simulink model "new_model"  (R2023a)
(part 1 of 4)
settings: Solver=VariableStepAuto  StartTime=0.0  StopTime=10.0  RelTol=1e-3
settings Model: Creator=owner  LastModifiedBy=owner

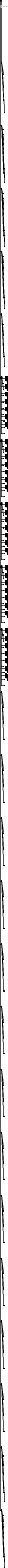
== system new_model ==
  SensorsInput : Inport
  Bus Selector:FreeSpacePerception:0 : BusSelector  OutputSignals=FreeSpacePerception:0.time,FreeSpacePerception:0.width,FreeSpacePerception:0.x,FreeSpacePerception:0.y
  Bus Selector:GNSS:0 : BusSelector  OutputSignals=GNSS:0.Timestamp,GNSS:0.Longitude,GNSS:0.Latitude,GNSS:0.Altitude,GNSS:0.Heading,GNSS:0.Velocity
  Bus Selector:IMU:0 : BusSelector  OutputSignals=IMU:0.Timestamp,IMU:0.ACC_X,IMU:0.ACC_Y,IMU:0.ACC_Z,IMU:0.Gyro_X,IMU:0.Gyro_Y,IMU:0.Gyro_Z,IMU:0.Yaw,IMU:0.Pitch,IMU:0.Roll
  Bus Selector:LaneInfoPerception:0 : BusSelector  OutputSignals=LaneInfoPerception:0.Timestamp,LaneInfoPerception:0.width,LaneInfoPerception:0.Lane_ID,LaneInfoPerception:0.Lane_Distance,LaneInfoPerception:0.Lane_Car_Distance_Left,LaneInfoPerception:0.Lane_Car_Distance_Right,LaneInfoPerception:0.Lane_Curvature,LaneInfoPerception:0.Lane_Coefficient_C0,LaneInfoPerception:0.Lane_Coefficient_C1,LaneInfoPerception:0.Lane_Coefficient_C2,LaneInfoPerception:0.Lane_Coefficient_C3,LaneInfoPerception:0.Lane_Class
  Bus Selector:ObjectPerception:0 : BusSelector  OutputSignals=ObjectPerception:0.Timestamp,ObjectPerception:0.width,ObjectPerception:0.OBJ_ID,ObjectPerception:0.OBJ_Class,ObjectPerception:0.OBJ_X,ObjectPerception:0.OBJ_Y,ObjectPerception:0.OBJ_Z,ObjectPerception:0.OBJ_Velocity,ObjectPerception:0.OBJ_Length,ObjectPerception:0.OBJ_Width,ObjectPerception:0.OBJ_Height
  Bus Selector:ParkingLotsPerception:0 : BusSelector  OutputSignals=ParkingLotsPerception:0.time,ParkingLotsPerception:0.width,ParkingLotsPerception:0.x1,ParkingLotsPerception:0.y1,ParkingLotsPerception:0.x2,ParkingLotsPerception:0.y2,ParkingLotsPerception:0.x3,ParkingLotsPerception:0.y3,ParkingLotsPerception:0.x4,ParkingLotsPerception:0.y4
  Bus Selector:RadarSensor:0 : BusSelector  OutputSignals=RadarSensor:0.time,RadarSensor:0.width,RadarSensor:0.OBJ_ID,RadarSensor:0.OBJ_Class,RadarSensor:0.OBJ_S_Azimuth,RadarSensor:0.OBJ_S_Elevation,RadarSensor:0.OBJ_S_Velocity,RadarSensor:0.OBJ_S_Range,RadarSensor:0.OBJ_RCS
  Bus Selector:RadarSensor:0_OBJ_Class_BS : BusSelector  OutputSignals=RadarSensor:0.OBJ_Class_1,RadarSensor:0.OBJ_Class_2,RadarSensor:0.OBJ_Class_3,RadarSensor:0.OBJ_Class_4,RadarSensor:0.OBJ_Class_5,RadarSensor:0.OBJ_Class_6,RadarSensor:0.OBJ_Class_7,RadarSensor:0.OBJ_Class_8,RadarSensor:0.OBJ_Class_9,RadarSensor:0.OBJ_Class_10,RadarSensor:0.OBJ_Class_11,RadarSensor:0.OBJ_Class_12,RadarSensor:0.OBJ_Class_13,RadarSensor:0.OBJ_Class_14,RadarSensor:0.OBJ_Class_15,RadarSensor:0.OBJ_Class_16,RadarSensor:0.OBJ_Class_17,RadarSensor:0.OBJ_Class_18,RadarSensor:0.OBJ_Class_19,RadarSensor:0.OBJ_Class_20,RadarSensor:0.OBJ_Class_21,RadarSensor:0.OBJ_Class_22,RadarSensor:0.OBJ_Class_23,RadarSensor:0.OBJ_Class_24,RadarSensor:0.OBJ_Class_25,RadarSensor:0.OBJ_Class_26,RadarSensor:0.OBJ_Class_27,RadarSensor:0.OBJ_Class_28,RadarSensor:0.OBJ_Class_29,RadarSensor:0.OBJ_Class_30,RadarSensor:0.OBJ_Class_31,RadarSensor:0.OBJ_Class_32,RadarSensor:0.OBJ_Class_33,RadarSensor:0.OBJ_Class_34,RadarSensor:0.OBJ_Class_35,RadarSensor:0.OBJ_Class_36,RadarSensor:0.OBJ_Class_37,RadarSensor:0.OBJ_Class_38,RadarSensor:0.OBJ_Class_39,RadarSensor:0.OBJ_Class_40,RadarSensor:0.OBJ_Class_41,RadarSensor:0.OBJ_Class_42,RadarSensor:0.OBJ_Class_43,RadarSensor:0.OBJ_Class_44,RadarSensor:0.OBJ_Class_45,RadarSensor:0.OBJ_Class_46,RadarSensor:0.OBJ_Class_47,RadarSensor:0.OBJ_Class_48,RadarSensor:0.OBJ_Class_49,RadarSensor:0.OBJ_Class_50,RadarSensor:0.OBJ_Class_51,RadarSensor:0.OBJ_Class_52,RadarSensor:0.OBJ_Class_53,RadarSensor:0.OBJ_Class_54,RadarSensor:0.OBJ_Class_55,RadarSensor:0.OBJ_Class_56,RadarSensor:0.OBJ_Class_57,RadarSensor:0.OBJ_Class_58,RadarSensor:0.OBJ_Class_59,RadarSensor:0.OBJ_Class_60,RadarSensor:0.OBJ_Class_61,RadarSensor:0.OBJ_Class_62,RadarSensor:0.OBJ_Class_63,RadarSensor:0.OBJ_Class_64
  Bus Selector:RadarSensor:0_OBJ_ID_BS : BusSelector  OutputSignals=RadarSensor:0.OBJ_ID_1,RadarSensor:0.OBJ_ID_2,RadarSensor:0.OBJ_ID_3,RadarSensor:0.OBJ_ID_4,RadarSensor:0.OBJ_ID_5,RadarSensor:0.OBJ_ID_6,RadarSensor:0.OBJ_ID_7,RadarSensor:0.OBJ_ID_8,RadarSensor:0.OBJ_ID_9,RadarSensor:0.OBJ_ID_10,RadarSensor:0.OBJ_ID_11,RadarSensor:0.OBJ_ID_12,RadarSensor:0.OBJ_ID_13,RadarSensor:0.OBJ_ID_14,RadarSensor:0.OBJ_ID_15,RadarSensor:0.OBJ_ID_16,RadarSensor:0.OBJ_ID_17,RadarSensor:0.OBJ_ID_18,RadarSensor:0.OBJ_ID_19,RadarSensor:0.OBJ_ID_20,RadarSensor:0.OBJ_ID_21,RadarSensor:0.OBJ_ID_22,RadarSensor:0.OBJ_ID_23,RadarSensor:0.OBJ_ID_24,RadarSensor:0.OBJ_ID_25,RadarSensor:0.OBJ_ID_26,RadarSensor:0.OBJ_ID_27,RadarSensor:0.OBJ_ID_28,RadarSensor:0.OBJ_ID_29,RadarSensor:0.OBJ_ID_30,RadarSensor:0.OBJ_ID_31,RadarSensor:0.OBJ_ID_32,RadarSensor:0.OBJ_ID_33,RadarSensor:0.OBJ_ID_34,RadarSensor:0.OBJ_ID_35,RadarSensor:0.OBJ_ID_36,RadarSensor:0.OBJ_ID_37,RadarSensor:0.OBJ_ID_38,RadarSensor:0.OBJ_ID_39,RadarSensor:0.OBJ_ID_40,RadarSensor:0.OBJ_ID_41,RadarSensor:0.OBJ_ID_42,RadarSensor:0.OBJ_ID_43,RadarSensor:0.OBJ_ID_44,RadarSensor:0.OBJ_ID_45,RadarSensor:0.OBJ_ID_46,RadarSensor:0.OBJ_ID_47,RadarSensor:0.OBJ_ID_48,RadarSensor:0.OBJ_ID_49,RadarSensor:0.OBJ_ID_50,RadarSensor:0.OBJ_ID_51,RadarSensor:0.OBJ_ID_52,RadarSensor:0.OBJ_ID_53,RadarSensor:0.OBJ_ID_54,RadarSensor:0.OBJ_ID_55,RadarSensor:0.OBJ_ID_56,RadarSensor:0.OBJ_ID_57,RadarSensor:0.OBJ_ID_58,RadarSensor:0.OBJ_ID_59,RadarSensor:0.OBJ_ID_60,RadarSensor:0.OBJ_ID_61,RadarSensor:0.OBJ_ID_62,RadarSensor:0.OBJ_ID_63,RadarSensor:0.OBJ_ID_64
  Bus Selector:RadarSensor:0_OBJ_RCS_BS : BusSelector  OutputSignals=RadarSensor:0.OBJ_RCS_1,RadarSensor:0.OBJ_RCS_2,RadarSensor:0.OBJ_RCS_3,RadarSensor:0.OBJ_RCS_4,RadarSensor:0.OBJ_RCS_5,RadarSensor:0.OBJ_RCS_6,RadarSensor:0.OBJ_RCS_7,RadarSensor:0.OBJ_RCS_8,RadarSensor:0.OBJ_RCS_9,RadarSensor:0.OBJ_RCS_10,RadarSensor:0.OBJ_RCS_11,RadarSensor:0.OBJ_RCS_12,RadarSensor:0.OBJ_RCS_13,RadarSensor:0.OBJ_RCS_14,RadarSensor:0.OBJ_RCS_15,RadarSensor:0.OBJ_RCS_16,RadarSensor:0.OBJ_RCS_17,RadarSensor:0.OBJ_RCS_18,RadarSensor:0.OBJ_RCS_19,RadarSensor:0.OBJ_RCS_20,RadarSensor:0.OBJ_RCS_21,RadarSensor:0.OBJ_RCS_22,RadarSensor:0.OBJ_RCS_23,RadarSensor:0.OBJ_RCS_24,RadarSensor:0.OBJ_RCS_25,RadarSensor:0.OBJ_RCS_26,RadarSensor:0.OBJ_RCS_27,RadarSensor:0.OBJ_RCS_28,RadarSensor:0.OBJ_RCS_29,RadarSensor:0.OBJ_RCS_30,RadarSensor:0.OBJ_RCS_31,RadarSensor:0.OBJ_RCS_32,RadarSensor:0.OBJ_RCS_33,RadarSensor:0.OBJ_RCS_34,RadarSensor:0.OBJ_RCS_35,RadarSensor:0.OBJ_RCS_36,RadarSensor:0.OBJ_RCS_37,RadarSensor:0.OBJ_RCS_38,RadarSensor:0.OBJ_RCS_39,RadarSensor:0.OBJ_RCS_40,RadarSensor:0.OBJ_RCS_41,RadarSensor:0.OBJ_RCS_42,RadarSensor:0.OBJ_RCS_43,RadarSensor:0.OBJ_RCS_44,RadarSensor:0.OBJ_RCS_45,RadarSensor:0.OBJ_RCS_46,RadarSensor:0.OBJ_RCS_47,RadarSensor:0.OBJ_RCS_48,RadarSensor:0.OBJ_RCS_49,RadarSensor:0.OBJ_RCS_50,RadarSensor:0.OBJ_RCS_51,RadarSensor:0.OBJ_RCS_52,RadarSensor:0.OBJ_RCS_53,RadarSensor:0.OBJ_RCS_54,RadarSensor:0.OBJ_RCS_55,RadarSensor:0.OBJ_RCS_56,RadarSensor:0.OBJ_RCS_57,RadarSensor:0.OBJ_RCS_58,RadarSensor:0.OBJ_RCS_59,RadarSensor:0.OBJ_RCS_60,RadarSensor:0.OBJ_RCS_61,RadarSensor:0.OBJ_RCS_62,RadarSensor:0.OBJ_RCS_63,RadarSensor:0.OBJ_RCS_64
  Bus Selector:RadarSensor:0_OBJ_S_Azimuth_BS : BusSelector  OutputSignals=RadarSensor:0.OBJ_S_Azimuth_1,RadarSensor:0.OBJ_S_Azimuth_2,RadarSensor:0.OBJ_S_Azimuth_3,RadarSensor:0.OBJ_S_Azimuth_4,RadarSensor:0.OBJ_S_Azimuth_5,RadarSensor:0.OBJ_S_Azimuth_6,RadarSensor:0.OBJ_S_Azimuth_7,RadarSensor:0.OBJ_S_Azimuth_8,RadarSensor:0.OBJ_S_Azimuth_9,RadarSensor:0.OBJ_S_Azimuth_10,RadarSensor:0.OBJ_S_Azimuth_11,RadarSensor:0.OBJ_S_Azimuth_12,RadarSensor:0.OBJ_S_Azimuth_13,RadarSensor:0.OBJ_S_Azimuth_14,RadarSensor:0.OBJ_S_Azimuth_15,RadarSensor:0.OBJ_S_Azimuth_16,RadarSensor:0.OBJ_S_Azimuth_17,RadarSensor:0.OBJ_S_Azimuth_18,RadarSensor:0.OBJ_S_Azimuth_19,RadarSensor:0.OBJ_S_Azimuth_20,RadarSensor:0.OBJ_S_Azimuth_21,RadarSensor:0.OBJ_S_Azimuth_22,RadarSensor:0.OBJ_S_Azimuth_23,RadarSensor:0.OBJ_S_Azimuth_24,RadarSensor:0.OBJ_S_Azimuth_25,RadarSensor:0.OBJ_S_Azimuth_26,RadarSensor:0.OBJ_S_Azimuth_27,RadarSensor:0.OBJ_S_Azimuth_28,RadarSensor:0.OBJ_S_Azimuth_29,RadarSensor:0.OBJ_S_Azimuth_30,RadarSensor:0.OBJ_S_Azimuth_31,RadarSensor:0.OBJ_S_Azimuth_32,RadarSensor:0.OBJ_S_Azimuth_33,RadarSensor:0.OBJ_S_Azimuth_34,RadarSensor:0.OBJ_S_Azimuth_35,RadarSensor:0.OBJ_S_Azimuth_36,RadarSensor:0.OBJ_S_Azimuth_37,RadarSensor:0.OBJ_S_Azimuth_38,RadarSensor:0.OBJ_S_Azimuth_39,RadarSensor:0.OBJ_S_Azimuth_40,RadarSensor:0.OBJ_S_Azimuth_41,RadarSensor:0.OBJ_S_Azimuth_42,RadarSensor:0.OBJ_S_Azimuth_43,RadarSensor:0.OBJ_S_Azimuth_44,RadarSensor:0.OBJ_S_Azimuth_45,RadarSensor:0.OBJ_S_Azimuth_46,RadarSensor:0.OBJ_S_Azimuth_47,RadarSensor:0.OBJ_S_Azimuth_48,RadarSensor:0.OBJ_S_Azimuth_49,RadarSensor:0.OBJ_S_Azimuth_50,RadarSensor:0.OBJ_S_Azimuth_51,RadarSensor:0.OBJ_S_Azimuth_52,RadarSensor:0.OBJ_S_Azimuth_53,RadarSensor:0.OBJ_S_Azimuth_54,RadarSensor:0.OBJ_S_Azimuth_55,RadarSensor:0.OBJ_S_Azimuth_56,RadarSensor:0.OBJ_S_Azimuth_57,RadarSensor:0.OBJ_S_Azimuth_58,RadarSensor:0.OBJ_S_Azimuth_59,RadarSensor:0.OBJ_S_Azimuth_60,RadarSensor:0.OBJ_S_Azimuth_61,RadarSensor:0.OBJ_S_Azimuth_62,RadarSensor:0.OBJ_S_Azimuth_63,RadarSensor:0.OBJ_S_Azimuth_64
  Bus Selector:RadarSensor:0_OBJ_S_Elevation_BS : BusSelector  OutputSignals=RadarSensor:0.OBJ_S_Elevation_1,RadarSensor:0.OBJ_S_Elevation_2,RadarSensor:0.OBJ_S_Elevation_3,RadarSensor:0.OBJ_S_Elevation_4,RadarSensor:0.OBJ_S_Elevation_5,RadarSensor:0.OBJ_S_Elevation_6,RadarSensor:0.OBJ_S_Elevation_7,RadarSensor:0.OBJ_S_Elevation_8,RadarSensor:0.OBJ_S_Elevation_9,RadarSensor:0.OBJ_S_Elevation_10,RadarSensor:0.OBJ_S_Elevation_11,RadarSensor:0.OBJ_S_Elevation_12,RadarSensor:0.OBJ_S_Elevation_13,RadarSensor:0.OBJ_S_Elevation_14,RadarSensor:0.OBJ_S_Elevation_15,RadarSensor:0.OBJ_S_Elevation_16,RadarSensor:0.OBJ_S_Elevation_17,RadarSensor:0.OBJ_S_Elevation_18,RadarSensor:0.OBJ_S_Elevation_19,RadarSensor:0.OBJ_S_Elevation_20,RadarSensor:0.OBJ_S_Elevation_21,RadarSensor:0.OBJ_S_Elevation_22,RadarSensor:0.OBJ_S_Elevation_23,RadarSensor:0.OBJ_S_Elevation_24,RadarSensor:0.OBJ_S_Elevation_25,RadarSensor:0.OBJ_S_Elevation_26,RadarSensor:0.OBJ_S_Elevation_27,RadarSensor:0.OBJ_S_Elevation_28,RadarSensor:0.OBJ_S_Elevation_29,RadarSensor:0.OBJ_S_Elevation_30,RadarSensor:0.OBJ_S_Elevation_31,RadarSensor:0.OBJ_S_Elevation_32,RadarSensor:0.OBJ_S_Elevation_33,RadarSensor:0.OBJ_S_Elevation_34,RadarSensor:0.OBJ_S_Elevation_35,RadarSensor:0.OBJ_S_Elevation_36,RadarSensor:0.OBJ_S_Elevation_37,RadarSensor:0.OBJ_S_Elevation_38,RadarSensor:0.OBJ_S_Elevation_39,RadarSensor:0.OBJ_S_Elevation_40,RadarSensor:0.OBJ_S_Elevation_41,RadarSensor:0.OBJ_S_Elevation_42,RadarSensor:0.OBJ_S_Elevation_43,RadarSensor:0.OBJ_S_Elevation_44,RadarSensor:0.OBJ_S_Elevation_45,RadarSensor:0.OBJ_S_Elevation_46,RadarSensor:0.OBJ_S_Elevation_47,RadarSensor:0.OBJ_S_Elevation_48,RadarSensor:0.OBJ_S_Elevation_49,RadarSensor:0.OBJ_S_Elevation_50,RadarSensor:0.OBJ_S_Elevation_51,RadarSensor:0.OBJ_S_Elevation_52,RadarSensor:0.OBJ_S_Elevation_53,RadarSensor:0.OBJ_S_Elevation_54,RadarSensor:0.OBJ_S_Elevation_55,RadarSensor:0.OBJ_S_Elevation_56,RadarSensor:0.OBJ_S_Elevation_57,RadarSensor:0.OBJ_S_Elevation_58,RadarSensor:0.OBJ_S_Elevation_59,RadarSensor:0.OBJ_S_Elevation_60,RadarSensor:0.OBJ_S_Elevation_61,RadarSensor:0.OBJ_S_Elevation_62,RadarSensor:0.OBJ_S_Elevation_63,RadarSensor:0.OBJ_S_Elevation_64
  Bus Selector:RadarSensor:0_OBJ_S_Range_BS : BusSelector  OutputSignals=RadarSensor:0.OBJ_S_Range_1,RadarSensor:0.OBJ_S_Range_2,RadarSensor:0.OBJ_S_Range_3,RadarSensor:0.OBJ_S_Range_4,RadarSensor:0.OBJ_S_Range_5,RadarSensor:0.OBJ_S_Range_6,RadarSensor:0.OBJ_S_Range_7,RadarSensor:0.OBJ_S_Range_8,RadarSensor:0.OBJ_S_Range_9,RadarSensor:0.OBJ_S_Range_10,RadarSensor:0.OBJ_S_Range_11,RadarSensor:0.OBJ_S_Range_12,RadarSensor:0.OBJ_S_Range_13,RadarSensor:0.OBJ_S_Range_14,RadarSensor:0.OBJ_S_Range_15,RadarSensor:0.OBJ_S_Range_16,RadarSensor:0.OBJ_S_Range_17,RadarSensor:0.OBJ_S_Range_18,RadarSensor:0.OBJ_S_Range_19,RadarSensor:0.OBJ_S_Range_20,RadarSensor:0.OBJ_S_Range_21,RadarSensor:0.OBJ_S_Range_22,RadarSensor:0.OBJ_S_Range_23,RadarSensor:0.OBJ_S_Range_24,RadarSensor:0.OBJ_S_Range_25,RadarSensor:0.OBJ_S_Range_26,RadarSensor:0.OBJ_S_Range_27,RadarSensor:0.OBJ_S_Range_28,RadarSensor:0.OBJ_S_Range_29,RadarSensor:0.OBJ_S_Range_30,RadarSensor:0.OBJ_S_Range_31,RadarSensor:0.OBJ_S_Range_32,RadarSensor:0.OBJ_S_Range_33,RadarSensor:0.OBJ_S_Range_34,RadarSensor:0.OBJ_S_Range_35,RadarSensor:0.OBJ_S_Range_36,RadarSensor:0.OBJ_S_Range_37,RadarSensor:0.OBJ_S_Range_38,RadarSensor:0.OBJ_S_Range_39,RadarSensor:0.OBJ_S_Range_40,RadarSensor:0.OBJ_S_Range_41,RadarSensor:0.OBJ_S_Range_42,RadarSensor:0.OBJ_S_Range_43,RadarSensor:0.OBJ_S_Range_44,RadarSensor:0.OBJ_S_Range_45,RadarSensor:0.OBJ_S_Range_46,RadarSensor:0.OBJ_S_Range_47,RadarSensor:0.OBJ_S_Range_48,RadarSensor:0.OBJ_S_Range_49,RadarSensor:0.OBJ_S_Range_50,RadarSensor:0.OBJ_S_Range_51,RadarSensor:0.OBJ_S_Range_52,RadarSensor:0.OBJ_S_Range_53,RadarSensor:0.OBJ_S_Range_54,RadarSensor:0.OBJ_S_Range_55,RadarSensor:0.OBJ_S_Range_56,RadarSensor:0.OBJ_S_Range_57,RadarSensor:0.OBJ_S_Range_58,RadarSensor:0.OBJ_S_Range_59,RadarSensor:0.OBJ_S_Range_60,RadarSensor:0.OBJ_S_Range_61,RadarSensor:0.OBJ_S_Range_62,RadarSensor:0.OBJ_S_Range_63,RadarSensor:0.OBJ_S_Range_64
  Bus Selector:RadarSensor:0_OBJ_S_Velocity_BS : BusSelector  OutputSignals=RadarSensor:0.OBJ_S_Velocity_1,RadarSensor:0.OBJ_S_Velocity_2,RadarSensor:0.OBJ_S_Velocity_3,RadarSensor:0.OBJ_S_Velocity_4,RadarSensor:0.OBJ_S_Velocity_5,RadarSensor:0.OBJ_S_Velocity_6,RadarSensor:0.OBJ_S_Velocity_7,RadarSensor:0.OBJ_S_Velocity_8,RadarSensor:0.OBJ_S_Velocity_9,RadarSensor:0.OBJ_S_Velocity_10,RadarSensor:0.OBJ_S_Velocity_11,RadarSensor:0.OBJ_S_Velocity_12,RadarSensor:0.OBJ_S_Velocity_13,RadarSensor:0.OBJ_S_Velocity_14,RadarSensor:0.OBJ_S_Velocity_15,RadarSensor:0.OBJ_S_Velocity_16,RadarSensor:0.OBJ_S_Velocity_17,RadarSensor:0.OBJ_S_Velocity_18,RadarSensor:0.OBJ_S_Velocity_19,RadarSensor:0.OBJ_S_Velocity_20,RadarSensor:0.OBJ_S_Velocity_21,RadarSensor:0.OBJ_S_Velocity_22,RadarSensor:0.OBJ_S_Velocity_23,RadarSensor:0.OBJ_S_Velocity_24,RadarSensor:0.OBJ_S_Velocity_25,RadarSensor:0.OBJ_S_Velocity_26,RadarSensor:0.OBJ_S_Velocity_27,RadarSensor:0.OBJ_S_Velocity_28,RadarSensor:0.OBJ_S_Velocity_29,RadarSensor:0.OBJ_S_Velocity_30,RadarSensor:0.OBJ_S_Velocity_31,RadarSensor:0.OBJ_S_Velocity_32,RadarSensor:0.OBJ_S_Velocity_33,RadarSensor:0.OBJ_S_Velocity_34,RadarSensor:0.OBJ_S_Velocity_35,RadarSensor:0.OBJ_S_Velocity_36,RadarSensor:0.OBJ_S_Velocity_37,RadarSensor:0.OBJ_S_Velocity_38,RadarSensor:0.OBJ_S_Velocity_39,RadarSensor:0.OBJ_S_Velocity_40,RadarSensor:0.OBJ_S_Velocity_41,RadarSensor:0.OBJ_S_Velocity_42,RadarSensor:0.OBJ_S_Velocity_43,RadarSensor:0.OBJ_S_Velocity_44,RadarSensor:0.OBJ_S_Velocity_45,RadarSensor:0.OBJ_S_Velocity_46,RadarSensor:0.OBJ_S_Velocity_47,RadarSensor:0.OBJ_S_Velocity_48,RadarSensor:0.OBJ_S_Velocity_49,RadarSensor:0.OBJ_S_Velocity_50,RadarSensor:0.OBJ_S_Velocity_51,RadarSensor:0.OBJ_S_Velocity_52,RadarSensor:0.OBJ_S_Velocity_53,RadarSensor:0.OBJ_S_Velocity_54,RadarSensor:0.OBJ_S_Velocity_55,RadarSensor:0.OBJ_S_Velocity_56,RadarSensor:0.OBJ_S_Velocity_57,RadarSensor:0.OBJ_S_Velocity_58,RadarSensor:0.OBJ_S_Velocity_59,RadarSensor:0.OBJ_S_Velocity_60,RadarSensor:0.OBJ_S_Velocity_61,RadarSensor:0.OBJ_S_Velocity_62,RadarSensor:0.OBJ_S_Velocity_63,RadarSensor:0.OBJ_S_Velocity_64
  Bus Selector:RadarSensor:1 : BusSelector  OutputSignals=RadarSensor:1.time,RadarSensor:1.width,RadarSensor:1.OBJ_ID,RadarSensor:1.OBJ_Class,RadarSensor:1.OBJ_S_Azimuth,RadarSensor:1.OBJ_S_Elevation,RadarSensor:1.OBJ_S_Velocity,RadarSensor:1.OBJ_S_Range,RadarSensor:1.OBJ_RCS
  Bus Selector:RadarSensor:1_OBJ_Class_BS : BusSelector  OutputSignals=RadarSensor:1.OBJ_Class_1,RadarSensor:1.OBJ_Class_2,RadarSensor:1.OBJ_Class_3,RadarSensor:1.OBJ_Class_4,RadarSensor:1.OBJ_Class_5,RadarSensor:1.OBJ_Class_6,RadarSensor:1.OBJ_Class_7,RadarSensor:1.OBJ_Class_8,RadarSensor:1.OBJ_Class_9,RadarSensor:1.OBJ_Class_10,RadarSensor:1.OBJ_Class_11,RadarSensor:1.OBJ_Class_12,RadarSensor:1.OBJ_Class_13,RadarSensor:1.OBJ_Class_14,RadarSensor:1.OBJ_Class_15,RadarSensor:1.OBJ_Class_16,RadarSensor:1.OBJ_Class_17,RadarSensor:1.OBJ_Class_18,RadarSensor:1.OBJ_Class_19,RadarSensor:1.OBJ_Class_20,RadarSensor:1.OBJ_Class_21,RadarSensor:1.OBJ_Class_22,RadarSensor:1.OBJ_Class_23,RadarSensor:1.OBJ_Class_24,RadarSensor:1.OBJ_Class_25,RadarSensor:1.OBJ_Class_26,RadarSensor:1.OBJ_Class_27,RadarSensor:1.OBJ_Class_28,RadarSensor:1.OBJ_Class_29,RadarSensor:1.OBJ_Class_30,RadarSensor:1.OBJ_Class_31,RadarSensor:1.OBJ_Class_32,RadarSensor:1.OBJ_Class_33,RadarSensor:1.OBJ_Class_34,RadarSensor:1.OBJ_Class_35,RadarSensor:1.OBJ_Class_36,RadarSensor:1.OBJ_Class_37,RadarSensor:1.OBJ_Class_38,RadarSensor:1.OBJ_Class_39,RadarSensor:1.OBJ_Class_40,RadarSensor:1.OBJ_Class_41,RadarSensor:1.OBJ_Class_42,RadarSensor:1.OBJ_Class_43,RadarSensor:1.OBJ_Class_44,RadarSensor:1.OBJ_Class_45,RadarSensor:1.OBJ_Class_46,RadarSensor:1.OBJ_Class_47,RadarSensor:1.OBJ_Class_48,RadarSensor:1.OBJ_Class_49,RadarSensor:1.OBJ_Class_50,RadarSensor:1.OBJ_Class_51,RadarSensor:1.OBJ_Class_52,RadarSensor:1.OBJ_Class_53,RadarSensor:1.OBJ_Class_54,RadarSensor:1.OBJ_Class_55,RadarSensor:1.OBJ_Class_56,RadarSensor:1.OBJ_Class_57,RadarSensor:1.OBJ_Class_58,RadarSensor:1.OBJ_Class_59,RadarSensor:1.OBJ_Class_60,RadarSensor:1.OBJ_Class_61,RadarSensor:1.OBJ_Class_62,RadarSensor:1.OBJ_Class_63,RadarSensor:1.OBJ_Class_64
  Bus Selector:RadarSensor:1_OBJ_ID_BS : BusSelector  OutputSignals=RadarSensor:1.OBJ_ID_1,RadarSensor:1.OBJ_ID_2,RadarSensor:1.OBJ_ID_3,RadarSensor:1.OBJ_ID_4,RadarSensor:1.OBJ_ID_5,RadarSensor:1.OBJ_ID_6,RadarSensor:1.OBJ_ID_7,RadarSensor:1.OBJ_ID_8,RadarSensor:1.OBJ_ID_9,RadarSensor:1.OBJ_ID_10,RadarSensor:1.OBJ_ID_11,RadarSensor:1.OBJ_ID_12,RadarSensor:1.OBJ_ID_13,RadarSensor:1.OBJ_ID_14,RadarSensor:1.OBJ_ID_15,RadarSensor:1.OBJ_ID_16,RadarSensor:1.OBJ_ID_17,RadarSensor:1.OBJ_ID_18,RadarSensor:1.OBJ_ID_19,RadarSensor:1.OBJ_ID_20,RadarSensor:1.OBJ_ID_21,RadarSensor:1.OBJ_ID_22,RadarSensor:1.OBJ_ID_23,RadarSensor:1.OBJ_ID_24,RadarSensor:1.OBJ_ID_25,RadarSensor:1.OBJ_ID_26,RadarSensor:1.OBJ_ID_27,RadarSensor:1.OBJ_ID_28,RadarSensor:1.OBJ_ID_29,RadarSensor:1.OBJ_ID_30,RadarSensor:1.OBJ_ID_31,RadarSensor:1.OBJ_ID_32,RadarSensor:1.OBJ_ID_33,RadarSensor:1.OBJ_ID_34,RadarSensor:1.OBJ_ID_35,RadarSensor:1.OBJ_ID_36,RadarSensor:1.OBJ_ID_37,RadarSensor:1.OBJ_ID_38,RadarSensor:1.OBJ_ID_39,RadarSensor:1.OBJ_ID_40,RadarSensor:1.OBJ_ID_41,RadarSensor:1.OBJ_ID_42,RadarSensor:1.OBJ_ID_43,RadarSensor:1.OBJ_ID_44,RadarSensor:1.OBJ_ID_45,RadarSensor:1.OBJ_ID_46,RadarSensor:1.OBJ_ID_47,RadarSensor:1.OBJ_ID_48,RadarSensor:1.OBJ_ID_49,RadarSensor:1.OBJ_ID_50,RadarSensor:1.OBJ_ID_51,RadarSensor:1.OBJ_ID_52,RadarSensor:1.OBJ_ID_53,RadarSensor:1.OBJ_ID_54,RadarSensor:1.OBJ_ID_55,RadarSensor:1.OBJ_ID_56,RadarSensor:1.OBJ_ID_57,RadarSensor:1.OBJ_ID_58,RadarSensor:1.OBJ_ID_59,RadarSensor:1.OBJ_ID_60,RadarSensor:1.OBJ_ID_61,RadarSensor:1.OBJ_ID_62,RadarSensor:1.OBJ_ID_63,RadarSensor:1.OBJ_ID_64
  Bus Selector:RadarSensor:1_OBJ_RCS_BS : BusSelector  OutputSignals=RadarSensor:1.OBJ_RCS_1,RadarSensor:1.OBJ_RCS_2,RadarSensor:1.OBJ_RCS_3,RadarSensor:1.OBJ_RCS_4,RadarSensor:1.OBJ_RCS_5,RadarSensor:1.OBJ_RCS_6,RadarSensor:1.OBJ_RCS_7,RadarSensor:1.OBJ_RCS_8,RadarSensor:1.OBJ_RCS_9,RadarSensor:1.OBJ_RCS_10,RadarSensor:1.OBJ_RCS_11,RadarSensor:1.OBJ_RCS_12,RadarSensor:1.OBJ_RCS_13,RadarSensor:1.OBJ_RCS_14,RadarSensor:1.OBJ_RCS_15,RadarSensor:1.OBJ_RCS_16,RadarSensor:1.OBJ_RCS_17,RadarSensor:1.OBJ_RCS_18,RadarSensor:1.OBJ_RCS_19,RadarSensor:1.OBJ_RCS_20,RadarSensor:1.OBJ_RCS_21,RadarSensor:1.OBJ_RCS_22,RadarSensor:1.OBJ_RCS_23,RadarSensor:1.OBJ_RCS_24,RadarSensor:1.OBJ_RCS_25,RadarSensor:1.OBJ_RCS_26,RadarSensor:1.OBJ_RCS_27,RadarSensor:1.OBJ_RCS_28,RadarSensor:1.OBJ_RCS_29,RadarSensor:1.OBJ_RCS_30,RadarSensor:1.OBJ_RCS_31,RadarSensor:1.OBJ_RCS_32,RadarSensor:1.OBJ_RCS_33,RadarSensor:1.OBJ_RCS_34,RadarSensor:1.OBJ_RCS_35,RadarSensor:1.OBJ_RCS_36,RadarSensor:1.OBJ_RCS_37,RadarSensor:1.OBJ_RCS_38,RadarSensor:1.OBJ_RCS_39,RadarSensor:1.OBJ_RCS_40,RadarSensor:1.OBJ_RCS_41,RadarSensor:1.OBJ_RCS_42,RadarSensor:1.OBJ_RCS_43,RadarSensor:1.OBJ_RCS_44,RadarSensor:1.OBJ_RCS_45,RadarSensor:1.OBJ_RCS_46,RadarSensor:1.OBJ_RCS_47,RadarSensor:1.OBJ_RCS_48,RadarSensor:1.OBJ_RCS_49,RadarSensor:1.OBJ_RCS_50,RadarSensor:1.OBJ_RCS_51,RadarSensor:1.OBJ_RCS_52,RadarSensor:1.OBJ_RCS_53,RadarSensor:1.OBJ_RCS_54,RadarSensor:1.OBJ_RCS_55,RadarSensor:1.OBJ_RCS_56,RadarSensor:1.OBJ_RCS_57,RadarSensor:1.OBJ_RCS_58,RadarSensor:1.OBJ_RCS_59,RadarSensor:1.OBJ_RCS_60,RadarSensor:1.OBJ_RCS_61,RadarSensor:1.OBJ_RCS_62,RadarSensor:1.OBJ_RCS_63,RadarSensor:1.OBJ_RCS_64
  Bus Selector:RadarSensor:1_OBJ_S_Azimuth_BS : BusSelector  OutputSignals=RadarSensor:1.OBJ_S_Azimuth_1,RadarSensor:1.OBJ_S_Azimuth_2,RadarSensor:1.OBJ_S_Azimuth_3,RadarSensor:1.OBJ_S_Azimuth_4,RadarSensor:1.OBJ_S_Azimuth_5,RadarSensor:1.OBJ_S_Azimuth_6,RadarSensor:1.OBJ_S_Azimuth_7,RadarSensor:1.OBJ_S_Azimuth_8,RadarSensor:1.OBJ_S_Azimuth_9,RadarSensor:1.OBJ_S_Azimuth_10,RadarSensor:1.OBJ_S_Azimuth_11,RadarSensor:1.OBJ_S_Azimuth_12,RadarSensor:1.OBJ_S_Azimuth_13,RadarSensor:1.OBJ_S_Azimuth_14,RadarSensor:1.OBJ_S_Azimuth_15,RadarSensor:1.OBJ_S_Azimuth_16,RadarSensor:1.OBJ_S_Azimuth_17,RadarSensor:1.OBJ_S_Azimuth_18,RadarSensor:1.OBJ_S_Azimuth_19,RadarSensor:1.OBJ_S_Azimuth_20,RadarSensor:1.OBJ_S_Azimuth_21,RadarSensor:1.OBJ_S_Azimuth_22,RadarSensor:1.OBJ_S_Azimuth_23,RadarSensor:1.OBJ_S_Azimuth_24,RadarSensor:1.OBJ_S_Azimuth_25,RadarSensor:1.OBJ_S_Azimuth_26,RadarSensor:1.OBJ_S_Azimuth_27,RadarSensor:1.OBJ_S_Azimuth_28,RadarSensor:1.OBJ_S_Azimuth_29,RadarSensor:1.OBJ_S_Azimuth_30,RadarSensor:1.OBJ_S_Azimuth_31,RadarSensor:1.OBJ_S_Azimuth_32,RadarSensor:1.OBJ_S_Azimuth_33,RadarSensor:1.OBJ_S_Azimuth_34,RadarSensor:1.OBJ_S_Azimuth_35,RadarSensor:1.OBJ_S_Azimuth_36,RadarSensor:1.OBJ_S_Azimuth_37,RadarSensor:1.OBJ_S_Azimuth_38,RadarSensor:1.OBJ_S_Azimuth_39,RadarSensor:1.OBJ_S_Azimuth_40,RadarSensor:1.OBJ_S_Azimuth_41,RadarSensor:1.OBJ_S_Azimuth_42,RadarSensor:1.OBJ_S_Azimuth_43,RadarSensor:1.OBJ_S_Azimuth_44,RadarSensor:1.OBJ_S_Azimuth_45,RadarSensor:1.OBJ_S_Azimuth_46,RadarSensor:1.OBJ_S_Azimuth_47,RadarSensor:1.OBJ_S_Azimuth_48,RadarSensor:1.OBJ_S_Azimuth_49,RadarSensor:1.OBJ_S_Azimuth_50,RadarSensor:1.OBJ_S_Azimuth_51,RadarSensor:1.OBJ_S_Azimuth_52,RadarSensor:1.OBJ_S_Azimuth_53,RadarSensor:1.OBJ_S_Azimuth_54,RadarSensor:1.OBJ_S_Azimuth_55,RadarSensor:1.OBJ_S_Azimuth_56,RadarSensor:1.OBJ_S_Azimuth_57,RadarSensor:1.OBJ_S_Azimuth_58,RadarSensor:1.OBJ_S_Azimuth_59,RadarSensor:1.OBJ_S_Azimuth_60,RadarSensor:1.OBJ_S_Azimuth_61,RadarSensor:1.OBJ_S_Azimuth_62,RadarSensor:1.OBJ_S_Azimuth_63,RadarSensor:1.OBJ_S_Azimuth_64
  Bus Selector:RadarSensor:1_OBJ_S_Elevation_BS : BusSelector  OutputSignals=RadarSensor:1.OBJ_S_Elevation_1,RadarSensor:1.OBJ_S_Elevation_2,RadarSensor:1.OBJ_S_Elevation_3,RadarSensor:1.OBJ_S_Elevation_4,RadarSensor:1.OBJ_S_Elevation_5,RadarSensor:1.OBJ_S_Elevation_6,RadarSensor:1.OBJ_S_Elevation_7,RadarSensor:1.OBJ_S_Elevation_8,RadarSensor:1.OBJ_S_Elevation_9,RadarSensor:1.OBJ_S_Elevation_10,RadarSensor:1.OBJ_S_Elevation_11,RadarSensor:1.OBJ_S_Elevation_12,RadarSensor:1.OBJ_S_Elevation_13,RadarSensor:1.OBJ_S_Elevation_14,RadarSensor:1.OBJ_S_Elevation_15,RadarSensor:1.OBJ_S_Elevation_16,RadarSensor:1.OBJ_S_Elevation_17,RadarSensor:1.OBJ_S_Elevation_18,RadarSensor:1.OBJ_S_Elevation_19,RadarSensor:1.OBJ_S_Elevation_20,RadarSensor:1.OBJ_S_Elevation_21,RadarSensor:1.OBJ_S_Elevation_22,RadarSensor:1.OBJ_S_Elevation_23,RadarSensor:1.OBJ_S_Elevation_24,RadarSensor:1.OBJ_S_Elevation_25,RadarSensor:1.OBJ_S_Elevation_26,RadarSensor:1.OBJ_S_Elevation_27,RadarSensor:1.OBJ_S_Elevation_28,RadarSensor:1.OBJ_S_Elevation_29,RadarSensor:1.OBJ_S_Elevation_30,RadarSensor:1.OBJ_S_Elevation_31,RadarSensor:1.OBJ_S_Elevation_32,RadarSensor:1.OBJ_S_Elevation_33,RadarSensor:1.OBJ_S_Elevation_34,RadarSensor:1.OBJ_S_Elevation_35,RadarSensor:1.OBJ_S_Elevation_36,RadarSensor:1.OBJ_S_Elevation_37,RadarSensor:1.OBJ_S_Elevation_38,RadarSensor:1.OBJ_S_Elevation_39,RadarSensor:1.OBJ_S_Elevation_40,RadarSensor:1.OBJ_S_Elevation_41,RadarSensor:1.OBJ_S_Elevation_42,RadarSensor:1.OBJ_S_Elevation_43,RadarSensor:1.OBJ_S_Elevation_44,RadarSensor:1.OBJ_S_Elevation_45,RadarSensor:1.OBJ_S_Elevation_46,RadarSensor:1.OBJ_S_Elevation_47,RadarSensor:1.OBJ_S_Elevation_48,RadarSensor:1.OBJ_S_Elevation_49,RadarSensor:1.OBJ_S_Elevation_50,RadarSensor:1.OBJ_S_Elevation_51,RadarSensor:1.OBJ_S_Elevation_52,RadarSensor:1.OBJ_S_Elevation_53,RadarSensor:1.OBJ_S_Elevation_54,RadarSensor:1.OBJ_S_Elevation_55,RadarSensor:1.OBJ_S_Elevation_56,RadarSensor:1.OBJ_S_Elevation_57,RadarSensor:1.OBJ_S_Elevation_58,RadarSensor:1.OBJ_S_Elevation_59,RadarSensor:1.OBJ_S_Elevation_60,RadarSensor:1.OBJ_S_Elevation_61,RadarSensor:1.OBJ_S_Elevation_62,RadarSensor:1.OBJ_S_Elevation_63,RadarSensor:1.OBJ_S_Elevation_64
  Bus Selector:RadarSensor:1_OBJ_S_Range_BS : BusSelector  OutputSignals=RadarSensor:1.OBJ_S_Range_1,RadarSensor:1.OBJ_S_Range_2,RadarSensor:1.OBJ_S_Range_3,RadarSensor:1.OBJ_S_Range_4,RadarSensor:1.OBJ_S_Range_5,RadarSensor:1.OBJ_S_Range_6,RadarSensor:1.OBJ_S_Range_7,RadarSensor:1.OBJ_S_Range_8,RadarSensor:1.OBJ_S_Range_9,RadarSensor:1.OBJ_S_Range_10,RadarSensor:1.OBJ_S_Range_11,RadarSensor:1.OBJ_S_Range_12,RadarSensor:1.OBJ_S_Range_13,RadarSensor:1.OBJ_S_Range_14,RadarSensor:1.OBJ_S_Range_15,RadarSensor:1.OBJ_S_Range_16,RadarSensor:1.OBJ_S_Range_17,RadarSensor:1.OBJ_S_Range_18,RadarSensor:1.OBJ_S_Range_19,RadarSensor:1.OBJ_S_Range_20,RadarSensor:1.OBJ_S_Range_21,RadarSensor:1.OBJ_S_Range_22,RadarSensor:1.OBJ_S_Range_23,RadarSensor:1.OBJ_S_Range_24,RadarSensor:1.OBJ_S_Range_25,RadarSensor:1.OBJ_S_Range_26,RadarSensor:1.OBJ_S_Range_27,RadarSensor:1.OBJ_S_Range_28,RadarSensor:1.OBJ_S_Range_29,RadarSensor:1.OBJ_S_Range_30,RadarSensor:1.OBJ_S_Range_31,RadarSensor:1.OBJ_S_Range_32,RadarSensor:1.OBJ_S_Range_33,RadarSensor:1.OBJ_S_Range_34,RadarSensor:1.OBJ_S_Range_35,RadarSensor:1.OBJ_S_Range_36,RadarSensor:1.OBJ_S_Range_37,RadarSensor:1.OBJ_S_Range_38,RadarSensor:1.OBJ_S_Range_39,RadarSensor:1.OBJ_S_Range_40,RadarSensor:1.OBJ_S_Range_41,RadarSensor:1.OBJ_S_Range_42,RadarSensor:1.OBJ_S_Range_43,RadarSensor:1.OBJ_S_Range_44,RadarSensor:1.OBJ_S_Range_45,RadarSensor:1.OBJ_S_Range_46,RadarSensor:1.OBJ_S_Range_47,RadarSensor:1.OBJ_S_Range_48,RadarSensor:1.OBJ_S_Range_49,RadarSensor:1.OBJ_S_Range_50,RadarSensor:1.OBJ_S_Range_51,RadarSensor:1.OBJ_S_Range_52,RadarSensor:1.OBJ_S_Range_53,RadarSensor:1.OBJ_S_Range_54,RadarSensor:1.OBJ_S_Range_55,RadarSensor:1.OBJ_S_Range_56,RadarSensor:1.OBJ_S_Range_57,RadarSensor:1.OBJ_S_Range_58,RadarSensor:1.OBJ_S_Range_59,RadarSensor:1.OBJ_S_Range_60,RadarSensor:1.OBJ_S_Range_61,RadarSensor:1.OBJ_S_Range_62,RadarSensor:1.OBJ_S_Range_63,RadarSensor:1.OBJ_S_Range_64
  Bus Selector:RadarSensor:1_OBJ_S_Velocity_BS : BusSelector  OutputSignals=RadarSensor:1.OBJ_S_Velocity_1,RadarSensor:1.OBJ_S_Velocity_2,RadarSensor:1.OBJ_S_Velocity_3,RadarSensor:1.OBJ_S_Velocity_4,RadarSensor:1.OBJ_S_Velocity_5,RadarSensor:1.OBJ_S_Velocity_6,RadarSensor:1.OBJ_S_Velocity_7,RadarSensor:1.OBJ_S_Velocity_8,RadarSensor:1.OBJ_S_Velocity_9,RadarSensor:1.OBJ_S_Velocity_10,RadarSensor:1.OBJ_S_Velocity_11,RadarSensor:1.OBJ_S_Velocity_12,RadarSensor:1.OBJ_S_Velocity_13,RadarSensor:1.OBJ_S_Velocity_14,RadarSensor:1.OBJ_S_Velocity_15,RadarSensor:1.OBJ_S_Velocity_16,RadarSensor:1.OBJ_S_Velocity_17,RadarSensor:1.OBJ_S_Velocity_18,RadarSensor:1.OBJ_S_Velocity_19,RadarSensor:1.OBJ_S_Velocity_20,RadarSensor:1.OBJ_S_Velocity_21,RadarSensor:1.OBJ_S_Velocity_22,RadarSensor:1.OBJ_S_Velocity_23,RadarSensor:1.OBJ_S_Velocity_24,RadarSensor:1.OBJ_S_Velocity_25,RadarSensor:1.OBJ_S_Velocity_26,RadarSensor:1.OBJ_S_Velocity_27,RadarSensor:1.OBJ_S_Velocity_28,RadarSensor:1.OBJ_S_Velocity_29,RadarSensor:1.OBJ_S_Velocity_30,RadarSensor:1.OBJ_S_Velocity_31,RadarSensor:1.OBJ_S_Velocity_32,RadarSensor:1.OBJ_S_Velocity_33,RadarSensor:1.OBJ_S_Velocity_34,RadarSensor:1.OBJ_S_Velocity_35,RadarSensor:1.OBJ_S_Velocity_36,RadarSensor:1.OBJ_S_Velocity_37,RadarSensor:1.OBJ_S_Velocity_38,RadarSensor:1.OBJ_S_Velocity_39,RadarSensor:1.OBJ_S_Velocity_40,RadarSensor:1.OBJ_S_Velocity_41,RadarSensor:1.OBJ_S_Velocity_42,RadarSensor:1.OBJ_S_Velocity_43,RadarSensor:1.OBJ_S_Velocity_44,RadarSensor:1.OBJ_S_Velocity_45,RadarSensor:1.OBJ_S_Velocity_46,RadarSensor:1.OBJ_S_Velocity_47,RadarSensor:1.OBJ_S_Velocity_48,RadarSensor:1.OBJ_S_Velocity_49,RadarSensor:1.OBJ_S_Velocity_50,RadarSensor:1.OBJ_S_Velocity_51,RadarSensor:1.OBJ_S_Velocity_52,RadarSensor:1.OBJ_S_Velocity_53,RadarSensor:1.OBJ_S_Velocity_54,RadarSensor:1.OBJ_S_Velocity_55,RadarSensor:1.OBJ_S_Velocity_56,RadarSensor:1.OBJ_S_Velocity_57,RadarSensor:1.OBJ_S_Velocity_58,RadarSensor:1.OBJ_S_Velocity_59,RadarSensor:1.OBJ_S_Velocity_60,RadarSensor:1.OBJ_S_Velocity_61,RadarSensor:1.OBJ_S_Velocity_62,RadarSensor:1.OBJ_S_Velocity_63,RadarSensor:1.OBJ_S_Velocity_64
  Bus Selector:RadarSensor:2 : BusSelector  OutputSignals=RadarSensor:2.time,RadarSensor:2.width,RadarSensor:2.OBJ_ID,RadarSensor:2.OBJ_Class,RadarSensor:2.OBJ_S_Azimuth,RadarSensor:2.OBJ_S_Elevation,RadarSensor:2.OBJ_S_Velocity,RadarSensor:2.OBJ_S_Range,RadarSensor:2.OBJ_RCS
  Bus Selector:RadarSensor:2_OBJ_Class_BS : BusSelector  OutputSignals=RadarSensor:2.OBJ_Class_1,RadarSensor:2.OBJ_Class_2,RadarSensor:2.OBJ_Class_3,RadarSensor:2.OBJ_Class_4,RadarSensor:2.OBJ_Class_5,RadarSensor:2.OBJ_Class_6,RadarSensor:2.OBJ_Class_7,RadarSensor:2.OBJ_Class_8,RadarSensor:2.OBJ_Class_9,RadarSensor:2.OBJ_Class_10,RadarSensor:2.OBJ_Class_11,RadarSensor:2.OBJ_Class_12,RadarSensor:2.OBJ_Class_13,RadarSensor:2.OBJ_Class_14,RadarSensor:2.OBJ_Class_15,RadarSensor:2.OBJ_Class_16,RadarSensor:2.OBJ_Class_17,RadarSensor:2.OBJ_Class_18,RadarSensor:2.OBJ_Class_19,RadarSensor:2.OBJ_Class_20,RadarSensor:2.OBJ_Class_21,RadarSensor:2.OBJ_Class_22,RadarSensor:2.OBJ_Class_23,RadarSensor:2.OBJ_Class_24,RadarSensor:2.OBJ_Class_25,RadarSensor:2.OBJ_Class_26,RadarSensor:2.OBJ_Class_27,RadarSensor:2.OBJ_Class_28,RadarSensor:2.OBJ_Class_29,RadarSensor:2.OBJ_Class_30,RadarSensor:2.OBJ_Class_31,RadarSensor:2.OBJ_Class_32,RadarSensor:2.OBJ_Class_33,RadarSensor:2.OBJ_Class_34,RadarSensor:2.OBJ_Class_35,RadarSensor:2.OBJ_Class_36,RadarSensor:2.OBJ_Class_37,RadarSensor:2.OBJ_Class_38,RadarSensor:2.OBJ_Class_39,RadarSensor:2.OBJ_Class_40,RadarSensor:2.OBJ_Class_41,RadarSensor:2.OBJ_Class_42,RadarSensor:2.OBJ_Class_43,RadarSensor:2.OBJ_Class_44,RadarSensor:2.OBJ_Class_45,RadarSensor:2.OBJ_Class_46,RadarSensor:2.OBJ_Class_47,RadarSensor:2.OBJ_Class_48,RadarSensor:2.OBJ_Class_49,RadarSensor:2.OBJ_Class_50,RadarSensor:2.OBJ_Class_51,RadarSensor:2.OBJ_Class_52,RadarSensor:2.OBJ_Class_53,RadarSensor:2.OBJ_Class_54,RadarSensor:2.OBJ_Class_55,RadarSensor:2.OBJ_Class_56,RadarSensor:2.OBJ_Class_57,RadarSensor:2.OBJ_Class_58,RadarSensor:2.OBJ_Class_59,RadarSensor:2.OBJ_Class_60,RadarSensor:2.OBJ_Class_61,RadarSensor:2.OBJ_Class_62,RadarSensor:2.OBJ_Class_63,RadarSensor:2.OBJ_Class_64
  Bus Selector:RadarSensor:2_OBJ_ID_BS : BusSelector  OutputSignals=RadarSensor:2.OBJ_ID_1,RadarSensor:2.OBJ_ID_2,RadarSensor:2.OBJ_ID_3,RadarSensor:2.OBJ_ID_4,RadarSensor:2.OBJ_ID_5,RadarSensor:2.OBJ_ID_6,RadarSensor:2.OBJ_ID_7,RadarSensor:2.OBJ_ID_8,RadarSensor:2.OBJ_ID_9,RadarSensor:2.OBJ_ID_10,RadarSensor:2.OBJ_ID_11,RadarSensor:2.OBJ_ID_12,RadarSensor:2.OBJ_ID_13,RadarSensor:2.OBJ_ID_14,RadarSensor:2.OBJ_ID_15,RadarSensor:2.OBJ_ID_16,RadarSensor:2.OBJ_ID_17,RadarSensor:2.OBJ_ID_18,RadarSensor:2.OBJ_ID_19,RadarSensor:2.OBJ_ID_20,RadarSensor:2.OBJ_ID_21,RadarSensor:2.OBJ_ID_22,RadarSensor:2.OBJ_ID_23,RadarSensor:2.OBJ_ID_24,RadarSensor:2.OBJ_ID_25,RadarSensor:2.OBJ_ID_26,RadarSensor:2.OBJ_ID_27,RadarSensor:2.OBJ_ID_28,RadarSensor:2.OBJ_ID_29,RadarSensor:2.OBJ_ID_30,RadarSensor:2.OBJ_ID_31,RadarSensor:2.OBJ_ID_32,RadarSensor:2.OBJ_ID_33,RadarSensor:2.OBJ_ID_34,RadarSensor:2.OBJ_ID_35,RadarSensor:2.OBJ_ID_36,RadarSensor:2.OBJ_ID_37,RadarSensor:2.OBJ_ID_38,RadarSensor:2.OBJ_ID_39,RadarSensor:2.OBJ_ID_40,RadarSensor:2.OBJ_ID_41,RadarSensor:2.OBJ_ID_42,RadarSensor:2.OBJ_ID_43,RadarSensor:2.OBJ_ID_44,RadarSensor:2.OBJ_ID_45,RadarSensor:2.OBJ_ID_46,RadarSensor:2.OBJ_ID_47,RadarSensor:2.OBJ_ID_48,RadarSensor:2.OBJ_ID_49,RadarSensor:2.OBJ_ID_50,RadarSensor:2.OBJ_ID_51,RadarSensor:2.OBJ_ID_52,RadarSensor:2.OBJ_ID_53,RadarSensor:2.OBJ_ID_54,RadarSensor:2.OBJ_ID_55,RadarSensor:2.OBJ_ID_56,RadarSensor:2.OBJ_ID_57,RadarSensor:2.OBJ_ID_58,RadarSensor:2.OBJ_ID_59,RadarSensor:2.OBJ_ID_60,RadarSensor:2.OBJ_ID_61,RadarSensor:2.OBJ_ID_62,RadarSensor:2.OBJ_ID_63,RadarSensor:2.OBJ_ID_64
  Bus Selector:RadarSensor:2_OBJ_RCS_BS : BusSelector  OutputSignals=RadarSensor:2.OBJ_RCS_1,RadarSensor:2.OBJ_RCS_2,RadarSensor:2.OBJ_RCS_3,RadarSensor:2.OBJ_RCS_4,RadarSensor:2.OBJ_RCS_5,RadarSensor:2.OBJ_RCS_6,RadarSensor:2.OBJ_RCS_7,RadarSensor:2.OBJ_RCS_8,RadarSensor:2.OBJ_RCS_9,RadarSensor:2.OBJ_RCS_10,RadarSensor:2.OBJ_RCS_11,RadarSensor:2.OBJ_RCS_12,RadarSensor:2.OBJ_RCS_13,RadarSensor:2.OBJ_RCS_14,RadarSensor:2.OBJ_RCS_15,RadarSensor:2.OBJ_RCS_16,RadarSensor:2.OBJ_RCS_17,RadarSensor:2.OBJ_RCS_18,RadarSensor:2.OBJ_RCS_19,RadarSensor:2.OBJ_RCS_20,RadarSensor:2.OBJ_RCS_21,RadarSensor:2.OBJ_RCS_22,RadarSensor:2.OBJ_RCS_23,RadarSensor:2.OBJ_RCS_24,RadarSensor:2.OBJ_RCS_25,RadarSensor:2.OBJ_RCS_26,RadarSensor:2.OBJ_RCS_27,RadarSensor:2.OBJ_RCS_28,RadarSensor:2.OBJ_RCS_29,RadarSensor:2.OBJ_RCS_30,RadarSensor:2.OBJ_RCS_31,RadarSensor:2.OBJ_RCS_32,RadarSensor:2.OBJ_RCS_33,RadarSensor:2.OBJ_RCS_34,RadarSensor:2.OBJ_RCS_35,RadarSensor:2.OBJ_RCS_36,RadarSensor:2.OBJ_RCS_37,RadarSensor:2.OBJ_RCS_38,RadarSensor:2.OBJ_RCS_39,RadarSensor:2.OBJ_RCS_40,RadarSensor:2.OBJ_RCS_41,RadarSensor:2.OBJ_RCS_42,RadarSensor:2.OBJ_RCS_43,RadarSensor:2.OBJ_RCS_44,RadarSensor:2.OBJ_RCS_45,RadarSensor:2.OBJ_RCS_46,RadarSensor:2.OBJ_RCS_47,RadarSensor:2.OBJ_RCS_48,RadarSensor:2.OBJ_RCS_49,RadarSensor:2.OBJ_RCS_50,RadarSensor:2.OBJ_RCS_51,RadarSensor:2.OBJ_RCS_52,RadarSensor:2.OBJ_RCS_53,RadarSensor:2.OBJ_RCS_54,RadarSensor:2.OBJ_RCS_55,RadarSensor:2.OBJ_RCS_56,RadarSensor:2.OBJ_RCS_57,RadarSensor:2.OBJ_RCS_58,RadarSensor:2.OBJ_RCS_59,RadarSensor:2.OBJ_RCS_60,RadarSensor:2.OBJ_RCS_61,RadarSensor:2.OBJ_RCS_62,RadarSensor:2.OBJ_RCS_63,RadarSensor:2.OBJ_RCS_64
  Bus Selector:RadarSensor:2_OBJ_S_Azimuth_BS : BusSelector  OutputSignals=RadarSensor:2.OBJ_S_Azimuth_1,RadarSensor:2.OBJ_S_Azimuth_2,RadarSensor:2.OBJ_S_Azimuth_3,RadarSensor:2.OBJ_S_Azimuth_4,RadarSensor:2.OBJ_S_Azimuth_5,RadarSensor:2.OBJ_S_Azimuth_6,RadarSensor:2.OBJ_S_Azimuth_7,RadarSensor:2.OBJ_S_Azimuth_8,RadarSensor:2.OBJ_S_Azimuth_9,RadarSensor:2.OBJ_S_Azimuth_10,RadarSensor:2.OBJ_S_Azimuth_11,RadarSensor:2.OBJ_S_Azimuth_12,RadarSensor:2.OBJ_S_Azimuth_13,RadarSensor:2.OBJ_S_Azimuth_14,RadarSensor:2.OBJ_S_Azimuth_15,RadarSensor:2.OBJ_S_Azimuth_16,RadarSensor:2.OBJ_S_Azimuth_17,RadarSensor:2.OBJ_S_Azimuth_18,RadarSensor:2.OBJ_S_Azimuth_19,RadarSensor:2.OBJ_S_Azimuth_20,RadarSensor:2.OBJ_S_Azimuth_21,RadarSensor:2.OBJ_S_Azimuth_22,RadarSensor:2.OBJ_S_Azimuth_23,RadarSensor:2.OBJ_S_Azimuth_24,RadarSensor:2.OBJ_S_Azimuth_25,RadarSensor:2.OBJ_S_Azimuth_26,RadarSensor:2.OBJ_S_Azimuth_27,RadarSensor:2.OBJ_S_Azimuth_28,RadarSensor:2.OBJ_S_Azimuth_29,RadarSensor:2.OBJ_S_Azimuth_30,RadarSensor:2.OBJ_S_Azimuth_31,RadarSensor:2.OBJ_S_Azimuth_32,RadarSensor:2.OBJ_S_Azimuth_33,RadarSensor:2.OBJ_S_Azimuth_34,RadarSensor:2.OBJ_S_Azimuth_35,RadarSensor:2.OBJ_S_Azimuth_36,RadarSensor:2.OBJ_S_Azimuth_37,RadarSensor:2.OBJ_S_Azimuth_38,RadarSensor:2.OBJ_S_Azimuth_39,RadarSensor:2.OBJ_S_Azimuth_40,RadarSensor:2.OBJ_S_Azimuth_41,RadarSensor:2.OBJ_S_Azimuth_42,RadarSensor:2.OBJ_S_Azimuth_43,RadarSensor:2.OBJ_S_Azimuth_44,RadarSensor:2.OBJ_S_Azimuth_45,RadarSensor:2.OBJ_S_Azimuth_46,RadarSensor:2.OBJ_S_Azimuth_47,RadarSensor:2.OBJ_S_Azimuth_48,RadarSensor:2.OBJ_S_Azimuth_49,RadarSensor:2.OBJ_S_Azimuth_50,RadarSensor:2.OBJ_S_Azimuth_51,RadarSensor:2.OBJ_S_Azimuth_52,RadarSensor:2.OBJ_S_Azimuth_53,RadarSensor:2.OBJ_S_Azimuth_54,RadarSensor:2.OBJ_S_Azimuth_55,RadarSensor:2.OBJ_S_Azimuth_56,RadarSensor:2.OBJ_S_Azimuth_57,RadarSensor:2.OBJ_S_Azimuth_58,RadarSensor:2.OBJ_S_Azimuth_59,RadarSensor:2.OBJ_S_Azimuth_60,RadarSensor:2.OBJ_S_Azimuth_61,RadarSensor:2.OBJ_S_Azimuth_62,RadarSensor:2.OBJ_S_Azimuth_63,RadarSensor:2.OBJ_S_Azimuth_64
  Bus Selector:RadarSensor:2_OBJ_S_Elevation_BS : BusSelector  OutputSignals=RadarSensor:2.OBJ_S_Elevation_1,RadarSensor:2.OBJ_S_Elevation_2,RadarSensor:2.OBJ_S_Elevation_3,RadarSensor:2.OBJ_S_Elevation_4,RadarSensor:2.OBJ_S_Elevation_5,RadarSensor:2.OBJ_S_Elevation_6,RadarSensor:2.OBJ_S_Elevation_7,RadarSensor:2.OBJ_S_Elevation_8,RadarSensor:2.OBJ_S_Elevation_9,RadarSensor:2.OBJ_S_Elevation_10,RadarSensor:2.OBJ_S_Elevation_11,RadarSensor:2.OBJ_S_Elevation_12,RadarSensor:2.OBJ_S_Elevation_13,RadarSensor:2.OBJ_S_Elevation_14,RadarSensor:2.OBJ_S_Elevation_15,RadarSensor:2.OBJ_S_Elevation_16,RadarSensor:2.OBJ_S_Elevation_17,RadarSensor:2.OBJ_S_Elevation_18,RadarSensor:2.OBJ_S_Elevation_19,RadarSensor:2.OBJ_S_Elevation_20,RadarSensor:2.OBJ_S_Elevation_21,RadarSensor:2.OBJ_S_Elevation_22,RadarSensor:2.OBJ_S_Elevation_23,RadarSensor:2.OBJ_S_Elevation_24,RadarSensor:2.OBJ_S_Elevation_25,RadarSensor:2.OBJ_S_Elevation_26,RadarSensor:2.OBJ_S_Elevation_27,RadarSensor:2.OBJ_S_Elevation_28,RadarSensor:2.OBJ_S_Elevation_29,RadarSensor:2.OBJ_S_Elevation_30,RadarSensor:2.OBJ_S_Elevation_31,RadarSensor:2.OBJ_S_Elevation_32,RadarSensor:2.OBJ_S_Elevation_33,RadarSensor:2.OBJ_S_Elevation_34,RadarSensor:2.OBJ_S_Elevation_35,RadarSensor:2.OBJ_S_Elevation_36,RadarSensor:2.OBJ_S_Elevation_37,RadarSensor:2.OBJ_S_Elevation_38,RadarSensor:2.OBJ_S_Elevation_39,RadarSensor:2.OBJ_S_Elevation_40,RadarSensor:2.OBJ_S_Elevation_41,RadarSensor:2.OBJ_S_Elevation_42,RadarSensor:2.OBJ_S_Elevation_43,RadarSensor:2.OBJ_S_Elevation_44,RadarSensor:2.OBJ_S_Elevation_45,RadarSensor:2.OBJ_S_Elevation_46,RadarSensor:2.OBJ_S_Elevation_47,RadarSensor:2.OBJ_S_Elevation_48,RadarSensor:2.OBJ_S_Elevation_49,RadarSensor:2.OBJ_S_Elevation_50,RadarSensor:2.OBJ_S_Elevation_51,RadarSensor:2.OBJ_S_Elevation_52,RadarSensor:2.OBJ_S_Elevation_53,RadarSensor:2.OBJ_S_Elevation_54,RadarSensor:2.OBJ_S_Elevation_55,RadarSensor:2.OBJ_S_Elevation_56,RadarSensor:2.OBJ_S_Elevation_57,RadarSensor:2.OBJ_S_Elevation_58,RadarSensor:2.OBJ_S_Elevation_59,RadarSensor:2.OBJ_S_Elevation_60,RadarSensor:2.OBJ_S_Elevation_61,RadarSensor:2.OBJ_S_Elevation_62,RadarSensor:2.OBJ_S_Elevation_63,RadarSensor:2.OBJ_S_Elevation_64
  Bus Selector:RadarSensor:2_OBJ_S_Range_BS : BusSelector  OutputSignals=RadarSensor:2.OBJ_S_Range_1,RadarSensor:2.OBJ_S_Range_2,RadarSensor:2.OBJ_S_Range_3,RadarSensor:2.OBJ_S_Range_4,RadarSensor:2.OBJ_S_Range_5,RadarSensor:2.OBJ_S_Range_6,RadarSensor:2.OBJ_S_Range_7,RadarSensor:2.OBJ_S_Range_8,RadarSensor:2.OBJ_S_Range_9,RadarSensor:2.OBJ_S_Range_10,RadarSensor:2.OBJ_S_Range_11,RadarSensor:2.OBJ_S_Range_12,RadarSensor:2.OBJ_S_Range_13,RadarSensor:2.OBJ_S_Range_14,RadarSensor:2.OBJ_S_Range_15,RadarSensor:2.OBJ_S_Range_16,RadarSensor:2.OBJ_S_Range_17,RadarSensor:2.OBJ_S_Range_18,RadarSensor:2.OBJ_S_Range_19,RadarSensor:2.OBJ_S_Range_20,RadarSensor:2.OBJ_S_Range_21,RadarSensor:2.OBJ_S_Range_22,RadarSensor:2.OBJ_S_Range_23,RadarSensor:2.OBJ_S_Range_24,RadarSensor:2.OBJ_S_Range_25,RadarSensor:2.OBJ_S_Range_26,RadarSensor:2.OBJ_S_Range_27,RadarSensor:2.OBJ_S_Range_28,RadarSensor:2.OBJ_S_Range_29,RadarSensor:2.OBJ_S_Range_30,RadarSensor:2.OBJ_S_Range_31,RadarSensor:2.OBJ_S_Range_32,RadarSensor:2.OBJ_S_Range_33,RadarSensor:2.OBJ_S_Range_34,RadarSensor:2.OBJ_S_Range_35,RadarSensor:2.OBJ_S_Range_36,RadarSensor:2.OBJ_S_Range_37,RadarSensor:2.OBJ_S_Range_38,RadarSensor:2.OBJ_S_Range_39,RadarSensor:2.OBJ_S_Range_40,RadarSensor:2.OBJ_S_Range_41,RadarSensor:2.OBJ_S_Range_42,RadarSensor:2.OBJ_S_Range_43,RadarSensor:2.OBJ_S_Range_44,RadarSensor:2.OBJ_S_Range_45,RadarSensor:2.OBJ_S_Range_46,RadarSensor:2.OBJ_S_Range_47,RadarSensor:2.OBJ_S_Range_48,RadarSensor:2.OBJ_S_Range_49,RadarSensor:2.OBJ_S_Range_50,RadarSensor:2.OBJ_S_Range_51,RadarSensor:2.OBJ_S_Range_52,RadarSensor:2.OBJ_S_Range_53,RadarSensor:2.OBJ_S_Range_54,RadarSensor:2.OBJ_S_Range_55,RadarSensor:2.OBJ_S_Range_56,RadarSensor:2.OBJ_S_Range_57,RadarSensor:2.OBJ_S_Range_58,RadarSensor:2.OBJ_S_Range_59,RadarSensor:2.OBJ_S_Range_60,RadarSensor:2.OBJ_S_Range_61,RadarSensor:2.OBJ_S_Range_62,RadarSensor:2.OBJ_S_Range_63,RadarSensor:2.OBJ_S_Range_64
  Bus Selector:RadarSensor:2_OBJ_S_Velocity_BS : BusSelector  OutputSignals=RadarSensor:2.OBJ_S_Velocity_1,RadarSensor:2.OBJ_S_Velocity_2,RadarSensor:2.OBJ_S_Velocity_3,RadarSensor:2.OBJ_S_Velocity_4,RadarSensor:2.OBJ_S_Velocity_5,RadarSensor:2.OBJ_S_Velocity_6,RadarSensor:2.OBJ_S_Velocity_7,RadarSensor:2.OBJ_S_Velocity_8,RadarSensor:2.OBJ_S_Velocity_9,RadarSensor:2.OBJ_S_Velocity_10,RadarSensor:2.OBJ_S_Velocity_11,RadarSensor:2.OBJ_S_Velocity_12,RadarSensor:2.OBJ_S_Velocity_13,RadarSensor:2.OBJ_S_Velocity_14,RadarSensor:2.OBJ_S_Velocity_15,RadarSensor:2.OBJ_S_Velocity_16,RadarSensor:2.OBJ_S_Velocity_17,RadarSensor:2.OBJ_S_Velocity_18,RadarSensor:2.OBJ_S_Velocity_19,RadarSensor:2.OBJ_S_Velocity_20,RadarSensor:2.OBJ_S_Velocity_21,RadarSensor:2.OBJ_S_Velocity_22,RadarSensor:2.OBJ_S_Velocity_23,RadarSensor:2.OBJ_S_Velocity_24,RadarSensor:2.OBJ_S_Velocity_25,RadarSensor:2.OBJ_S_Velocity_26,RadarSensor:2.OBJ_S_Velocity_27,RadarSensor:2.OBJ_S_Velocity_28,RadarSensor:2.OBJ_S_Velocity_29,RadarSensor:2.OBJ_S_Velocity_30,RadarSensor:2.OBJ_S_Velocity_31,RadarSensor:2.OBJ_S_Velocity_32,RadarSensor:2.OBJ_S_Velocity_33,RadarSensor:2.OBJ_S_Velocity_34,RadarSensor:2.OBJ_S_Velocity_35,RadarSensor:2.OBJ_S_Velocity_36,RadarSensor:2.OBJ_S_Velocity_37,RadarSensor:2.OBJ_S_Velocity_38,RadarSensor:2.OBJ_S_Velocity_39,RadarSensor:2.OBJ_S_Velocity_40,RadarSensor:2.OBJ_S_Velocity_41,RadarSensor:2.OBJ_S_Velocity_42,RadarSensor:2.OBJ_S_Velocity_43,RadarSensor:2.OBJ_S_Velocity_44,RadarSensor:2.OBJ_S_Velocity_45,RadarSensor:2.OBJ_S_Velocity_46,RadarSensor:2.OBJ_S_Velocity_47,RadarSensor:2.OBJ_S_Velocity_48,RadarSensor:2.OBJ_S_Velocity_49,RadarSensor:2.OBJ_S_Velocity_50,RadarSensor:2.OBJ_S_Velocity_51,RadarSensor:2.OBJ_S_Velocity_52,RadarSensor:2.OBJ_S_Velocity_53,RadarSensor:2.OBJ_S_Velocity_54,RadarSensor:2.OBJ_S_Velocity_55,RadarSensor:2.OBJ_S_Velocity_56,RadarSensor:2.OBJ_S_Velocity_57,RadarSensor:2.OBJ_S_Velocity_58,RadarSensor:2.OBJ_S_Velocity_59,RadarSensor:2.OBJ_S_Velocity_60,RadarSensor:2.OBJ_S_Velocity_61,RadarSensor:2.OBJ_S_Velocity_62,RadarSensor:2.OBJ_S_Velocity_63,RadarSensor:2.OBJ_S_Velocity_64
  Bus Selector:RadarSensor:3 : BusSelector  OutputSignals=RadarSensor:3.time,RadarSensor:3.width,RadarSensor:3.OBJ_ID,RadarSensor:3.OBJ_Class,RadarSensor:3.OBJ_S_Azimuth,RadarSensor:3.OBJ_S_Elevation,RadarSensor:3.OBJ_S_Velocity,RadarSensor:3.OBJ_S_Range,RadarSensor:3.OBJ_RCS
  Bus Selector:RadarSensor:3_OBJ_Class_BS : BusSelector  OutputSignals=RadarSensor:3.OBJ_Class_1,RadarSensor:3.OBJ_Class_2,RadarSensor:3.OBJ_Class_3,RadarSensor:3.OBJ_Class_4,RadarSensor:3.OBJ_Class_5,RadarSensor:3.OBJ_Class_6,RadarSensor:3.OBJ_Class_7,RadarSensor:3.OBJ_Class_8,RadarSensor:3.OBJ_Class_9,RadarSensor:3.OBJ_Class_10,RadarSensor:3.OBJ_Class_11,RadarSensor:3.OBJ_Class_12,RadarSensor:3.OBJ_Class_13,RadarSensor:3.OBJ_Class_14,RadarSensor:3.OBJ_Class_15,RadarSensor:3.OBJ_Class_16,RadarSensor:3.OBJ_Class_17,RadarSensor:3.OBJ_Class_18,RadarSensor:3.OBJ_Class_19,RadarSensor:3.OBJ_Class_20,RadarSensor:3.OBJ_Class_21,RadarSensor:3.OBJ_Class_22,RadarSensor:3.OBJ_Class_23,RadarSensor:3.OBJ_Class_24,RadarSensor:3.OBJ_Class_25,RadarSensor:3.OBJ_Class_26,RadarSensor:3.OBJ_Class_27,RadarSensor:3.OBJ_Class_28,RadarSensor:3.OBJ_Class_29,RadarSensor:3.OBJ_Class_30,RadarSensor:3.OBJ_Class_31,RadarSensor:3.OBJ_Class_32,RadarSensor:3.OBJ_Class_33,RadarSensor:3.OBJ_Class_34,RadarSensor:3.OBJ_Class_35,RadarSensor:3.OBJ_Class_36,RadarSensor:3.OBJ_Class_37,RadarSensor:3.OBJ_Class_38,RadarSensor:3.OBJ_Class_39,RadarSensor:3.OBJ_Class_40,RadarSensor:3.OBJ_Class_41,RadarSensor:3.OBJ_Class_42,RadarSensor:3.OBJ_Class_43,RadarSensor:3.OBJ_Class_44,RadarSensor:3.OBJ_Class_45,RadarSensor:3.OBJ_Class_46,RadarSensor:3.OBJ_Class_47,RadarSensor:3.OBJ_Class_48,RadarSensor:3.OBJ_Class_49,RadarSensor:3.OBJ_Class_50,RadarSensor:3.OBJ_Class_51,RadarSensor:3.OBJ_Class_52,RadarSensor:3.OBJ_Class_53,RadarSensor:3.OBJ_Class_54,RadarSensor:3.OBJ_Class_55,RadarSensor:3.OBJ_Class_56,RadarSensor:3.OBJ_Class_57,RadarSensor:3.OBJ_Class_58,RadarSensor:3.OBJ_Class_59,RadarSensor:3.OBJ_Class_60,RadarSensor:3.OBJ_Class_61,RadarSensor:3.OBJ_Class_62,RadarSensor:3.OBJ_Class_63,RadarSensor:3.OBJ_Class_64
  Bus Selector:RadarSensor:3_OBJ_ID_BS : BusSelector  OutputSignals=RadarSensor:3.OBJ_ID_1,RadarSensor:3.OBJ_ID_2,RadarSensor:3.OBJ_ID_3,RadarSensor:3.OBJ_ID_4,RadarSensor:3.OBJ_ID_5,RadarSensor:3.OBJ_ID_6,RadarSensor:3.OBJ_ID_7,RadarSensor:3.OBJ_ID_8,RadarSensor:3.OBJ_ID_9,RadarSensor:3.OBJ_ID_10,RadarSensor:3.OBJ_ID_11,RadarSensor:3.OBJ_ID_12,RadarSensor:3.OBJ_ID_13,RadarSensor:3.OBJ_ID_14,RadarSensor:3.OBJ_ID_15,RadarSensor:3.OBJ_ID_16,RadarSensor:3.OBJ_ID_17,RadarSensor:3.OBJ_ID_18,RadarSensor:3.OBJ_ID_19,RadarSensor:3.OBJ_ID_20,RadarSensor:3.OBJ_ID_21,RadarSensor:3.OBJ_ID_22,RadarSensor:3.OBJ_ID_23,RadarSensor:3.OBJ_ID_24,RadarSensor:3.OBJ_ID_25,RadarSensor:3.OBJ_ID_26,RadarSensor:3.OBJ_ID_27,RadarSensor:3.OBJ_ID_28,RadarSensor:3.OBJ_ID_29,RadarSensor:3.OBJ_ID_30,RadarSensor:3.OBJ_ID_31,RadarSensor:3.OBJ_ID_32,RadarSensor:3.OBJ_ID_33,RadarSensor:3.OBJ_ID_34,RadarSensor:3.OBJ_ID_35,RadarSensor:3.OBJ_ID_36,RadarSensor:3.OBJ_ID_37,RadarSensor:3.OBJ_ID_38,RadarSensor:3.OBJ_ID_39,RadarSensor:3.OBJ_ID_40,RadarSensor:3.OBJ_ID_41,RadarSensor:3.OBJ_ID_42,RadarSensor:3.OBJ_ID_43,RadarSensor:3.OBJ_ID_44,RadarSensor:3.OBJ_ID_45,RadarSensor:3.OBJ_ID_46,RadarSensor:3.OBJ_ID_47,RadarSensor:3.OBJ_ID_48,RadarSensor:3.OBJ_ID_49,RadarSensor:3.OBJ_ID_50,RadarSensor:3.OBJ_ID_51,RadarSensor:3.OBJ_ID_52,RadarSensor:3.OBJ_ID_53,RadarSensor:3.OBJ_ID_54,RadarSensor:3.OBJ_ID_55,RadarSensor:3.OBJ_ID_56,RadarSensor:3.OBJ_ID_57,RadarSensor:3.OBJ_ID_58,RadarSensor:3.OBJ_ID_59,RadarSensor:3.OBJ_ID_60,RadarSensor:3.OBJ_ID_61,RadarSensor:3.OBJ_ID_62,RadarSensor:3.OBJ_ID_63,RadarSensor:3.OBJ_ID_64
  Bus Selector:RadarSensor:3_OBJ_RCS_BS : BusSelector  OutputSignals=RadarSensor:3.OBJ_RCS_1,RadarSensor:3.OBJ_RCS_2,RadarSensor:3.OBJ_RCS_3,RadarSensor:3.OBJ_RCS_4,RadarSensor:3.OBJ_RCS_5,RadarSensor:3.OBJ_RCS_6,RadarSensor:3.OBJ_RCS_7,RadarSensor:3.OBJ_RCS_8,RadarSensor:3.OBJ_RCS_9,RadarSensor:3.OBJ_RCS_10,RadarSensor:3.OBJ_RCS_11,RadarSensor:3.OBJ_RCS_12,RadarSensor:3.OBJ_RCS_13,RadarSensor:3.OBJ_RCS_14,RadarSensor:3.OBJ_RCS_15,RadarSensor:3.OBJ_RCS_16,RadarSensor:3.OBJ_RCS_17,RadarSensor:3.OBJ_RCS_18,RadarSensor:3.OBJ_RCS_19,RadarSensor:3.OBJ_RCS_20,RadarSensor:3.OBJ_RCS_21,RadarSensor:3.OBJ_RCS_22,RadarSensor:3.OBJ_RCS_23,RadarSensor:3.OBJ_RCS_24,RadarSensor:3.OBJ_RCS_25,RadarSensor:3.OBJ_RCS_26,RadarSensor:3.OBJ_RCS_27,RadarSensor:3.OBJ_RCS_28,RadarSensor:3.OBJ_RCS_29,RadarSensor:3.OBJ_RCS_30,RadarSensor:3.OBJ_RCS_31,RadarSensor:3.OBJ_RCS_32,RadarSensor:3.OBJ_RCS_33,RadarSensor:3.OBJ_RCS_34,RadarSensor:3.OBJ_RCS_35,RadarSensor:3.OBJ_RCS_36,RadarSensor:3.OBJ_RCS_37,RadarSensor:3.OBJ_RCS_38,RadarSensor:3.OBJ_RCS_39,RadarSensor:3.OBJ_RCS_40,RadarSensor:3.OBJ_RCS_41,RadarSensor:3.OBJ_RCS_42,RadarSensor:3.OBJ_RCS_43,RadarSensor:3.OBJ_RCS_44,RadarSensor:3.OBJ_RCS_45,RadarSensor:3.OBJ_RCS_46,RadarSensor:3.OBJ_RCS_47,RadarSensor:3.OBJ_RCS_48,RadarSensor:3.OBJ_RCS_49,RadarSensor:3.OBJ_RCS_50,RadarSensor:3.OBJ_RCS_51,RadarSensor:3.OBJ_RCS_52,RadarSensor:3.OBJ_RCS_53,RadarSensor:3.OBJ_RCS_54,RadarSensor:3.OBJ_RCS_55,RadarSensor:3.OBJ_RCS_56,RadarSensor:3.OBJ_RCS_57,RadarSensor:3.OBJ_RCS_58,RadarSensor:3.OBJ_RCS_59,RadarSensor:3.OBJ_RCS_60,RadarSensor:3.OBJ_RCS_61,RadarSensor:3.OBJ_RCS_62,RadarSensor:3.OBJ_RCS_63,RadarSensor:3.OBJ_RCS_64
  Bus Selector:RadarSensor:3_OBJ_S_Azimuth_BS : BusSelector  OutputSignals=RadarSensor:3.OBJ_S_Azimuth_1,RadarSensor:3.OBJ_S_Azimuth_2,RadarSensor:3.OBJ_S_Azimuth_3,RadarSensor:3.OBJ_S_Azimuth_4,RadarSensor:3.OBJ_S_Azimuth_5,RadarSensor:3.OBJ_S_Azimuth_6,RadarSensor:3.OBJ_S_Azimuth_7,RadarSensor:3.OBJ_S_Azimuth_8,RadarSensor:3.OBJ_S_Azimuth_9,RadarSensor:3.OBJ_S_Azimuth_10,RadarSensor:3.OBJ_S_Azimuth_11,RadarSensor:3.OBJ_S_Azimuth_12,RadarSensor:3.OBJ_S_Azimuth_13,RadarSensor:3.OBJ_S_Azimuth_14,RadarSensor:3.OBJ_S_Azimuth_15,RadarSensor:3.OBJ_S_Azimuth_16,RadarSensor:3.OBJ_S_Azimuth_17,RadarSensor:3.OBJ_S_Azimuth_18,RadarSensor:3.OBJ_S_Azimuth_19,RadarSensor:3.OBJ_S_Azimuth_20,RadarSensor:3.OBJ_S_Azimuth_21,RadarSensor:3.OBJ_S_Azimuth_22,RadarSensor:3.OBJ_S_Azimuth_23,RadarSensor:3.OBJ_S_Azimuth_24,RadarSensor:3.OBJ_S_Azimuth_25,RadarSensor:3.OBJ_S_Azimuth_26,RadarSensor:3.OBJ_S_Azimuth_27,RadarSensor:3.OBJ_S_Azimuth_28,RadarSensor:3.OBJ_S_Azimuth_29,RadarSensor:3.OBJ_S_Azimuth_30,RadarSensor:3.OBJ_S_Azimuth_31,RadarSensor:3.OBJ_S_Azimuth_32,RadarSensor:3.OBJ_S_Azimuth_33,RadarSensor:3.OBJ_S_Azimuth_34,RadarSensor:3.OBJ_S_Azimuth_35,RadarSensor:3.OBJ_S_Azimuth_36,RadarSensor:3.OBJ_S_Azimuth_37,RadarSensor:3.OBJ_S_Azimuth_38,RadarSensor:3.OBJ_S_Azimuth_39,RadarSensor:3.OBJ_S_Azimuth_40,RadarSensor:3.OBJ_S_Azimuth_41,RadarSensor:3.OBJ_S_Azimuth_42,RadarSensor:3.OBJ_S_Azimuth_43,RadarSensor:3.OBJ_S_Azimuth_44,RadarSensor:3.OBJ_S_Azimuth_45,RadarSensor:3.OBJ_S_Azimuth_46,RadarSensor:3.OBJ_S_Azimuth_47,RadarSensor:3.OBJ_S_Azimuth_48,RadarSensor:3.OBJ_S_Azimuth_49,RadarSensor:3.OBJ_S_Azimuth_50,RadarSensor:3.OBJ_S_Azimuth_51,RadarSensor:3.OBJ_S_Azimuth_52,RadarSensor:3.OBJ_S_Azimuth_53,RadarSensor:3.OBJ_S_Azimuth_54,RadarSensor:3.OBJ_S_Azimuth_55,RadarSensor:3.OBJ_S_Azimuth_56,RadarSensor:3.OBJ_S_Azimuth_57,RadarSensor:3.OBJ_S_Azimuth_58,RadarSensor:3.OBJ_S_Azimuth_59,RadarSensor:3.OBJ_S_Azimuth_60,RadarSensor:3.OBJ_S_Azimuth_61,RadarSensor:3.OBJ_S_Azimuth_62,RadarSensor:3.OBJ_S_Azimuth_63,RadarSensor:3.OBJ_S_Azimuth_64
  Bus Selector:RadarSensor:3_OBJ_S_Elevation_BS : BusSelector  OutputSignals=RadarSensor:3.OBJ_S_Elevation_1,RadarSensor:3.OBJ_S_Elevation_2,RadarSensor:3.OBJ_S_Elevation_3,RadarSensor:3.OBJ_S_Elevation_4,RadarSensor:3.OBJ_S_Elevation_5,RadarSensor:3.OBJ_S_Elevation_6,RadarSensor:3.OBJ_S_Elevation_7,RadarSensor:3.OBJ_S_Elevation_8,RadarSensor:3.OBJ_S_Elevation_9,RadarSensor:3.OBJ_S_Elevation_10,RadarSensor:3.OBJ_S_Elevation_11,RadarSensor:3.OBJ_S_Elevation_12,RadarSensor:3.OBJ_S_Elevation_13,RadarSensor:3.OBJ_S_Elevation_14,RadarSensor:3.OBJ_S_Elevation_15,RadarSensor:3.OBJ_S_Elevation_16,RadarSensor:3.OBJ_S_Elevation_17,RadarSensor:3.OBJ_S_Elevation_18,RadarSensor:3.OBJ_S_Elevation_19,RadarSensor:3.OBJ_S_Elevation_20,RadarSensor:3.OBJ_S_Elevation_21,RadarSensor:3.OBJ_S_Elevation_22,RadarSensor:3.OBJ_S_Elevation_23,RadarSensor:3.OBJ_S_Elevation_24,RadarSensor:3.OBJ_S_Elevation_25,RadarSensor:3.OBJ_S_Elevation_26,RadarSensor:3.OBJ_S_Elevation_27,RadarSensor:3.OBJ_S_Elevation_28,RadarSensor:3.OBJ_S_Elevation_29,RadarSensor:3.OBJ_S_Elevation_30,RadarSensor:3.OBJ_S_Elevation_31,RadarSensor:3.OBJ_S_Elevation_32,RadarSensor:3.OBJ_S_Elevation_33,RadarSensor:3.OBJ_S_Elevation_34,RadarSensor:3.OBJ_S_Elevation_35,RadarSensor:3.OBJ_S_Elevation_36,RadarSensor:3.OBJ_S_Elevation_37,RadarSensor:3.OBJ_S_Elevation_38,RadarSensor:3.OBJ_S_Elevation_39,RadarSensor:3.OBJ_S_Elevation_40,RadarSensor:3.OBJ_S_Elevation_41,RadarSensor:3.OBJ_S_Elevation_42,RadarSensor:3.OBJ_S_Elevation_43,RadarSensor:3.OBJ_S_Elevation_44,RadarSensor:3.OBJ_S_Elevation_45,RadarSensor:3.OBJ_S_Elevation_46,RadarSensor:3.OBJ_S_Elevation_47,RadarSensor:3.OBJ_S_Elevation_48,RadarSensor:3.OBJ_S_Elevation_49,RadarSensor:3.OBJ_S_Elevation_50,RadarSensor:3.OBJ_S_Elevation_51,RadarSensor:3.OBJ_S_Elevation_52,RadarSensor:3.OBJ_S_Elevation_53,RadarSensor:3.OBJ_S_Elevation_54,RadarSensor:3.OBJ_S_Elevation_55,RadarSensor:3.OBJ_S_Elevation_56,RadarSensor:3.OBJ_S_Elevation_57,RadarSensor:3.OBJ_S_Elevation_58,RadarSensor:3.OBJ_S_Elevation_59,RadarSensor:3.OBJ_S_Elevation_60,RadarSensor:3.OBJ_S_Elevation_61,RadarSensor:3.OBJ_S_Elevation_62,RadarSensor:3.OBJ_S_Elevation_63,RadarSensor:3.OBJ_S_Elevation_64
  Bus Selector:RadarSensor:3_OBJ_S_Range_BS : BusSelector  OutputSignals=RadarSensor:3.OBJ_S_Range_1,RadarSensor:3.OBJ_S_Range_2,RadarSensor:3.OBJ_S_Range_3,RadarSensor:3.OBJ_S_Range_4,RadarSensor:3.OBJ_S_Range_5,RadarSensor:3.OBJ_S_Range_6,RadarSensor:3.OBJ_S_Range_7,RadarSensor:3.OBJ_S_Range_8,RadarSensor:3.OBJ_S_Range_9,RadarSensor:3.OBJ_S_Range_10,RadarSensor:3.OBJ_S_Range_11,RadarSensor:3.OBJ_S_Range_12,RadarSensor:3.OBJ_S_Range_13,RadarSensor:3.OBJ_S_Range_14,RadarSensor:3.OBJ_S_Range_15,RadarSensor:3.OBJ_S_Range_16,RadarSensor:3.OBJ_S_Range_17,RadarSensor:3.OBJ_S_Range_18,RadarSensor:3.OBJ_S_Range_19,RadarSensor:3.OBJ_S_Range_20,RadarSensor:3.OBJ_S_Range_21,RadarSensor:3.OBJ_S_Range_22,RadarSensor:3.OBJ_S_Range_23,RadarSensor:3.OBJ_S_Range_24,RadarSensor:3.OBJ_S_Range_25,RadarSensor:3.OBJ_S_Range_26,RadarSensor:3.OBJ_S_Range_27,RadarSensor:3.OBJ_S_Range_28,RadarSensor:3.OBJ_S_Range_29,RadarSensor:3.OBJ_S_Range_30,RadarSensor:3.OBJ_S_Range_31,RadarSensor:3.OBJ_S_Range_32,RadarSensor:3.OBJ_S_Range_33,RadarSensor:3.OBJ_S_Range_34,RadarSensor:3.OBJ_S_Range_35,RadarSensor:3.OBJ_S_Range_36,RadarSensor:3.OBJ_S_Range_37,RadarSensor:3.OBJ_S_Range_38,RadarSensor:3.OBJ_S_Range_39,RadarSensor:3.OBJ_S_Range_40,RadarSensor:3.OBJ_S_Range_41,RadarSensor:3.OBJ_S_Range_42,RadarSensor:3.OBJ_S_Range_43,RadarSensor:3.OBJ_S_Range_44,RadarSensor:3.OBJ_S_Range_45,RadarSensor:3.OBJ_S_Range_46,RadarSensor:3.OBJ_S_Range_47,RadarSensor:3.OBJ_S_Range_48,RadarSensor:3.OBJ_S_Range_49,RadarSensor:3.OBJ_S_Range_50,RadarSensor:3.OBJ_S_Range_51,RadarSensor:3.OBJ_S_Range_52,RadarSensor:3.OBJ_S_Range_53,RadarSensor:3.OBJ_S_Range_54,RadarSensor:3.OBJ_S_Range_55,RadarSensor:3.OBJ_S_Range_56,RadarSensor:3.OBJ_S_Range_57,RadarSensor:3.OBJ_S_Range_58,RadarSensor:3.OBJ_S_Range_59,RadarSensor:3.OBJ_S_Range_60,RadarSensor:3.OBJ_S_Range_61,RadarSensor:3.OBJ_S_Range_62,RadarSensor:3.OBJ_S_Range_63,RadarSensor:3.OBJ_S_Range_64
  Bus Selector:RadarSensor:3_OBJ_S_Velocity_BS : BusSelector  OutputSignals=RadarSensor:3.OBJ_S_Velocity_1,RadarSensor:3.OBJ_S_Velocity_2,RadarSensor:3.OBJ_S_Velocity_3,RadarSensor:3.OBJ_S_Velocity_4,RadarSensor:3.OBJ_S_Velocity_5,RadarSensor:3.OBJ_S_Velocity_6,RadarSensor:3.OBJ_S_Velocity_7,RadarSensor:3.OBJ_S_Velocity_8,RadarSensor:3.OBJ_S_Velocity_9,RadarSensor:3.OBJ_S_Velocity_10,RadarSensor:3.OBJ_S_Velocity_11,RadarSensor:3.OBJ_S_Velocity_12,RadarSensor:3.OBJ_S_Velocity_13,RadarSensor:3.OBJ_S_Velocity_14,RadarSensor:3.OBJ_S_Velocity_15,RadarSensor:3.OBJ_S_Velocity_16,RadarSensor:3.OBJ_S_Velocity_17,RadarSensor:3.OBJ_S_Velocity_18,RadarSensor:3.OBJ_S_Velocity_19,RadarSensor:3.OBJ_S_Velocity_20,RadarSensor:3.OBJ_S_Velocity_21,RadarSensor:3.OBJ_S_Velocity_22,RadarSensor:3.OBJ_S_Velocity_23,RadarSensor:3.OBJ_S_Velocity_24,RadarSensor:3.OBJ_S_Velocity_25,RadarSensor:3.OBJ_S_Velocity_26,RadarSensor:3.OBJ_S_Velocity_27,RadarSensor:3.OBJ_S_Velocity_28,RadarSensor:3.OBJ_S_Velocity_29,RadarSensor:3.OBJ_S_Velocity_30,RadarSensor:3.OBJ_S_Velocity_31,RadarSensor:3.OBJ_S_Velocity_32,RadarSensor:3.OBJ_S_Velocity_33,RadarSensor:3.OBJ_S_Velocity_34,RadarSensor:3.OBJ_S_Velocity_35,RadarSensor:3.OBJ_S_Velocity_36,RadarSensor:3.OBJ_S_Velocity_37,RadarSensor:3.OBJ_S_Velocity_38,RadarSensor:3.OBJ_S_Velocity_39,RadarSensor:3.OBJ_S_Velocity_40,RadarSensor:3.OBJ_S_Velocity_41,RadarSensor:3.OBJ_S_Velocity_42,RadarSensor:3.OBJ_S_Velocity_43,RadarSensor:3.OBJ_S_Velocity_44,RadarSensor:3.OBJ_S_Velocity_45,RadarSensor:3.OBJ_S_Velocity_46,RadarSensor:3.OBJ_S_Velocity_47,RadarSensor:3.OBJ_S_Velocity_48,RadarSensor:3.OBJ_S_Velocity_49,RadarSensor:3.OBJ_S_Velocity_50,RadarSensor:3.OBJ_S_Velocity_51,RadarSensor:3.OBJ_S_Velocity_52,RadarSensor:3.OBJ_S_Velocity_53,RadarSensor:3.OBJ_S_Velocity_54,RadarSensor:3.OBJ_S_Velocity_55,RadarSensor:3.OBJ_S_Velocity_56,RadarSensor:3.OBJ_S_Velocity_57,RadarSensor:3.OBJ_S_Velocity_58,RadarSensor:3.OBJ_S_Velocity_59,RadarSensor:3.OBJ_S_Velocity_60,RadarSensor:3.OBJ_S_Velocity_61,RadarSensor:3.OBJ_S_Velocity_62,RadarSensor:3.OBJ_S_Velocity_63,RadarSensor:3.OBJ_S_Velocity_64
  Bus Selector:RadarSensor:4 : BusSelector  OutputSignals=RadarSensor:4.time,RadarSensor:4.width,RadarSensor:4.OBJ_ID,RadarSensor:4.OBJ_Class,RadarSensor:4.OBJ_S_Azimuth,RadarSensor:4.OBJ_S_Elevation,RadarSensor:4.OBJ_S_Velocity,RadarSensor:4.OBJ_S_Range,RadarSensor:4.OBJ_RCS
  Bus Selector:RadarSensor:4_OBJ_Class_BS : BusSelector  OutputSignals=RadarSensor:4.OBJ_Class_1,RadarSensor:4.OBJ_Class_2,RadarSensor:4.OBJ_Class_3,RadarSensor:4.OBJ_Class_4,RadarSensor:4.OBJ_Class_5,RadarSensor:4.OBJ_Class_6,RadarSensor:4.OBJ_Class_7,RadarSensor:4.OBJ_Class_8,RadarSensor:4.OBJ_Class_9,RadarSensor:4.OBJ_Class_10,RadarSensor:4.OBJ_Class_11,RadarSensor:4.OBJ_Class_12,RadarSensor:4.OBJ_Class_13,RadarSensor:4.OBJ_Class_14,RadarSensor:4.OBJ_Class_15,RadarSensor:4.OBJ_Class_16,RadarSensor:4.OBJ_Class_17,RadarSensor:4.OBJ_Class_18,RadarSensor:4.OBJ_Class_19,RadarSensor:4.OBJ_Class_20,RadarSensor:4.OBJ_Class_21,RadarSensor:4.OBJ_Class_22,RadarSensor:4.OBJ_Class_23,RadarSensor:4.OBJ_Class_24,RadarSensor:4.OBJ_Class_25,RadarSensor:4.OBJ_Class_26,RadarSensor:4.OBJ_Class_27,RadarSensor:4.OBJ_Class_28,RadarSensor:4.OBJ_Class_29,RadarSensor:4.OBJ_Class_30,RadarSensor:4.OBJ_Class_31,RadarSensor:4.OBJ_Class_32,RadarSensor:4.OBJ_Class_33,RadarSensor:4.OBJ_Class_34,RadarSensor:4.OBJ_Class_35,RadarSensor:4.OBJ_Class_36,RadarSensor:4.OBJ_Class_37,RadarSensor:4.OBJ_Class_38,RadarSensor:4.OBJ_Class_39,RadarSensor:4.OBJ_Class_40,RadarSensor:4.OBJ_Class_41,RadarSensor:4.OBJ_Class_42,RadarSensor:4.OBJ_Class_43,RadarSensor:4.OBJ_Class_44,RadarSensor:4.OBJ_Class_45,RadarSensor:4.OBJ_Class_46,RadarSensor:4.OBJ_Class_47,RadarSensor:4.OBJ_Class_48,RadarSensor:4.OBJ_Class_49,RadarSensor:4.OBJ_Class_50,RadarSensor:4.OBJ_Class_51,RadarSensor:4.OBJ_Class_52,RadarSensor:4.OBJ_Class_53,RadarSensor:4.OBJ_Class_54,RadarSensor:4.OBJ_Class_55,RadarSensor:4.OBJ_Class_56,RadarSensor:4.OBJ_Class_57,RadarSensor:4.OBJ_Class_58,RadarSensor:4.OBJ_Class_59,RadarSensor:4.OBJ_Class_60,RadarSensor:4.OBJ_Class_61,RadarSensor:4.OBJ_Class_62,RadarSensor:4.OBJ_Class_63,RadarSensor:4.OBJ_Class_64
  Bus Selector:RadarSensor:4_OBJ_ID_BS : BusSelector  OutputSignals=RadarSensor:4.OBJ_ID_1,RadarSensor:4.OBJ_ID_2,RadarSensor:4.OBJ_ID_3,RadarSensor:4.OBJ_ID_4,RadarSensor:4.OBJ_ID_5,RadarSensor:4.OBJ_ID_6,RadarSensor:4.OBJ_ID_7,RadarSensor:4.OBJ_ID_8,RadarSensor:4.OBJ_ID_9,RadarSensor:4.OBJ_ID_10,RadarSensor:4.OBJ_ID_11,RadarSensor:4.OBJ_ID_12,RadarSensor:4.OBJ_ID_13,RadarSensor:4.OBJ_ID_14,RadarSensor:4.OBJ_ID_15,RadarSensor:4.OBJ_ID_16,RadarSensor:4.OBJ_ID_17,RadarSensor:4.OBJ_ID_18,RadarSensor:4.OBJ_ID_19,RadarSensor:4.OBJ_ID_20,RadarSensor:4.OBJ_ID_21,RadarSensor:4.OBJ_ID_22,RadarSensor:4.OBJ_ID_23,RadarSensor:4.OBJ_ID_24,RadarSensor:4.OBJ_ID_25,RadarSensor:4.OBJ_ID_26,RadarSensor:4.OBJ_ID_27,RadarSensor:4.OBJ_ID_28,RadarSensor:4.OBJ_ID_29,RadarSensor:4.OBJ_ID_30,RadarSensor:4.OBJ_ID_31,RadarSensor:4.OBJ_ID_32,RadarSensor:4.OBJ_ID_33,RadarSensor:4.OBJ_ID_34,RadarSensor:4.OBJ_ID_35,RadarSensor:4.OBJ_ID_36,RadarSensor:4.OBJ_ID_37,RadarSensor:4.OBJ_ID_38,RadarSensor:4.OBJ_ID_39,RadarSensor:4.OBJ_ID_40,RadarSensor:4.OBJ_ID_41,RadarSensor:4.OBJ_ID_42,RadarSensor:4.OBJ_ID_43,RadarSensor:4.OBJ_ID_44,RadarSensor:4.OBJ_ID_45,RadarSensor:4.OBJ_ID_46,RadarSensor:4.OBJ_ID_47,RadarSensor:4.OBJ_ID_48,RadarSensor:4.OBJ_ID_49,RadarSensor:4.OBJ_ID_50,RadarSensor:4.OBJ_ID_51,RadarSensor:4.OBJ_ID_52,RadarSensor:4.OBJ_ID_53,RadarSensor:4.OBJ_ID_54,RadarSensor:4.OBJ_ID_55,RadarSensor:4.OBJ_ID_56,RadarSensor:4.OBJ_ID_57,RadarSensor:4.OBJ_ID_58,RadarSensor:4.OBJ_ID_59,RadarSensor:4.OBJ_ID_60,RadarSensor:4.OBJ_ID_61,RadarSensor:4.OBJ_ID_62,RadarSensor:4.OBJ_ID_63,RadarSensor:4.OBJ_ID_64
  Bus Selector:RadarSensor:4_OBJ_RCS_BS : BusSelector  OutputSignals=RadarSensor:4.OBJ_RCS_1,RadarSensor:4.OBJ_RCS_2,RadarSensor:4.OBJ_RCS_3,RadarSensor:4.OBJ_RCS_4,RadarSensor:4.OBJ_RCS_5,RadarSensor:4.OBJ_RCS_6,RadarSensor:4.OBJ_RCS_7,RadarSensor:4.OBJ_RCS_8,RadarSensor:4.OBJ_RCS_9,RadarSensor:4.OBJ_RCS_10,RadarSensor:4.OBJ_RCS_11,RadarSensor:4.OBJ_RCS_12,RadarSensor:4.OBJ_RCS_13,RadarSensor:4.OBJ_RCS_14,RadarSensor:4.OBJ_RCS_15,RadarSensor:4.OBJ_RCS_16,RadarSensor:4.OBJ_RCS_17,RadarSensor:4.OBJ_RCS_18,RadarSensor:4.OBJ_RCS_19,RadarSensor:4.OBJ_RCS_20,RadarSensor:4.OBJ_RCS_21,RadarSensor:4.OBJ_RCS_22,RadarSensor:4.OBJ_RCS_23,RadarSensor:4.OBJ_RCS_24,RadarSensor:4.OBJ_RCS_25,RadarSensor:4.OBJ_RCS_26,RadarSensor:4.OBJ_RCS_27,RadarSensor:4.OBJ_RCS_28,RadarSensor:4.OBJ_RCS_29,RadarSensor:4.OBJ_RCS_30,RadarSensor:4.OBJ_RCS_31,RadarSensor:4.OBJ_RCS_32,RadarSensor:4.OBJ_RCS_33,RadarSensor:4.OBJ_RCS_34,RadarSensor:4.OBJ_RCS_35,RadarSensor:4.OBJ_RCS_36,RadarSensor:4.OBJ_RCS_37,RadarSensor:4.OBJ_RCS_38,RadarSensor:4.OBJ_RCS_39,RadarSensor:4.OBJ_RCS_40,RadarSensor:4.OBJ_RCS_41,RadarSensor:4.OBJ_RCS_42,RadarSensor:4.OBJ_RCS_43,RadarSensor:4.OBJ_RCS_44,RadarSensor:4.OBJ_RCS_45,RadarSensor:4.OBJ_RCS_46,RadarSensor:4.OBJ_RCS_47,RadarSensor:4.OBJ_RCS_48,RadarSensor:4.OBJ_RCS_49,RadarSensor:4.OBJ_RCS_50,RadarSensor:4.OBJ_RCS_51,RadarSensor:4.OBJ_RCS_52,RadarSensor:4.OBJ_RCS_53,RadarSensor:4.OBJ_RCS_54,RadarSensor:4.OBJ_RCS_55,RadarSensor:4.OBJ_RCS_56,RadarSensor:4.OBJ_RCS_57,RadarSensor:4.OBJ_RCS_58,RadarSensor:4.OBJ_RCS_59,RadarSensor:4.OBJ_RCS_60,RadarSensor:4.OBJ_RCS_61,RadarSensor:4.OBJ_RCS_62,RadarSensor:4.OBJ_RCS_63,RadarSensor:4.OBJ_RCS_64
  Bus Selector:RadarSensor:4_OBJ_S_Azimuth_BS : BusSelector  OutputSignals=RadarSensor:4.OBJ_S_Azimuth_1,RadarSensor:4.OBJ_S_Azimuth_2,RadarSensor:4.OBJ_S_Azimuth_3,RadarSensor:4.OBJ_S_Azimuth_4,RadarSensor:4.OBJ_S_Azimuth_5,RadarSensor:4.OBJ_S_Azimuth_6,RadarSensor:4.OBJ_S_Azimuth_7,RadarSensor:4.OBJ_S_Azimuth_8,RadarSensor:4.OBJ_S_Azimuth_9,RadarSensor:4.OBJ_S_Azimuth_10,RadarSensor:4.OBJ_S_Azimuth_11,RadarSensor:4.OBJ_S_Azimuth_12,RadarSensor:4.OBJ_S_Azimuth_13,RadarSensor:4.OBJ_S_Azimuth_14,RadarSensor:4.OBJ_S_Azimuth_15,RadarSensor:4.OBJ_S_Azimuth_16,RadarSensor:4.OBJ_S_Azimuth_17,RadarSensor:4.OBJ_S_Azimuth_18,RadarSensor:4.OBJ_S_Azimuth_19,RadarSensor:4.OBJ_S_Azimuth_20,RadarSensor:4.OBJ_S_Azimuth_21,RadarSensor:4.OBJ_S_Azimuth_22,RadarSensor:4.OBJ_S_Azimuth_23,RadarSensor:4.OBJ_S_Azimuth_24,RadarSensor:4.OBJ_S_Azimuth_25,RadarSensor:4.OBJ_S_Azimuth_26,RadarSensor:4.OBJ_S_Azimuth_27,RadarSensor:4.OBJ_S_Azimuth_28,RadarSensor:4.OBJ_S_Azimuth_29,RadarSensor:4.OBJ_S_Azimuth_30,RadarSensor:4.OBJ_S_Azimuth_31,RadarSensor:4.OBJ_S_Azimuth_32,RadarSensor:4.OBJ_S_Azimuth_33,RadarSensor:4.OBJ_S_Azimuth_34,RadarSensor:4.OBJ_S_Azimuth_35,RadarSensor:4.OBJ_S_Azimuth_36,RadarSensor:4.OBJ_S_Azimuth_37,RadarSensor:4.OBJ_S_Azimuth_38,RadarSensor:4.OBJ_S_Azimuth_39,RadarSensor:4.OBJ_S_Azimuth_40,RadarSensor:4.OBJ_S_Azimuth_41,RadarSensor:4.OBJ_S_Azimuth_42,RadarSensor:4.OBJ_S_Azimuth_43,RadarSensor:4.OBJ_S_Azimuth_44,RadarSensor:4.OBJ_S_Azimuth_45,RadarSensor:4.OBJ_S_Azimuth_46,RadarSensor:4.OBJ_S_Azimuth_47,RadarSensor:4.OBJ_S_Azimuth_48,RadarSensor:4.OBJ_S_Azimuth_49,RadarSensor:4.OBJ_S_Azimuth_50,RadarSensor:4.OBJ_S_Azimuth_51,RadarSensor:4.OBJ_S_Azimuth_52,RadarSensor:4.OBJ_S_Azimuth_53,RadarSensor:4.OBJ_S_Azimuth_54,RadarSensor:4.OBJ_S_Azimuth_55,RadarSensor:4.OBJ_S_Azimuth_56,RadarSensor:4.OBJ_S_Azimuth_57,RadarSensor:4.OBJ_S_Azimuth_58,RadarSensor:4.OBJ_S_Azimuth_59,RadarSensor:4.OBJ_S_Azimuth_60,RadarSensor:4.OBJ_S_Azimuth_61,RadarSensor:4.OBJ_S_Azimuth_62,RadarSensor:4.OBJ_S_Azimuth_63,RadarSensor:4.OBJ_S_Azimuth_64
  Bus Selector:RadarSensor:4_OBJ_S_Elevation_BS : BusSelector  OutputSignals=RadarSensor:4.OBJ_S_Elevation_1,RadarSensor:4.OBJ_S_Elevation_2,RadarSensor:4.OBJ_S_Elevation_3,RadarSensor:4.OBJ_S_Elevation_4,RadarSensor:4.OBJ_S_Elevation_5,RadarSensor:4.OBJ_S_Elevation_6,RadarSensor:4.OBJ_S_Elevation_7,RadarSensor:4.OBJ_S_Elevation_8,RadarSensor:4.OBJ_S_Elevation_9,RadarSensor:4.OBJ_S_Elevation_10,RadarSensor:4.OBJ_S_Elevation_11,RadarSensor:4.OBJ_S_Elevation_12,RadarSensor:4.OBJ_S_Elevation_13,RadarSensor:4.OBJ_S_Elevation_14,RadarSensor:4.OBJ_S_Elevation_15,RadarSensor:4.OBJ_S_Elevation_16,RadarSensor:4.OBJ_S_Elevation_17,RadarSensor:4.OBJ_S_Elevation_18,RadarSensor:4.OBJ_S_Elevation_19,RadarSensor:4.OBJ_S_Elevation_20,RadarSensor:4.OBJ_S_Elevation_21,RadarSensor:4.OBJ_S_Elevation_22,RadarSensor:4.OBJ_S_Elevation_23,RadarSensor:4.OBJ_S_Elevation_24,RadarSensor:4.OBJ_S_Elevation_25,RadarSensor:4.OBJ_S_Elevation_26,RadarSensor:4.OBJ_S_Elevation_27,RadarSensor:4.OBJ_S_Elevation_28,RadarSensor:4.OBJ_S_Elevation_29,RadarSensor:4.OBJ_S_Elevation_30,RadarSensor:4.OBJ_S_Elevation_31,RadarSensor:4.OBJ_S_Elevation_32,RadarSensor:4.OBJ_S_Elevation_33,RadarSensor:4.OBJ_S_Elevation_34,RadarSensor:4.OBJ_S_Elevation_35,RadarSensor:4.OBJ_S_Elevation_36,RadarSensor:4.OBJ_S_Elevation_37,RadarSensor:4.OBJ_S_Elevation_38,RadarSensor:4.OBJ_S_Elevation_39,RadarSensor:4.OBJ_S_Elevation_40,RadarSensor:4.OBJ_S_Elevation_41,RadarSensor:4.OBJ_S_Elevation_42,RadarSensor:4.OBJ_S_Elevation_43,RadarSensor:4.OBJ_S_Elevation_44,RadarSensor:4.OBJ_S_Elevation_45,RadarSensor:4.OBJ_S_Elevation_46,RadarSensor:4.OBJ_S_Elevation_47,RadarSensor:4.OBJ_S_Elevation_48,RadarSensor:4.OBJ_S_Elevation_49,RadarSensor:4.OBJ_S_Elevation_50,RadarSensor:4.OBJ_S_Elevation_51,RadarSensor:4.OBJ_S_Elevation_52,RadarSensor:4.OBJ_S_Elevation_53,RadarSensor:4.OBJ_S_Elevation_54,RadarSensor:4.OBJ_S_Elevation_55,RadarSensor:4.OBJ_S_Elevation_56,RadarSensor:4.OBJ_S_Elevation_57,RadarSensor:4.OBJ_S_Elevation_58,RadarSensor:4.OBJ_S_Elevation_59,RadarSensor:4.OBJ_S_Elevation_60,RadarSensor:4.OBJ_S_Elevation_61,RadarSensor:4.OBJ_S_Elevation_62,RadarSensor:4.OBJ_S_Elevation_63,RadarSensor:4.OBJ_S_Elevation_64
  Bus Selector:RadarSensor:4_OBJ_S_Range_BS : BusSelector  OutputSignals=RadarSensor:4.OBJ_S_Range_1,RadarSensor:4.OBJ_S_Range_2,RadarSensor:4.OBJ_S_Range_3,RadarSensor:4.OBJ_S_Range_4,RadarSensor:4.OBJ_S_Range_5,RadarSensor:4.OBJ_S_Range_6,RadarSensor:4.OBJ_S_Range_7,RadarSensor:4.OBJ_S_Range_8,RadarSensor:4.OBJ_S_Range_9,RadarSensor:4.OBJ_S_Range_10,RadarSensor:4.OBJ_S_Range_11,RadarSensor:4.OBJ_S_Range_12,RadarSensor:4.OBJ_S_Range_13,RadarSensor:4.OBJ_S_Range_14,RadarSensor:4.OBJ_S_Range_15,RadarSensor:4.OBJ_S_Range_16,RadarSensor:4.OBJ_S_Range_17,RadarSensor:4.OBJ_S_Range_18,RadarSensor:4.OBJ_S_Range_19,RadarSensor:4.OBJ_S_Range_20,RadarSensor:4.OBJ_S_Range_21,RadarSensor:4.OBJ_S_Range_22,RadarSensor:4.OBJ_S_Range_23,RadarSensor:4.OBJ_S_Range_24,RadarSensor:4.OBJ_S_Range_25,RadarSensor:4.OBJ_S_Range_26,RadarSensor:4.OBJ_S_Range_27,RadarSensor:4.OBJ_S_Range_28,RadarSensor:4.OBJ_S_Range_29,RadarSensor:4.OBJ_S_Range_30,RadarSensor:4.OBJ_S_Range_31,RadarSensor:4.OBJ_S_Range_32,RadarSensor:4.OBJ_S_Range_33,RadarSensor:4.OBJ_S_Range_34,RadarSensor:4.OBJ_S_Range_35,RadarSensor:4.OBJ_S_Range_36,RadarSensor:4.OBJ_S_Range_37,RadarSensor:4.OBJ_S_Range_38,RadarSensor:4.OBJ_S_Range_39,RadarSensor:4.OBJ_S_Range_40,RadarSensor:4.OBJ_S_Range_41,RadarSensor:4.OBJ_S_Range_42,RadarSensor:4.OBJ_S_Range_43,RadarSensor:4.OBJ_S_Range_44,RadarSensor:4.OBJ_S_Range_45,RadarSensor:4.OBJ_S_Range_46,RadarSensor:4.OBJ_S_Range_47,RadarSensor:4.OBJ_S_Range_48,RadarSensor:4.OBJ_S_Range_49,RadarSensor:4.OBJ_S_Range_50,RadarSensor:4.OBJ_S_Range_51,RadarSensor:4.OBJ_S_Range_52,RadarSensor:4.OBJ_S_Range_53,RadarSensor:4.OBJ_S_Range_54,RadarSensor:4.OBJ_S_Range_55,RadarSensor:4.OBJ_S_Range_56,RadarSensor:4.OBJ_S_Range_57,RadarSensor:4.OBJ_S_Range_58,RadarSensor:4.OBJ_S_Range_59,RadarSensor:4.OBJ_S_Range_60,RadarSensor:4.OBJ_S_Range_61,RadarSensor:4.OBJ_S_Range_62,RadarSensor:4.OBJ_S_Range_63,RadarSensor:4.OBJ_S_Range_64
  Bus Selector:RadarSensor:4_OBJ_S_Velocity_BS : BusSelector  OutputSignals=RadarSensor:4.OBJ_S_Velocity_1,RadarSensor:4.OBJ_S_Velocity_2,RadarSensor:4.OBJ_S_Velocity_3,RadarSensor:4.OBJ_S_Velocity_4,RadarSensor:4.OBJ_S_Velocity_5,RadarSensor:4.OBJ_S_Velocity_6,RadarSensor:4.OBJ_S_Velocity_7,RadarSensor:4.OBJ_S_Velocity_8,RadarSensor:4.OBJ_S_Velocity_9,RadarSensor:4.OBJ_S_Velocity_10,RadarSensor:4.OBJ_S_Velocity_11,RadarSensor:4.OBJ_S_Velocity_12,RadarSensor:4.OBJ_S_Velocity_13,RadarSensor:4.OBJ_S_Velocity_14,RadarSensor:4.OBJ_S_Velocity_15,RadarSensor:4.OBJ_S_Velocity_16,RadarSensor:4.OBJ_S_Velocity_17,RadarSensor:4.OBJ_S_Velocity_18,RadarSensor:4.OBJ_S_Velocity_19,RadarSensor:4.OBJ_S_Velocity_20,RadarSensor:4.OBJ_S_Velocity_21,RadarSensor:4.OBJ_S_Velocity_22,RadarSensor:4.OBJ_S_Velocity_23,RadarSensor:4.OBJ_S_Velocity_24,RadarSensor:4.OBJ_S_Velocity_25,RadarSensor:4.OBJ_S_Velocity_26,RadarSensor:4.OBJ_S_Velocity_27,RadarSensor:4.OBJ_S_Velocity_28,RadarSensor:4.OBJ_S_Velocity_29,RadarSensor:4.OBJ_S_Velocity_30,RadarSensor:4.OBJ_S_Velocity_31,RadarSensor:4.OBJ_S_Velocity_32,RadarSensor:4.OBJ_S_Velocity_33,RadarSensor:4.OBJ_S_Velocity_34,RadarSensor:4.OBJ_S_Velocity_35,RadarSensor:4.OBJ_S_Velocity_36,RadarSensor:4.OBJ_S_Velocity_37,RadarSensor:4.OBJ_S_Velocity_38,RadarSensor:4.OBJ_S_Velocity_39,RadarSensor:4.OBJ_S_Velocity_40,RadarSensor:4.OBJ_S_Velocity_41,RadarSensor:4.OBJ_S_Velocity_42,RadarSensor:4.OBJ_S_Velocity_43,RadarSensor:4.OBJ_S_Velocity_44,RadarSensor:4.OBJ_S_Velocity_45,RadarSensor:4.OBJ_S_Velocity_46,RadarSensor:4.OBJ_S_Velocity_47,RadarSensor:4.OBJ_S_Velocity_48,RadarSensor:4.OBJ_S_Velocity_49,RadarSensor:4.OBJ_S_Velocity_50,RadarSensor:4.OBJ_S_Velocity_51,RadarSensor:4.OBJ_S_Velocity_52,RadarSensor:4.OBJ_S_Velocity_53,RadarSensor:4.OBJ_S_Velocity_54,RadarSensor:4.OBJ_S_Velocity_55,RadarSensor:4.OBJ_S_Velocity_56,RadarSensor:4.OBJ_S_Velocity_57,RadarSensor:4.OBJ_S_Velocity_58,RadarSensor:4.OBJ_S_Velocity_59,RadarSensor:4.OBJ_S_Velocity_60,RadarSensor:4.OBJ_S_Velocity_61,RadarSensor:4.OBJ_S_Velocity_62,RadarSensor:4.OBJ_S_Velocity_63,RadarSensor:4.OBJ_S_Velocity_64
  Bus Selector:TrafficLightPerception:0 : BusSelector  OutputSignals=TrafficLightPerception:0.Timestamp,TrafficLightPerception:0.width,TrafficLightPerception:0.TrafficLight_Direction,TrafficLightPerception:0.TrafficLight_State,TrafficLightPerception:0.TrafficLight_Timer
  Bus Selector:UltrasonicSensor:0 : BusSelector  OutputSignals=UltrasonicSensor:0.time,UltrasonicSensor:0.width,UltrasonicSensor:0.distance
  Bus Selector:UltrasonicSensor:1 : BusSelector  OutputSignals=UltrasonicSensor:1.time,UltrasonicSensor:1.width,UltrasonicSensor:1.distance
  Bus Selector:UltrasonicSensor:10 : BusSelector  OutputSignals=UltrasonicSensor:10.time,UltrasonicSensor:10.width,UltrasonicSensor:10.distance
  Bus Selector:UltrasonicSensor:11 : BusSelector  OutputSignals=UltrasonicSensor:11.time,UltrasonicSensor:11.width,UltrasonicSensor:11.distance
  Bus Selector:UltrasonicSensor:2 : BusSelector  OutputSignals=UltrasonicSensor:2.time,UltrasonicSensor:2.width,UltrasonicSensor:2.distance
  Bus Selector:UltrasonicSensor:3 : BusSelector  OutputSignals=UltrasonicSensor:3.time,UltrasonicSensor:3.width,UltrasonicSensor:3.distance
  Bus Selector:UltrasonicSensor:4 : BusSelector  OutputSignals=UltrasonicSensor:4.time,UltrasonicSensor:4.width,UltrasonicSensor:4.distance
  Bus Selector:UltrasonicSensor:5 : BusSelector  OutputSignals=UltrasonicSensor:5.time,UltrasonicSensor:5.width,UltrasonicSensor:5.distance
  Bus Selector:UltrasonicSensor:6 : BusSelector  OutputSignals=UltrasonicSensor:6.time,UltrasonicSensor:6.width,UltrasonicSensor:6.distance
  Bus Selector:UltrasonicSensor:7 : BusSelector  OutputSignals=UltrasonicSensor:7.time,UltrasonicSensor:7.width,UltrasonicSensor:7.distance
  Bus Selector:UltrasonicSensor:8 : BusSelector  OutputSignals=UltrasonicSensor:8.time,UltrasonicSensor:8.width,UltrasonicSensor:8.distance
  Bus Selector:UltrasonicSensor:9 : BusSelector  OutputSignals=UltrasonicSensor:9.time,UltrasonicSensor:9.width,UltrasonicSensor:9.distance
  FreeSpacePerception:0.time : Outport
  FreeSpacePerception:0.width : Outport  Port=2
  FreeSpacePerception:0.x : Outport  Port=3
  FreeSpacePerception:0.y : Outport  Port=4
  LaneInfoPerception:0.Timestamp : Outport  Port=5
  LaneInfoPerception:0.width : Outport  Port=6
  LaneInfoPerception:0.Lane_ID : Outport  Port=7
  LaneInfoPerception:0.Lane_Distance : Outport  Port=8
  LaneInfoPerception:0.Lane_Car_Distance_Left : Outport  Port=9
  LaneInfoPerception:0.Lane_Car_Distance_Right : Outport  Port=10
  LaneInfoPerception:0.Lane_Curvature : Outport  Port=11
  LaneInfoPerception:0.Lane_Coefficient_C0 : Outport  Port=12
  LaneInfoPerception:0.Lane_Coefficient_C1 : Outport  Port=13
  LaneInfoPerception:0.Lane_Coefficient_C2 : Outport  Port=14
  LaneInfoPerception:0.Lane_Coefficient_C3 : Outport  Port=15
  LaneInfoPerception:0.Lane_Class : Outport  Port=16
  ObjectPerception:0.Timestamp : Outport  Port=17
  ObjectPerception:0.width : Outport  Port=18
  ObjectPerception:0.OBJ_ID : Outport  Port=19
  ObjectPerception:0.OBJ_Class : Outport  Port=20
  ObjectPerception:0.OBJ_X : Outport  Port=21
  ObjectPerception:0.OBJ_Y : Outport  Port=22
  ObjectPerception:0.OBJ_Z : Outport  Port=23
  ObjectPerception:0.OBJ_Velocity : Outport  Port=24
  ObjectPerception:0.OBJ_Length : Outport  Port=25
  ObjectPerception:0.OBJ_Width : Outport  Port=26
  ObjectPerception:0.OBJ_Height : Outport  Port=27
  ParkingLotsPerception:0.time : Outport  Port=28
  ParkingLotsPerception:0.width : Outport  Port=29
  ParkingLotsPerception:0.x1 : Outport  Port=30
  ParkingLotsPerception:0.y1 : Outport  Port=31
  ParkingLotsPerception:0.x2 : Outport  Port=32
  ParkingLotsPerception:0.y2 : Outport  Port=33
  ParkingLotsPerception:0.x3 : Outport  Port=34
  ParkingLotsPerception:0.y3 : Outport  Port=35
  ParkingLotsPerception:0.x4 : Outport  Port=36
  ParkingLotsPerception:0.y4 : Outport  Port=37
  TrafficLightPerception:0.Timestamp : Outport  Port=38
  TrafficLightPerception:0.width : Outport  Port=39
  TrafficLightPerception:0.TrafficLight_Direction : Outport  Port=40
  TrafficLightPerception:0.TrafficLight_State : Outport  Port=41
  TrafficLightPerception:0.TrafficLight_Timer : Outport  Port=42
  RadarSensor:0.time : Outport  Port=43
  RadarSensor:0.width : Outport  Port=44
  RadarSensor:0.OBJ_ID : Outport  Port=45
  RadarSensor:0.OBJ_ID_1 : Outport  Port=46
  RadarSensor:0.OBJ_ID_2 : Outport  Port=47
  RadarSensor:0.OBJ_ID_3 : Outport  Port=48
  RadarSensor:0.OBJ_ID_4 : Outport  Port=49
  RadarSensor:0.OBJ_ID_5 : Outport  Port=50
  RadarSensor:0.OBJ_ID_6 : Outport  Port=51
  RadarSensor:0.OBJ_ID_7 : Outport  Port=52
  RadarSensor:0.OBJ_ID_8 : Outport  Port=53
  RadarSensor:0.OBJ_ID_9 : Outport  Port=54
  RadarSensor:0.OBJ_ID_10 : Outport  Port=55
  RadarSensor:0.OBJ_ID_11 : Outport  Port=56
  RadarSensor:0.OBJ_ID_12 : Outport  Port=57
  RadarSensor:0.OBJ_ID_13 : Outport  Port=58
  RadarSensor:0.OBJ_ID_14 : Outport  Port=59
  RadarSensor:0.OBJ_ID_15 : Outport  Port=60
  RadarSensor:0.OBJ_ID_16 : Outport  Port=61
  RadarSensor:0.OBJ_ID_17 : Outport  Port=62
  RadarSensor:0.OBJ_ID_18 : Outport  Port=63
  RadarSensor:0.OBJ_ID_19 : Outport  Port=64
  RadarSensor:0.OBJ_ID_20 : Outport  Port=65
  RadarSensor:0.OBJ_ID_21 : Outport  Port=66
  RadarSensor:0.OBJ_ID_22 : Outport  Port=67
  RadarSensor:0.OBJ_ID_23 : Outport  Port=68
  RadarSensor:0.OBJ_ID_24 : Outport  Port=69
  RadarSensor:0.OBJ_ID_25 : Outport  Port=70
  RadarSensor:0.OBJ_ID_26 : Outport  Port=71
  RadarSensor:0.OBJ_ID_27 : Outport  Port=72
  RadarSensor:0.OBJ_ID_28 : Outport  Port=73
  RadarSensor:0.OBJ_ID_29 : Outport  Port=74
  RadarSensor:0.OBJ_ID_30 : Outport  Port=75
  RadarSensor:0.OBJ_ID_31 : Outport  Port=76
  RadarSensor:0.OBJ_ID_32 : Outport  Port=77
  RadarSensor:0.OBJ_ID_33 : Outport  Port=78
  RadarSensor:0.OBJ_ID_34 : Outport  Port=79
  RadarSensor:0.OBJ_ID_35 : Outport  Port=80
  RadarSensor:0.OBJ_ID_36 : Outport  Port=81
  RadarSensor:0.OBJ_ID_37 : Outport  Port=82
  RadarSensor:0.OBJ_ID_38 : Outport  Port=83
  RadarSensor:0.OBJ_ID_39 : Outport  Port=84
  RadarSensor:0.OBJ_ID_40 : Outport  Port=85
  RadarSensor:0.OBJ_ID_41 : Outport  Port=86
  RadarSensor:0.OBJ_ID_42 : Outport  Port=87
  RadarSensor:0.OBJ_ID_43 : Outport  Port=88
  RadarSensor:0.OBJ_ID_44 : Outport  Port=89
  RadarSensor:0.OBJ_ID_45 : Outport  Port=90
  RadarSensor:0.OBJ_ID_46 : Outport  Port=91
  RadarSensor:0.OBJ_ID_47 : Outport  Port=92
  RadarSensor:0.OBJ_ID_48 : Outport  Port=93
  RadarSensor:0.OBJ_ID_49 : Outport  Port=94
  RadarSensor:0.OBJ_ID_50 : Outport  Port=95
  RadarSensor:0.OBJ_ID_51 : Outport  Port=96
  RadarSensor:0.OBJ_ID_52 : Outport  Port=97
  RadarSensor:0.OBJ_ID_53 : Outport  Port=98
  RadarSensor:0.OBJ_ID_54 : Outport  Port=99
  RadarSensor:0.OBJ_ID_55 : Outport  Port=100
  RadarSensor:0.OBJ_ID_56 : Outport  Port=101
  RadarSensor:0.OBJ_ID_57 : Outport  Port=102
  RadarSensor:0.OBJ_ID_58 : Outport  Port=103
  RadarSensor:0.OBJ_ID_59 : Outport  Port=104
  RadarSensor:0.OBJ_ID_60 : Outport  Port=105
  RadarSensor:0.OBJ_ID_61 : Outport  Port=106
  RadarSensor:0.OBJ_ID_62 : Outport  Port=107
  RadarSensor:0.OBJ_ID_63 : Outport  Port=108
  RadarSensor:0.OBJ_ID_64 : Outport  Port=109
  RadarSensor:0.OBJ_Class : Outport  Port=110
  RadarSensor:0.OBJ_Class_1 : Outport  Port=111
  RadarSensor:0.OBJ_Class_2 : Outport  Port=112
  RadarSensor:0.OBJ_Class_3 : Outport  Port=113
  RadarSensor:0.OBJ_Class_4 : Outport  Port=114
  RadarSensor:0.OBJ_Class_5 : Outport  Port=115
  RadarSensor:0.OBJ_Class_6 : Outport  Port=116
  RadarSensor:0.OBJ_Class_7 : Outport  Port=117
  RadarSensor:0.OBJ_Class_8 : Outport  Port=118
  RadarSensor:0.OBJ_Class_9 : Outport  Port=119
  RadarSensor:0.OBJ_Class_10 : Outport  Port=120
  RadarSensor:0.OBJ_Class_11 : Outport  Port=121
  RadarSensor:0.OBJ_Class_12 : Outport  Port=122
  RadarSensor:0.OBJ_Class_13 : Outport  Port=123
  RadarSensor:0.OBJ_Class_14 : Outport  Port=124
  RadarSensor:0.OBJ_Class_15 : Outport  Port=125
  RadarSensor:0.OBJ_Class_16 : Outport  Port=126
  RadarSensor:0.OBJ_Class_17 : Outport  Port=127
  RadarSensor:0.OBJ_Class_18 : Outport  Port=128
  RadarSensor:0.OBJ_Class_19 : Outport  Port=129
  RadarSensor:0.OBJ_Class_20 : Outport  Port=130
  RadarSensor:0.OBJ_Class_21 : Outport  Port=131
  RadarSensor:0.OBJ_Class_22 : Outport  Port=132
  RadarSensor:0.OBJ_Class_23 : Outport  Port=133
  RadarSensor:0.OBJ_Class_24 : Outport  Port=134
  RadarSensor:0.OBJ_Class_25 : Outport  Port=135
  RadarSensor:0.OBJ_Class_26 : Outport  Port=136
  RadarSensor:0.OBJ_Class_27 : Outport  Port=137
  RadarSensor:0.OBJ_Class_28 : Outport  Port=138
  RadarSensor:0.OBJ_Class_29 : Outport  Port=139
  RadarSensor:0.OBJ_Class_30 : Outport  Port=140
  RadarSensor:0.OBJ_Class_31 : Outport  Port=141
  RadarSensor:0.OBJ_Class_32 : Outport  Port=142
  RadarSensor:0.OBJ_Class_33 : Outport  Port=143
  RadarSensor:0.OBJ_Class_34 : Outport  Port=144
  RadarSensor:0.OBJ_Class_35 : Outport  Port=145
  RadarSensor:0.OBJ_Class_36 : Outport  Port=146
  RadarSensor:0.OBJ_Class_37 : Outport  Port=147
  RadarSensor:0.OBJ_Class_38 : Outport  Port=148
  RadarSensor:0.OBJ_Class_39 : Outport  Port=149
  RadarSensor:0.OBJ_Class_40 : Outport  Port=150
  RadarSensor:0.OBJ_Class_41 : Outport  Port=151
  RadarSensor:0.OBJ_Class_42 : Outport  Port=152
  RadarSensor:0.OBJ_Class_43 : Outport  Port=153
  RadarSensor:0.OBJ_Class_44 : Outport  Port=154
  RadarSensor:0.OBJ_Class_45 : Outport  Port=155
  RadarSensor:0.OBJ_Class_46 : Outport  Port=156
  RadarSensor:0.OBJ_Class_47 : Outport  Port=157
  RadarSensor:0.OBJ_Class_48 : Outport  Port=158
  RadarSensor:0.OBJ_Class_49 : Outport  Port=159
  RadarSensor:0.OBJ_Class_50 : Outport  Port=160
  RadarSensor:0.OBJ_Class_51 : Outport  Port=161
  RadarSensor:0.OBJ_Class_52 : Outport  Port=162
  RadarSensor:0.OBJ_Class_53 : Outport  Port=163
  RadarSensor:0.OBJ_Class_54 : Outport  Port=164
  RadarSensor:0.OBJ_Class_55 : Outport  Port=165
  RadarSensor:0.OBJ_Class_56 : Outport  Port=166
  RadarSensor:0.OBJ_Class_57 : Outport  Port=167
  RadarSensor:0.OBJ_Class_58 : Outport  Port=168
  RadarSensor:0.OBJ_Class_59 : Outport  Port=169
  RadarSensor:0.OBJ_Class_60 : Outport  Port=170
  RadarSensor:0.OBJ_Class_61 : Outport  Port=171
  RadarSensor:0.OBJ_Class_62 : Outport  Port=172
  RadarSensor:0.OBJ_Class_63 : Outport  Port=173
  RadarSensor:0.OBJ_Class_64 : Outport  Port=174
  RadarSensor:0.OBJ_S_Azimuth : Outport  Port=175
  RadarSensor:0.OBJ_S_Azimuth_1 : Outport  Port=176
  RadarSensor:0.OBJ_S_Azimuth_2 : Outport  Port=177
  RadarSensor:0.OBJ_S_Azimuth_3 : Outport  Port=178
  RadarSensor:0.OBJ_S_Azimuth_4 : Outport  Port=179
  RadarSensor:0.OBJ_S_Azimuth_5 : Outport  Port=180
  RadarSensor:0.OBJ_S_Azimuth_6 : Outport  Port=181
  RadarSensor:0.OBJ_S_Azimuth_7 : Outport  Port=182
  RadarSensor:0.OBJ_S_Azimuth_8 : Outport  Port=183
  RadarSensor:0.OBJ_S_Azimuth_9 : Outport  Port=184
  RadarSensor:0.OBJ_S_Azimuth_10 : Outport  Port=185
  RadarSensor:0.OBJ_S_Azimuth_11 : Outport  Port=186
  RadarSensor:0.OBJ_S_Azimuth_12 : Outport  Port=187
  RadarSensor:0.OBJ_S_Azimuth_13 : Outport  Port=188
  RadarSensor:0.OBJ_S_Azimuth_14 : Outport  Port=189
  RadarSensor:0.OBJ_S_Azimuth_15 : Outport  Port=190
  RadarSensor:0.OBJ_S_Azimuth_16 : Outport  Port=191
  RadarSensor:0.OBJ_S_Azimuth_17 : Outport  Port=192
  RadarSensor:0.OBJ_S_Azimuth_18 : Outport  Port=193
  RadarSensor:0.OBJ_S_Azimuth_19 : Outport  Port=194
  RadarSensor:0.OBJ_S_Azimuth_20 : Outport  Port=195
  RadarSensor:0.OBJ_S_Azimuth_21 : Outport  Port=196
  RadarSensor:0.OBJ_S_Azimuth_22 : Outport  Port=197
  RadarSensor:0.OBJ_S_Azimuth_23 : Outport  Port=198
  RadarSensor:0.OBJ_S_Azimuth_24 : Outport  Port=199
  RadarSensor:0.OBJ_S_Azimuth_25 : Outport  Port=200
  RadarSensor:0.OBJ_S_Azimuth_26 : Outport  Port=201
  RadarSensor:0.OBJ_S_Azimuth_27 : Outport  Port=202
  RadarSensor:0.OBJ_S_Azimuth_28 : Outport  Port=203
  RadarSensor:0.OBJ_S_Azimuth_29 : Outport  Port=204
  RadarSensor:0.OBJ_S_Azimuth_30 : Outport  Port=205
  RadarSensor:0.OBJ_S_Azimuth_31 : Outport  Port=206
  RadarSensor:0.OBJ_S_Azimuth_32 : Outport  Port=207
  RadarSensor:0.OBJ_S_Azimuth_33 : Outport  Port=208
  RadarSensor:0.OBJ_S_Azimuth_34 : Outport  Port=209
  RadarSensor:0.OBJ_S_Azimuth_35 : Outport  Port=210
  RadarSensor:0.OBJ_S_Azimuth_36 : Outport  Port=211
  RadarSensor:0.OBJ_S_Azimuth_37 : Outport  Port=212
  RadarSensor:0.OBJ_S_Azimuth_38 : Outport  Port=213
  RadarSensor:0.OBJ_S_Azimuth_39 : Outport  Port=214
  RadarSensor:0.OBJ_S_Azimuth_40 : Outport  Port=215
  RadarSensor:0.OBJ_S_Azimuth_41 : Outport  Port=216
  RadarSensor:0.OBJ_S_Azimuth_42 : Outport  Port=217
  RadarSensor:0.OBJ_S_Azimuth_43 : Outport  Port=218
  RadarSensor:0.OBJ_S_Azimuth_44 : Outport  Port=219
  RadarSensor:0.OBJ_S_Azimuth_45 : Outport  Port=220
  RadarSensor:0.OBJ_S_Azimuth_46 : Outport  Port=221
  RadarSensor:0.OBJ_S_Azimuth_47 : Outport  Port=222
  RadarSensor:0.OBJ_S_Azimuth_48 : Outport  Port=223
  RadarSensor:0.OBJ_S_Azimuth_49 : Outport  Port=224
  RadarSensor:0.OBJ_S_Azimuth_50 : Outport  Port=225
  RadarSensor:0.OBJ_S_Azimuth_51 : Outport  Port=226
  RadarSensor:0.OBJ_S_Azimuth_52 : Outport  Port=227
  RadarSensor:0.OBJ_S_Azimuth_53 : Outport  Port=228
  RadarSensor:0.OBJ_S_Azimuth_54 : Outport  Port=229
  RadarSensor:0.OBJ_S_Azimuth_55 : Outport  Port=230
  RadarSensor:0.OBJ_S_Azimuth_56 : Outport  Port=231
  RadarSensor:0.OBJ_S_Azimuth_57 : Outport  Port=232
  RadarSensor:0.OBJ_S_Azimuth_58 : Outport  Port=233
  RadarSensor:0.OBJ_S_Azimuth_59 : Outport  Port=234
  RadarSensor:0.OBJ_S_Azimuth_60 : Outport  Port=235
  RadarSensor:0.OBJ_S_Azimuth_61 : Outport  Port=236
  RadarSensor:0.OBJ_S_Azimuth_62 : Outport  Port=237
  RadarSensor:0.OBJ_S_Azimuth_63 : Outport  Port=238
  RadarSensor:0.OBJ_S_Azimuth_64 : Outport  Port=239
  RadarSensor:0.OBJ_S_Elevation : Outport  Port=240
  RadarSensor:0.OBJ_S_Elevation_1 : Outport  Port=241
  RadarSensor:0.OBJ_S_Elevation_2 : Outport  Port=242
  RadarSensor:0.OBJ_S_Elevation_3 : Outport  Port=243
  RadarSensor:0.OBJ_S_Elevation_4 : Outport  Port=244
  RadarSensor:0.OBJ_S_Elevation_5 : Outport  Port=245
  RadarSensor:0.OBJ_S_Elevation_6 : Outport  Port=246
  RadarSensor:0.OBJ_S_Elevation_7 : Outport  Port=247
  RadarSensor:0.OBJ_S_Elevation_8 : Outport  Port=248
  RadarSensor:0.OBJ_S_Elevation_9 : Outport  Port=249
  RadarSensor:0.OBJ_S_Elevation_10 : Outport  Port=250
  RadarSensor:0.OBJ_S_Elevation_11 : Outport  Port=251
  RadarSensor:0.OBJ_S_Elevation_12 : Outport  Port=252
  RadarSensor:0.OBJ_S_Elevation_13 : Outport  Port=253
  RadarSensor:0.OBJ_S_Elevation_14 : Outport  Port=254
  RadarSensor:0.OBJ_S_Elevation_15 : Outport  Port=255
  RadarSensor:0.OBJ_S_Elevation_16 : Outport  Port=256
  RadarSensor:0.OBJ_S_Elevation_17 : Outport  Port=257
  RadarSensor:0.OBJ_S_Elevation_18 : Outport  Port=258
  RadarSensor:0.OBJ_S_Elevation_19 : Outport  Port=259
  RadarSensor:0.OBJ_S_Elevation_20 : Outport  Port=260
  RadarSensor:0.OBJ_S_Elevation_21 : Outport  Port=261
  RadarSensor:0.OBJ_S_Elevation_22 : Outport  Port=262
  RadarSensor:0.OBJ_S_Elevation_23 : Outport  Port=263
  RadarSensor:0.OBJ_S_Elevation_24 : Outport  Port=264
  RadarSensor:0.OBJ_S_Elevation_25 : Outport  Port=265
  RadarSensor:0.OBJ_S_Elevation_26 : Outport  Port=266
  RadarSensor:0.OBJ_S_Elevation_27 : Outport  Port=267
  RadarSensor:0.OBJ_S_Elevation_28 : Outport  Port=268
  RadarSensor:0.OBJ_S_Elevation_29 : Outport  Port=269
  RadarSensor:0.OBJ_S_Elevation_30 : Outport  Port=270
  RadarSensor:0.OBJ_S_Elevation_31 : Outport  Port=271
  RadarSensor:0.OBJ_S_Elevation_32 : Outport  Port=272
  RadarSensor:0.OBJ_S_Elevation_33 : Outport  Port=273
  RadarSensor:0.OBJ_S_Elevation_34 : Outport  Port=274
  RadarSensor:0.OBJ_S_Elevation_35 : Outport  Port=275
  RadarSensor:0.OBJ_S_Elevation_36 : Outport  Port=276
  RadarSensor:0.OBJ_S_Elevation_37 : Outport  Port=277
  RadarSensor:0.OBJ_S_Elevation_38 : Outport  Port=278
  RadarSensor:0.OBJ_S_Elevation_39 : Outport  Port=279
  RadarSensor:0.OBJ_S_Elevation_40 : Outport  Port=280
  RadarSensor:0.OBJ_S_Elevation_41 : Outport  Port=281
  RadarSensor:0.OBJ_S_Elevation_42 : Outport  Port=282
  RadarSensor:0.OBJ_S_Elevation_43 : Outport  Port=283
  RadarSensor:0.OBJ_S_Elevation_44 : Outport  Port=284
  RadarSensor:0.OBJ_S_Elevation_45 : Outport  Port=285
  RadarSensor:0.OBJ_S_Elevation_46 : Outport  Port=286
  RadarSensor:0.OBJ_S_Elevation_47 : Outport  Port=287
  RadarSensor:0.OBJ_S_Elevation_48 : Outport  Port=288
  RadarSensor:0.OBJ_S_Elevation_49 : Outport  Port=289
  RadarSensor:0.OBJ_S_Elevation_50 : Outport  Port=290
  RadarSensor:0.OBJ_S_Elevation_51 : Outport  Port=291
  RadarSensor:0.OBJ_S_Elevation_52 : Outport  Port=292
  RadarSensor:0.OBJ_S_Elevation_53 : Outport  Port=293
  RadarSensor:0.OBJ_S_Elevation_54 : Outport  Port=294
  RadarSensor:0.OBJ_S_Elevation_55 : Outport  Port=295
  RadarSensor:0.OBJ_S_Elevation_56 : Outport  Port=296
  RadarSensor:0.OBJ_S_Elevation_57 : Outport  Port=297
  RadarSensor:0.OBJ_S_Elevation_58 : Outport  Port=298
  RadarSensor:0.OBJ_S_Elevation_59 : Outport  Port=299
  RadarSensor:0.OBJ_S_Elevation_60 : Outport  Port=300
  RadarSensor:0.OBJ_S_Elevation_61 : Outport  Port=301
  RadarSensor:0.OBJ_S_Elevation_62 : Outport  Port=302
  RadarSensor:0.OBJ_S_Elevation_63 : Outport  Port=303
  RadarSensor:0.OBJ_S_Elevation_64 : Outport  Port=304
  RadarSensor:0.OBJ_S_Velocity : Outport  Port=305
  RadarSensor:0.OBJ_S_Velocity_1 : Outport  Port=306
  RadarSensor:0.OBJ_S_Velocity_2 : Outport  Port=307
  RadarSensor:0.OBJ_S_Velocity_3 : Outport  Port=308
  RadarSensor:0.OBJ_S_Velocity_4 : Outport  Port=309
  RadarSensor:0.OBJ_S_Velocity_5 : Outport  Port=310
  RadarSensor:0.OBJ_S_Velocity_6 : Outport  Port=311
  RadarSensor:0.OBJ_S_Velocity_7 : Outport  Port=312
  RadarSensor:0.OBJ_S_Velocity_8 : Outport  Port=313
  RadarSensor:0.OBJ_S_Velocity_9 : Outport  Port=314
  RadarSensor:0.OBJ_S_Velocity_10 : Outport  Port=315
  RadarSensor:0.OBJ_S_Velocity_11 : Outport  Port=316
  RadarSensor:0.OBJ_S_Velocity_12 : Outport  Port=317
  RadarSensor:0.OBJ_S_Velocity_13 : Outport  Port=318
  RadarSensor:0.OBJ_S_Velocity_14 : Outport  Port=319
  RadarSensor:0.OBJ_S_Velocity_15 : Outport  Port=320
  RadarSensor:0.OBJ_S_Velocity_16 : Outport  Port=321
  RadarSensor:0.OBJ_S_Velocity_17 : Outport  Port=322
  RadarSensor:0.OBJ_S_Velocity_18 : Outport  Port=323
  RadarSensor:0.OBJ_S_Velocity_19 : Outport  Port=324
  RadarSensor:0.OBJ_S_Velocity_20 : Outport  Port=325
  RadarSensor:0.OBJ_S_Velocity_21 : Outport  Port=326
  RadarSensor:0.OBJ_S_Velocity_22 : Outport  Port=327
  RadarSensor:0.OBJ_S_Velocity_23 : Outport  Port=328
  RadarSensor:0.OBJ_S_Velocity_24 : Outport  Port=329
  RadarSensor:0.OBJ_S_Velocity_25 : Outport  Port=330
  RadarSensor:0.OBJ_S_Velocity_26 : Outport  Port=331
  RadarSensor:0.OBJ_S_Velocity_27 : Outport  Port=332
  RadarSensor:0.OBJ_S_Velocity_28 : Outport  Port=333
  RadarSensor:0.OBJ_S_Velocity_29 : Outport  Port=334
  RadarSensor:0.OBJ_S_Velocity_30 : Outport  Port=335
  RadarSensor:0.OBJ_S_Velocity_31 : Outport  Port=336
  RadarSensor:0.OBJ_S_Velocity_32 : Outport  Port=337
  RadarSensor:0.OBJ_S_Velocity_33 : Outport  Port=338
  RadarSensor:0.OBJ_S_Velocity_34 : Outport  Port=339
  RadarSensor:0.OBJ_S_Velocity_35 : Outport  Port=340
  RadarSensor:0.OBJ_S_Velocity_36 : Outport  Port=341
  RadarSensor:0.OBJ_S_Velocity_37 : Outport  Port=342
  RadarSensor:0.OBJ_S_Velocity_38 : Outport  Port=343
  RadarSensor:0.OBJ_S_Velocity_39 : Outport  Port=344
  RadarSensor:0.OBJ_S_Velocity_40 : Outport  Port=345
  RadarSensor:0.OBJ_S_Velocity_41 : Outport  Port=346
  RadarSensor:0.OBJ_S_Velocity_42 : Outport  Port=347
  RadarSensor:0.OBJ_S_Velocity_43 : Outport  Port=348
  RadarSensor:0.OBJ_S_Velocity_44 : Outport  Port=349
  RadarSensor:0.OBJ_S_Velocity_45 : Outport  Port=350
  RadarSensor:0.OBJ_S_Velocity_46 : Outport  Port=351
  RadarSensor:0.OBJ_S_Velocity_47 : Outport  Port=352
  RadarSensor:0.OBJ_S_Velocity_48 : Outport  Port=353
  RadarSensor:0.OBJ_S_Velocity_49 : Outport  Port=354
  RadarSensor:0.OBJ_S_Velocity_50 : Outport  Port=355
  RadarSensor:0.OBJ_S_Velocity_51 : Outport  Port=356
  RadarSensor:0.OBJ_S_Velocity_52 : Outport  Port=357
  RadarSensor:0.OBJ_S_Velocity_53 : Outport  Port=358
  RadarSensor:0.OBJ_S_Velocity_54 : Outport  Port=359
  RadarSensor:0.OBJ_S_Velocity_55 : Outport  Port=360
  RadarSensor:0.OBJ_S_Velocity_56 : Outport  Port=361
  RadarSensor:0.OBJ_S_Velocity_57 : Outport  Port=362
  RadarSensor:0.OBJ_S_Velocity_58 : Outport  Port=363
  RadarSensor:0.OBJ_S_Velocity_59 : Outport  Port=364
  RadarSensor:0.OBJ_S_Velocity_60 : Outport  Port=365
  RadarSensor:0.OBJ_S_Velocity_61 : Outport  Port=366
  RadarSensor:0.OBJ_S_Velocity_62 : Outport  Port=367
  RadarSensor:0.OBJ_S_Velocity_63 : Outport  Port=368
  RadarSensor:0.OBJ_S_Velocity_64 : Outport  Port=369
  RadarSensor:0.OBJ_S_Range : Outport  Port=370
  RadarSensor:0.OBJ_S_Range_1 : Outport  Port=371
  RadarSensor:0.OBJ_S_Range_2 : Outport  Port=372
  RadarSensor:0.OBJ_S_Range_3 : Outport  Port=373
  RadarSensor:0.OBJ_S_Range_4 : Outport  Port=374
  RadarSensor:0.OBJ_S_Range_5 : Outport  Port=375
  RadarSensor:0.OBJ_S_Range_6 : Outport  Port=376
  RadarSensor:0.OBJ_S_Range_7 : Outport  Port=377
  RadarSensor:0.OBJ_S_Range_8 : Outport  Port=378
  RadarSensor:0.OBJ_S_Range_9 : Outport  Port=379
  RadarSensor:0.OBJ_S_Range_10 : Outport  Port=380
  RadarSensor:0.OBJ_S_Range_11 : Outport  Port=381
  RadarSensor:0.OBJ_S_Range_12 : Outport  Port=382
  RadarSensor:0.OBJ_S_Range_13 : Outport  Port=383
  RadarSensor:0.OBJ_S_Range_14 : Outport  Port=384
  RadarSensor:0.OBJ_S_Range_15 : Outport  Port=385
  RadarSensor:0.OBJ_S_Range_16 : Outport  Port=386
  RadarSensor:0.OBJ_S_Range_17 : Outport  Port=387
  RadarSensor:0.OBJ_S_Range_18 : Outport  Port=388
  RadarSensor:0.OBJ_S_Range_19 : Outport  Port=389
  RadarSensor:0.OBJ_S_Range_20 : Outport  Port=390
  RadarSensor:0.OBJ_S_Range_21 : Outport  Port=391
  RadarSensor:0.OBJ_S_Range_22 : Outport  Port=392
  RadarSensor:0.OBJ_S_Range_23 : Outport  Port=393
  RadarSensor:0.OBJ_S_Range_24 : Outport  Port=394
  RadarSensor:0.OBJ_S_Range_25 : Outport  Port=395
  RadarSensor:0.OBJ_S_Range_26 : Outport  Port=396
  RadarSensor:0.OBJ_S_Range_27 : Outport  Port=397
  RadarSensor:0.OBJ_S_Range_28 : Outport  Port=398
  RadarSensor:0.OBJ_S_Range_29 : Outport  Port=399
  RadarSensor:0.OBJ_S_Range_30 : Outport  Port=400
  RadarSensor:0.OBJ_S_Range_31 : Outport  Port=401
  RadarSensor:0.OBJ_S_Range_32 : Outport  Port=402
  RadarSensor:0.OBJ_S_Range_33 : Outport  Port=403
  RadarSensor:0.OBJ_S_Range_34 : Outport  Port=404
  RadarSensor:0.OBJ_S_Range_35 : Outport  Port=405
  RadarSensor:0.OBJ_S_Range_36 : Outport  Port=406
  RadarSensor:0.OBJ_S_Range_37 : Outport  Port=407
  RadarSensor:0.OBJ_S_Range_38 : Outport  Port=408
  RadarSensor:0.OBJ_S_Range_39 : Outport  Port=409
  RadarSensor:0.OBJ_S_Range_40 : Outport  Port=410
  RadarSensor:0.OBJ_S_Range_41 : Outport  Port=411
  RadarSensor:0.OBJ_S_Range_42 : Outport  Port=412
  RadarSensor:0.OBJ_S_Range_43 : Outport  Port=413
  RadarSensor:0.OBJ_S_Range_44 : Outport  Port=414
  RadarSensor:0.OBJ_S_Range_45 : Outport  Port=415
  RadarSensor:0.OBJ_S_Range_46 : Outport  Port=416
  RadarSensor:0.OBJ_S_Range_47 : Outport  Port=417
  RadarSensor:0.OBJ_S_Range_48 : Outport  Port=418
  RadarSensor:0.OBJ_S_Range_49 : Outport  Port=419
  RadarSensor:0.OBJ_S_Range_50 : Outport  Port=420
  RadarSensor:0.OBJ_S_Range_51 : Outport  Port=421
  RadarSensor:0.OBJ_S_Range_52 : Outport  Port=422
  RadarSensor:0.OBJ_S_Range_53 : Outport  Port=423
  RadarSensor:0.OBJ_S_Range_54 : Outport  Port=424
  RadarSensor:0.OBJ_S_Range_55 : Outport  Port=425
  RadarSensor:0.OBJ_S_Range_56 : Outport  Port=426
  RadarSensor:0.OBJ_S_Range_57 : Outport  Port=427
  RadarSensor:0.OBJ_S_Range_58 : Outport  Port=428
  RadarSensor:0.OBJ_S_Range_59 : Outport  Port=429
  RadarSensor:0.OBJ_S_Range_60 : Outport  Port=430
  RadarSensor:0.OBJ_S_Range_61 : Outport  Port=431
  RadarSensor:0.OBJ_S_Range_62 : Outport  Port=432
  RadarSensor:0.OBJ_S_Range_63 : Outport  Port=433
  RadarSensor:0.OBJ_S_Range_64 : Outport  Port=434
  RadarSensor:0.OBJ_RCS : Outport  Port=435
  RadarSensor:0.OBJ_RCS_1 : Outport  Port=436
  RadarSensor:0.OBJ_RCS_2 : Outport  Port=437
  RadarSensor:0.OBJ_RCS_3 : Outport  Port=438
  RadarSensor:0.OBJ_RCS_4 : Outport  Port=439
  RadarSensor:0.OBJ_RCS_5 : Outport  Port=440
  RadarSensor:0.OBJ_RCS_6 : Outport  Port=441
  RadarSensor:0.OBJ_RCS_7 : Outport  Port=442
  RadarSensor:0.OBJ_RCS_8 : Outport  Port=443
  RadarSensor:0.OBJ_RCS_9 : Outport  Port=444
  RadarSensor:0.OBJ_RCS_10 : Outport  Port=445
  RadarSensor:0.OBJ_RCS_11 : Outport  Port=446
  RadarSensor:0.OBJ_RCS_12 : Outport  Port=447
  RadarSensor:0.OBJ_RCS_13 : Outport  Port=448
  RadarSensor:0.OBJ_RCS_14 : Outport  Port=449
  RadarSensor:0.OBJ_RCS_15 : Outport  Port=450
  RadarSensor:0.OBJ_RCS_16 : Outport  Port=451
  RadarSensor:0.OBJ_RCS_17 : Outport  Port=452
  RadarSensor:0.OBJ_RCS_18 : Outport  Port=453
  RadarSensor:0.OBJ_RCS_19 : Outport  Port=454
  RadarSensor:0.OBJ_RCS_20 : Outport  Port=455
  RadarSensor:0.OBJ_RCS_21 : Outport  Port=456
  RadarSensor:0.OBJ_RCS_22 : Outport  Port=457
  RadarSensor:0.OBJ_RCS_23 : Outport  Port=458
  RadarSensor:0.OBJ_RCS_24 : Outport  Port=459
  RadarSensor:0.OBJ_RCS_25 : Outport  Port=460
  RadarSensor:0.OBJ_RCS_26 : Outport  Port=461
  RadarSensor:0.OBJ_RCS_27 : Outport  Port=462
  RadarSensor:0.OBJ_RCS_28 : Outport  Port=463
  RadarSensor:0.OBJ_RCS_29 : Outport  Port=464
  RadarSensor:0.OBJ_RCS_30 : Outport  Port=465
  RadarSensor:0.OBJ_RCS_31 : Outport  Port=466
  RadarSensor:0.OBJ_RCS_32 : Outport  Port=467
  RadarSensor:0.OBJ_RCS_33 : Outport  Port=468
  RadarSensor:0.OBJ_RCS_34 : Outport  Port=469
  RadarSensor:0.OBJ_RCS_35 : Outport  Port=470
  RadarSensor:0.OBJ_RCS_36 : Outport  Port=471
  RadarSensor:0.OBJ_RCS_37 : Outport  Port=472
  RadarSensor:0.OBJ_RCS_38 : Outport  Port=473
  RadarSensor:0.OBJ_RCS_39 : Outport  Port=474
  RadarSensor:0.OBJ_RCS_40 : Outport  Port=475
  RadarSensor:0.OBJ_RCS_41 : Outport  Port=476
  RadarSensor:0.OBJ_RCS_42 : Outport  Port=477
  RadarSensor:0.OBJ_RCS_43 : Outport  Port=478
  RadarSensor:0.OBJ_RCS_44 : Outport  Port=479
  RadarSensor:0.OBJ_RCS_45 : Outport  Port=480
  RadarSensor:0.OBJ_RCS_46 : Outport  Port=481
  RadarSensor:0.OBJ_RCS_47 : Outport  Port=482
  RadarSensor:0.OBJ_RCS_48 : Outport  Port=483
  RadarSensor:0.OBJ_RCS_49 : Outport  Port=484
  RadarSensor:0.OBJ_RCS_50 : Outport  Port=485
  RadarSensor:0.OBJ_RCS_51 : Outport  Port=486
  RadarSensor:0.OBJ_RCS_52 : Outport  Port=487
  RadarSensor:0.OBJ_RCS_53 : Outport  Port=488
  RadarSensor:0.OBJ_RCS_54 : Outport  Port=489
  RadarSensor:0.OBJ_RCS_55 : Outport  Port=490
  RadarSensor:0.OBJ_RCS_56 : Outport  Port=491
  RadarSensor:0.OBJ_RCS_57 : Outport  Port=492
  RadarSensor:0.OBJ_RCS_58 : Outport  Port=493
  RadarSensor:0.OBJ_RCS_59 : Outport  Port=494
  RadarSensor:0.OBJ_RCS_60 : Outport  Port=495
  RadarSensor:0.OBJ_RCS_61 : Outport  Port=496
  RadarSensor:0.OBJ_RCS_62 : Outport  Port=497
  RadarSensor:0.OBJ_RCS_63 : Outport  Port=498
  RadarSensor:0.OBJ_RCS_64 : Outport  Port=499
  RadarSensor:1.time : Outport  Port=500
  RadarSensor:1.width : Outport  Port=501
  RadarSensor:1.OBJ_ID : Outport  Port=502
  RadarSensor:1.OBJ_ID_1 : Outport  Port=503
  RadarSensor:1.OBJ_ID_2 : Outport  Port=504
  RadarSensor:1.OBJ_ID_3 : Outport  Port=505
  RadarSensor:1.OBJ_ID_4 : Outport  Port=506
  RadarSensor:1.OBJ_ID_5 : Outport  Port=507
  RadarSensor:1.OBJ_ID_6 : Outport  Port=508
  RadarSensor:1.OBJ_ID_7 : Outport  Port=509
  RadarSensor:1.OBJ_ID_8 : Outport  Port=510
  RadarSensor:1.OBJ_ID_9 : Outport  Port=511
  RadarSensor:1.OBJ_ID_10 : Outport  Port=512
  RadarSensor:1.OBJ_ID_11 : Outport  Port=513
  RadarSensor:1.OBJ_ID_12 : Outport  Port=514
  RadarSensor:1.OBJ_ID_13 : Outport  Port=515
  RadarSensor:1.OBJ_ID_14 : Outport  Port=516
  RadarSensor:1.OBJ_ID_15 : Outport  Port=517
  RadarSensor:1.OBJ_ID_16 : Outport  Port=518
  RadarSensor:1.OBJ_ID_17 : Outport  Port=519
  RadarSensor:1.OBJ_ID_18 : Outport  Port=520
  RadarSensor:1.OBJ_ID_19 : Outport  Port=521
  RadarSensor:1.OBJ_ID_20 : Outport  Port=522
  RadarSensor:1.OBJ_ID_21 : Outport  Port=523
  RadarSensor:1.OBJ_ID_22 : Outport  Port=524
  RadarSensor:1.OBJ_ID_23 : Outport  Port=525
  RadarSensor:1.OBJ_ID_24 : Outport  Port=526
  RadarSensor:1.OBJ_ID_25 : Outport  Port=527
  RadarSensor:1.OBJ_ID_26 : Outport  Port=528
  RadarSensor:1.OBJ_ID_27 : Outport  Port=529
  RadarSensor:1.OBJ_ID_28 : Outport  Port=530
  RadarSensor:1.OBJ_ID_29 : Outport  Port=531
  RadarSensor:1.OBJ_ID_30 : Outport  Port=532
  RadarSensor:1.OBJ_ID_31 : Outport  Port=533
  RadarSensor:1.OBJ_ID_32 : Outport  Port=534
  RadarSensor:1.OBJ_ID_33 : Outport  Port=535
  RadarSensor:1.OBJ_ID_34 : Outport  Port=536
  RadarSensor:1.OBJ_ID_35 : Outport  Port=537
  RadarSensor:1.OBJ_ID_36 : Outport  Port=538
  RadarSensor:1.OBJ_ID_37 : Outport  Port=539
  RadarSensor:1.OBJ_ID_38 : Outport  Port=540
  RadarSensor:1.OBJ_ID_39 : Outport  Port=541
  RadarSensor:1.OBJ_ID_40 : Outport  Port=542
  RadarSensor:1.OBJ_ID_41 : Outport  Port=543
  RadarSensor:1.OBJ_ID_42 : Outport  Port=544
  RadarSensor:1.OBJ_ID_43 : Outport  Port=545
  RadarSensor:1.OBJ_ID_44 : Outport  Port=546
  RadarSensor:1.OBJ_ID_45 : Outport  Port=547
  RadarSensor:1.OBJ_ID_46 : Outport  Port=548
  RadarSensor:1.OBJ_ID_47 : Outport  Port=549
  RadarSensor:1.OBJ_ID_48 : Outport  Port=550
  RadarSensor:1.OBJ_ID_49 : Outport  Port=551
  RadarSensor:1.OBJ_ID_50 : Outport  Port=552
  RadarSensor:1.OBJ_ID_51 : Outport  Port=553
  RadarSensor:1.OBJ_ID_52 : Outport  Port=554
  RadarSensor:1.OBJ_ID_53 : Outport  Port=555
  RadarSensor:1.OBJ_ID_54 : Outport  Port=556
  RadarSensor:1.OBJ_ID_55 : Outport  Port=557
  RadarSensor:1.OBJ_ID_56 : Outport  Port=558
  RadarSensor:1.OBJ_ID_57 : Outport  Port=559
  RadarSensor:1.OBJ_ID_58 : Outport  Port=560
  RadarSensor:1.OBJ_ID_59 : Outport  Port=561
  RadarSensor:1.OBJ_ID_60 : Outport  Port=562
  RadarSensor:1.OBJ_ID_61 : Outport  Port=563
  RadarSensor:1.OBJ_ID_62 : Outport  Port=564
  RadarSensor:1.OBJ_ID_63 : Outport  Port=565
  RadarSensor:1.OBJ_ID_64 : Outport  Port=566
  RadarSensor:1.OBJ_Class : Outport  Port=567
  RadarSensor:1.OBJ_Class_1 : Outport  Port=568
  RadarSensor:1.OBJ_Class_2 : Outport  Port=569
  RadarSensor:1.OBJ_Class_3 : Outport  Port=570
  RadarSensor:1.OBJ_Class_4 : Outport  Port=571
  RadarSensor:1.OBJ_Class_5 : Outport  Port=572
  RadarSensor:1.OBJ_Class_6 : Outport  Port=573
  RadarSensor:1.OBJ_Class_7 : Outport  Port=574
  RadarSensor:1.OBJ_Class_8 : Outport  Port=575
  RadarSensor:1.OBJ_Class_9 : Outport  Port=576
  RadarSensor:1.OBJ_Class_10 : Outport  Port=577
  RadarSensor:1.OBJ_Class_11 : Outport  Port=578
  RadarSensor:1.OBJ_Class_12 : Outport  Port=579
  RadarSensor:1.OBJ_Class_13 : Outport  Port=580
  RadarSensor:1.OBJ_Class_14 : Outport  Port=581
  RadarSensor:1.OBJ_Class_15 : Outport  Port=582
  RadarSensor:1.OBJ_Class_16 : Outport  Port=583
  RadarSensor:1.OBJ_Class_17 : Outport  Port=584
  RadarSensor:1.OBJ_Class_18 : Outport  Port=585
  RadarSensor:1.OBJ_Class_19 : Outport  Port=586
  RadarSensor:1.OBJ_Class_20 : Outport  Port=587
  RadarSensor:1.OBJ_Class_21 : Outport  Port=588
  RadarSensor:1.OBJ_Class_22 : Outport  Port=589
  RadarSensor:1.OBJ_Class_23 : Outport  Port=590
  RadarSensor:1.OBJ_Class_24 : Outport  Port=591
  RadarSensor:1.OBJ_Class_25 : Outport  Port=592
  RadarSensor:1.OBJ_Class_26 : Outport  Port=593
  RadarSensor:1.OBJ_Class_27 : Outport  Port=594
  RadarSensor:1.OBJ_Class_28 : Outport  Port=595
  RadarSensor:1.OBJ_Class_29 : Outport  Port=596
  RadarSensor:1.OBJ_Class_30 : Outport  Port=597
  RadarSensor:1.OBJ_Class_31 : Outport  Port=598
  RadarSensor:1.OBJ_Class_32 : Outport  Port=599
  RadarSensor:1.OBJ_Class_33 : Outport  Port=600
  RadarSensor:1.OBJ_Class_34 : Outport  Port=601
  RadarSensor:1.OBJ_Class_35 : Outport  Port=602
  RadarSensor:1.OBJ_Class_36 : Outport  Port=603
  RadarSensor:1.OBJ_Class_37 : Outport  Port=604
  RadarSensor:1.OBJ_Class_38 : Outport  Port=605
  RadarSensor:1.OBJ_Class_39 : Outport  Port=606
  RadarSensor:1.OBJ_Class_40 : Outport  Port=607
  RadarSensor:1.OBJ_Class_41 : Outport  Port=608
  RadarSensor:1.OBJ_Class_42 : Outport  Port=609
  RadarSensor:1.OBJ_Class_43 : Outport  Port=610
  RadarSensor:1.OBJ_Class_44 : Outport  Port=611
  RadarSensor:1.OBJ_Class_45 : Outport  Port=612
  RadarSensor:1.OBJ_Class_46 : Outport  Port=613
  RadarSensor:1.OBJ_Class_47 : Outport  Port=614
  RadarSensor:1.OBJ_Class_48 : Outport  Port=615
  RadarSensor:1.OBJ_Class_49 : Outport  Port=616
  RadarSensor:1.OBJ_Class_50 : Outport  Port=617
  RadarSensor:1.OBJ_Class_51 : Outport  Port=618
  RadarSensor:1.OBJ_Class_52 : Outport  Port=619
  RadarSensor:1.OBJ_Class_53 : Outport  Port=620
  RadarSensor:1.OBJ_Class_54 : Outport  Port=621
  RadarSensor:1.OBJ_Class_55 : Outport  Port=622
  RadarSensor:1.OBJ_Class_56 : Outport  Port=623
  RadarSensor:1.OBJ_Class_57 : Outport  Port=624
  RadarSensor:1.OBJ_Class_58 : Outport  Port=625
  RadarSensor:1.OBJ_Class_59 : Outport  Port=626
  RadarSensor:1.OBJ_Class_60 : Outport  Port=627
  RadarSensor:1.OBJ_Class_61 : Outport  Port=628
  RadarSensor:1.OBJ_Class_62 : Outport  Port=629
  RadarSensor:1.OBJ_Class_63 : Outport  Port=630
  RadarSensor:1.OBJ_Class_64 : Outport  Port=631
  RadarSensor:1.OBJ_S_Azimuth : Outport  Port=632
  RadarSensor:1.OBJ_S_Azimuth_1 : Outport  Port=633
  RadarSensor:1.OBJ_S_Azimuth_2 : Outport  Port=634
  RadarSensor:1.OBJ_S_Azimuth_3 : Outport  Port=635
  RadarSensor:1.OBJ_S_Azimuth_4 : Outport  Port=636
  RadarSensor:1.OBJ_S_Azimuth_5 : Outport  Port=637
  RadarSensor:1.OBJ_S_Azimuth_6 : Outport  Port=638
  RadarSensor:1.OBJ_S_Azimuth_7 : Outport  Port=639
  RadarSensor:1.OBJ_S_Azimuth_8 : Outport  Port=640
  RadarSensor:1.OBJ_S_Azimuth_9 : Outport  Port=641
  RadarSensor:1.OBJ_S_Azimuth_10 : Outport  Port=642
  RadarSensor:1.OBJ_S_Azimuth_11 : Outport  Port=643
  RadarSensor:1.OBJ_S_Azimuth_12 : Outport  Port=644
  RadarSensor:1.OBJ_S_Azimuth_13 : Outport  Port=645
  RadarSensor:1.OBJ_S_Azimuth_14 : Outport  Port=646
  RadarSensor:1.OBJ_S_Azimuth_15 : Outport  Port=647
  RadarSensor:1.OBJ_S_Azimuth_16 : Outport  Port=648
  RadarSensor:1.OBJ_S_Azimuth_17 : Outport  Port=649
  RadarSensor:1.OBJ_S_Azimuth_18 : Outport  Port=650
  RadarSensor:1.OBJ_S_Azimuth_19 : Outport  Port=651
  RadarSensor:1.OBJ_S_Azimuth_20 : Outport  Port=652
  RadarSensor:1.OBJ_S_Azimuth_21 : Outport  Port=653
  RadarSensor:1.OBJ_S_Azimuth_22 : Outport  Port=654
  RadarSensor:1.OBJ_S_Azimuth_23 : Outport  Port=655
  RadarSensor:1.OBJ_S_Azimuth_24 : Outport  Port=656
  RadarSensor:1.OBJ_S_Azimuth_25 : Outport  Port=657
  RadarSensor:1.OBJ_S_Azimuth_26 : Outport  Port=658
  RadarSensor:1.OBJ_S_Azimuth_27 : Outport  Port=659
  RadarSensor:1.OBJ_S_Azimuth_28 : Outport  Port=660
  RadarSensor:1.OBJ_S_Azimuth_29 : Outport  Port=661
  RadarSensor:1.OBJ_S_Azimuth_30 : Outport  Port=662
  RadarSensor:1.OBJ_S_Azimuth_31 : Outport  Port=663
  RadarSensor:1.OBJ_S_Azimuth_32 : Outport  Port=664
  RadarSensor:1.OBJ_S_Azimuth_33 : Outport  Port=665
  RadarSensor:1.OBJ_S_Azimuth_34 : Outport  Port=666
  RadarSensor:1.OBJ_S_Azimuth_35 : Outport  Port=667
  RadarSensor:1.OBJ_S_Azimuth_36 : Outport  Port=668
  RadarSensor:1.OBJ_S_Azimuth_37 : Outport  Port=669
  RadarSensor:1.OBJ_S_Azimuth_38 : Outport  Port=670
  RadarSensor:1.OBJ_S_Azimuth_39 : Outport  Port=671
  RadarSensor:1.OBJ_S_Azimuth_40 : Outport  Port=672
  RadarSensor:1.OBJ_S_Azimuth_41 : Outport  Port=673
  RadarSensor:1.OBJ_S_Azimuth_42 : Outport  Port=674
  RadarSensor:1.OBJ_S_Azimuth_43 : Outport  Port=675
  RadarSensor:1.OBJ_S_Azimuth_44 : Outport  Port=676
  RadarSensor:1.OBJ_S_Azimuth_45 : Outport  Port=677
  RadarSensor:1.OBJ_S_Azimuth_46 : Outport  Port=678
  RadarSensor:1.OBJ_S_Azimuth_47 : Outport  Port=679
  RadarSensor:1.OBJ_S_Azimuth_48 : Outport  Port=680
  RadarSensor:1.OBJ_S_Azimuth_49 : Outport  Port=681
  RadarSensor:1.OBJ_S_Azimuth_50 : Outport  Port=682
  RadarSensor:1.OBJ_S_Azimuth_51 : Outport  Port=683
  RadarSensor:1.OBJ_S_Azimuth_52 : Outport  Port=684
  RadarSensor:1.OBJ_S_Azimuth_53 : Outport  Port=685
  RadarSensor:1.OBJ_S_Azimuth_54 : Outport  Port=686
  RadarSensor:1.OBJ_S_Azimuth_55 : Outport  Port=687
  RadarSensor:1.OBJ_S_Azimuth_56 : Outport  Port=688
  RadarSensor:1.OBJ_S_Azimuth_57 : Outport  Port=689
  RadarSensor:1.OBJ_S_Azimuth_58 : Outport  Port=690
  RadarSensor:1.OBJ_S_Azimuth_59 : Outport  Port=691
  RadarSensor:1.OBJ_S_Azimuth_60 : Outport  Port=692
  RadarSensor:1.OBJ_S_Azimuth_61 : Outport  Port=693
  RadarSensor:1.OBJ_S_Azimuth_62 : Outport  Port=694
  RadarSensor:1.OBJ_S_Azimuth_63 : Outport  Port=695
  RadarSensor:1.OBJ_S_Azimuth_64 : Outport  Port=696
  RadarSensor:1.OBJ_S_Elevation : Outport  Port=697
  RadarSensor:1.OBJ_S_Elevation_1 : Outport  Port=698
  RadarSensor:1.OBJ_S_Elevation_2 : Outport  Port=699
  RadarSensor:1.OBJ_S_Elevation_3 : Outport  Port=700
  RadarSensor:1.OBJ_S_Elevation_4 : Outport  Port=701
  RadarSensor:1.OBJ_S_Elevation_5 : Outport  Port=702
  RadarSensor:1.OBJ_S_Elevation_6 : Outport  Port=703
  RadarSensor:1.OBJ_S_Elevation_7 : Outport  Port=704
  RadarSensor:1.OBJ_S_Elevation_8 : Outport  Port=705
  RadarSensor:1.OBJ_S_Elevation_9 : Outport  Port=706
  RadarSensor:1.OBJ_S_Elevation_10 : Outport  Port=707
  RadarSensor:1.OBJ_S_Elevation_11 : Outport  Port=708
  RadarSensor:1.OBJ_S_Elevation_12 : Outport  Port=709
  RadarSensor:1.OBJ_S_Elevation_13 : Outport  Port=710
  RadarSensor:1.OBJ_S_Elevation_14 : Outport  Port=711
  RadarSensor:1.OBJ_S_Elevation_15 : Outport  Port=712
  RadarSensor:1.OBJ_S_Elevation_16 : Outport  Port=713
  RadarSensor:1.OBJ_S_Elevation_17 : Outport  Port=714
  RadarSensor:1.OBJ_S_Elevation_18 : Outport  Port=715
  RadarSensor:1.OBJ_S_Elevation_19 : Outport  Port=716
  RadarSensor:1.OBJ_S_Elevation_20 : Outport  Port=717
  RadarSensor:1.OBJ_S_Elevation_21 : Outport  Port=718
  RadarSensor:1.OBJ_S_Elevation_22 : Outport  Port=719
  RadarSensor:1.OBJ_S_Elevation_23 : Outport  Port=720
  RadarSensor:1.OBJ_S_Elevation_24 : Outport  Port=721
  RadarSensor:1.OBJ_S_Elevation_25 : Outport  Port=722
  RadarSensor:1.OBJ_S_Elevation_26 : Outport  Port=723
  RadarSensor:1.OBJ_S_Elevation_27 : Outport  Port=724
  RadarSensor:1.OBJ_S_Elevation_28 : Outport  Port=725
  RadarSensor:1.OBJ_S_Elevation_29 : Outport  Port=726
  RadarSensor:1.OBJ_S_Elevation_30 : Outport  Port=727
  RadarSensor:1.OBJ_S_Elevation_31 : Outport  Port=728
  RadarSensor:1.OBJ_S_Elevation_32 : Outport  Port=729
  RadarSensor:1.OBJ_S_Elevation_33 : Outport  Port=730
  RadarSensor:1.OBJ_S_Elevation_34 : Outport  Port=731
  RadarSensor:1.OBJ_S_Elevation_35 : Outport  Port=732
  RadarSensor:1.OBJ_S_Elevation_36 : Outport  Port=733
  RadarSensor:1.OBJ_S_Elevation_37 : Outport  Port=734
  RadarSensor:1.OBJ_S_Elevation_38 : Outport  Port=735
  RadarSensor:1.OBJ_S_Elevation_39 : Outport  Port=736
  RadarSensor:1.OBJ_S_Elevation_40 : Outport  Port=737
  RadarSensor:1.OBJ_S_Elevation_41 : Outport  Port=738
  RadarSensor:1.OBJ_S_Elevation_42 : Outport  Port=739
  RadarSensor:1.OBJ_S_Elevation_43 : Outport  Port=740
  RadarSensor:1.OBJ_S_Elevation_44 : Outport  Port=741
  RadarSensor:1.OBJ_S_Elevation_45 : Outport  Port=742
  RadarSensor:1.OBJ_S_Elevation_46 : Outport  Port=743
  RadarSensor:1.OBJ_S_Elevation_47 : Outport  Port=744
  RadarSensor:1.OBJ_S_Elevation_48 : Outport  Port=745
  RadarSensor:1.OBJ_S_Elevation_49 : Outport  Port=746
  RadarSensor:1.OBJ_S_Elevation_50 : Outport  Port=747
  RadarSensor:1.OBJ_S_Elevation_51 : Outport  Port=748
  RadarSensor:1.OBJ_S_Elevation_52 : Outport  Port=749
  RadarSensor:1.OBJ_S_Elevation_53 : Outport  Port=750
  RadarSensor:1.OBJ_S_Elevation_54 : Outport  Port=751
  RadarSensor:1.OBJ_S_Elevation_55 : Outport  Port=752
  RadarSensor:1.OBJ_S_Elevation_56 : Outport  Port=753
  RadarSensor:1.OBJ_S_Elevation_57 : Outport  Port=754
  RadarSensor:1.OBJ_S_Elevation_58 : Outport  Port=755
  RadarSensor:1.OBJ_S_Elevation_59 : Outport  Port=756
  RadarSensor:1.OBJ_S_Elevation_60 : Outport  Port=757
  RadarSensor:1.OBJ_S_Elevation_61 : Outport  Port=758
  RadarSensor:1.OBJ_S_Elevation_62 : Outport  Port=759
  RadarSensor:1.OBJ_S_Elevation_63 : Outport  Port=760
  RadarSensor:1.OBJ_S_Elevation_64 : Outport  Port=761
  RadarSensor:1.OBJ_S_Velocity : Outport  Port=762
  RadarSensor:1.OBJ_S_Velocity_1 : Outport  Port=763
  RadarSensor:1.OBJ_S_Velocity_2 : Outport  Port=764
  RadarSensor:1.OBJ_S_Velocity_3 : Outport  Port=765
  RadarSensor:1.OBJ_S_Velocity_4 : Outport  Port=766
  RadarSensor:1.OBJ_S_Velocity_5 : Outport  Port=767
  RadarSensor:1.OBJ_S_Velocity_6 : Outport  Port=768
  RadarSensor:1.OBJ_S_Velocity_7 : Outport  Port=769
  RadarSensor:1.OBJ_S_Velocity_8 : Outport  Port=770
  RadarSensor:1.OBJ_S_Velocity_9 : Outport  Port=771
  RadarSensor:1.OBJ_S_Velocity_10 : Outport  Port=772
  RadarSensor:1.OBJ_S_Velocity_11 : Outport  Port=773
  RadarSensor:1.OBJ_S_Velocity_12 : Outport  Port=774
  RadarSensor:1.OBJ_S_Velocity_13 : Outport  Port=775
  RadarSensor:1.OBJ_S_Velocity_14 : Outport  Port=776
  RadarSensor:1.OBJ_S_Velocity_15 : Outport  Port=777
  RadarSensor:1.OBJ_S_Velocity_16 : Outport  Port=778
  RadarSensor:1.OBJ_S_Velocity_17 : Outport  Port=779
  RadarSensor:1.OBJ_S_Velocity_18 : Outport  Port=780
  RadarSensor:1.OBJ_S_Velocity_19 : Outport  Port=781
  RadarSensor:1.OBJ_S_Velocity_20 : Outport  Port=782
  RadarSensor:1.OBJ_S_Velocity_21 : Outport  Port=783
  RadarSensor:1.OBJ_S_Velocity_22 : Outport  Port=784
  RadarSensor:1.OBJ_S_Velocity_23 : Outport  Port=785
  RadarSensor:1.OBJ_S_Velocity_24 : Outport  Port=786
  RadarSensor:1.OBJ_S_Velocity_25 : Outport  Port=787
  RadarSensor:1.OBJ_S_Velocity_26 : Outport  Port=788
  RadarSensor:1.OBJ_S_Velocity_27 : Outport  Port=789
  RadarSensor:1.OBJ_S_Velocity_28 : Outport  Port=790
  RadarSensor:1.OBJ_S_Velocity_29 : Outport  Port=791
  RadarSensor:1.OBJ_S_Velocity_30 : Outport  Port=792
  RadarSensor:1.OBJ_S_Velocity_31 : Outport  Port=793
  RadarSensor:1.OBJ_S_Velocity_32 : Outport  Port=794
  RadarSensor:1.OBJ_S_Velocity_33 : Outport  Port=795
  RadarSensor:1.OBJ_S_Velocity_34 : Outport  Port=796
  RadarSensor:1.OBJ_S_Velocity_35 : Outport  Port=797
  RadarSensor:1.OBJ_S_Velocity_36 : Outport  Port=798
  RadarSensor:1.OBJ_S_Velocity_37 : Outport  Port=799
  RadarSensor:1.OBJ_S_Velocity_38 : Outport  Port=800
  RadarSensor:1.OBJ_S_Velocity_39 : Outport  Port=801
  RadarSensor:1.OBJ_S_Velocity_40 : Outport  Port=802
  RadarSensor:1.OBJ_S_Velocity_41 : Outport  Port=803
  RadarSensor:1.OBJ_S_Velocity_42 : Outport  Port=804
  RadarSensor:1.OBJ_S_Velocity_43 : Outport  Port=805
  RadarSensor:1.OBJ_S_Velocity_44 : Outport  Port=806
  RadarSensor:1.OBJ_S_Velocity_45 : Outport  Port=807
  RadarSensor:1.OBJ_S_Velocity_46 : Outport  Port=808
  RadarSensor:1.OBJ_S_Velocity_47 : Outport  Port=809
  RadarSensor:1.OBJ_S_Velocity_48 : Outport  Port=810
  RadarSensor:1.OBJ_S_Velocity_49 : Outport  Port=811
  RadarSensor:1.OBJ_S_Velocity_50 : Outport  Port=812
  RadarSensor:1.OBJ_S_Velocity_51 : Outport  Port=813
  RadarSensor:1.OBJ_S_Velocity_52 : Outport  Port=814
  RadarSensor:1.OBJ_S_Velocity_53 : Outport  Port=815
  RadarSensor:1.OBJ_S_Velocity_54 : Outport  Port=816
  RadarSensor:1.OBJ_S_Velocity_55 : Outport  Port=817
  RadarSensor:1.OBJ_S_Velocity_56 : Outport  Port=818
  RadarSensor:1.OBJ_S_Velocity_57 : Outport  Port=819
  RadarSensor:1.OBJ_S_Velocity_58 : Outport  Port=820
  RadarSensor:1.OBJ_S_Velocity_59 : Outport  Port=821
  RadarSensor:1.OBJ_S_Velocity_60 : Outport  Port=822
  RadarSensor:1.OBJ_S_Velocity_61 : Outport  Port=823
  RadarSensor:1.OBJ_S_Velocity_62 : Outport  Port=824
  RadarSensor:1.OBJ_S_Velocity_63 : Outport  Port=825
  RadarSensor:1.OBJ_S_Velocity_64 : Outport  Port=826
  RadarSensor:1.OBJ_S_Range : Outport  Port=827
  RadarSensor:1.OBJ_S_Range_1 : Outport  Port=828
  RadarSensor:1.OBJ_S_Range_2 : Outport  Port=829
  RadarSensor:1.OBJ_S_Range_3 : Outport  Port=830
  RadarSensor:1.OBJ_S_Range_4 : Outport  Port=831
  RadarSensor:1.OBJ_S_Range_5 : Outport  Port=832
  RadarSensor:1.OBJ_S_Range_6 : Outport  Port=833
  RadarSensor:1.OBJ_S_Range_7 : Outport  Port=834
  RadarSensor:1.OBJ_S_Range_8 : Outport  Port=835
  RadarSensor:1.OBJ_S_Range_9 : Outport  Port=836
  RadarSensor:1.OBJ_S_Range_10 : Outport  Port=837
  RadarSensor:1.OBJ_S_Range_11 : Outport  Port=838
  RadarSensor:1.OBJ_S_Range_12 : Outport  Port=839
  RadarSensor:1.OBJ_S_Range_13 : Outport  Port=840
  RadarSensor:1.OBJ_S_Range_14 : Outport  Port=841
  RadarSensor:1.OBJ_S_Range_15 : Outport  Port=842
  RadarSensor:1.OBJ_S_Range_16 : Outport  Port=843
  RadarSensor:1.OBJ_S_Range_17 : Outport  Port=844
  RadarSensor:1.OBJ_S_Range_18 : Outport  Port=845
  RadarSensor:1.OBJ_S_Range_19 : Outport  Port=846
  RadarSensor:1.OBJ_S_Range_20 : Outport  Port=847
  RadarSensor:1.OBJ_S_Range_21 : Outport  Port=848
  RadarSensor:1.OBJ_S_Range_22 : Outport  Port=849
  RadarSensor:1.OBJ_S_Range_23 : Outport  Port=850
  RadarSensor:1.OBJ_S_Range_24 : Outport  Port=851
  RadarSensor:1.OBJ_S_Range_25 : Outport  Port=852
  RadarSensor:1.OBJ_S_Range_26 : Outport  Port=853
  RadarSensor:1.OBJ_S_Range_27 : Outport  Port=854
  RadarSensor:1.OBJ_S_Range_28 : Outport  Port=855
  RadarSensor:1.OBJ_S_Range_29 : Outport  Port=856
  RadarSensor:1.OBJ_S_Range_30 : Outport  Port=857
  RadarSensor:1.OBJ_S_Range_31 : Outport  Port=858
  RadarSensor:1.OBJ_S_Range_32 : Outport  Port=859
  RadarSensor:1.OBJ_S_Range_33 : Outport  Port=860
  RadarSensor:1.OBJ_S_Range_34 : Outport  Port=861
  RadarSensor:1.OBJ_S_Range_35 : Outport  Port=862
  RadarSensor:1.OBJ_S_Range_36 : Outport  Port=863
  RadarSensor:1.OBJ_S_Range_37 : Outport  Port=864
  RadarSensor:1.OBJ_S_Range_38 : Outport  Port=865
  RadarSensor:1.OBJ_S_Range_39 : Outport  Port=866
  RadarSensor:1.OBJ_S_Range_40 : Outport  Port=867
  RadarSensor:1.OBJ_S_Range_41 : Outport  Port=868
  RadarSensor:1.OBJ_S_Range_42 : Outport  Port=869
  RadarSensor:1.OBJ_S_Range_43 : Outport  Port=870
  RadarSensor:1.OBJ_S_Range_44 : Outport  Port=871
  RadarSensor:1.OBJ_S_Range_45 : Outport  Port=872
  RadarSensor:1.OBJ_S_Range_46 : Outport  Port=873
  RadarSensor:1.OBJ_S_Range_47 : Outport  Port=874
  RadarSensor:1.OBJ_S_Range_48 : Outport  Port=875
  RadarSensor:1.OBJ_S_Range_49 : Outport  Port=876
  RadarSensor:1.OBJ_S_Range_50 : Outport  Port=877
  RadarSensor:1.OBJ_S_Range_51 : Outport  Port=878
  RadarSensor:1.OBJ_S_Range_52 : Outport  Port=879
  RadarSensor:1.OBJ_S_Range_53 : Outport  Port=880
  RadarSensor:1.OBJ_S_Range_54 : Outport  Port=881
  RadarSensor:1.OBJ_S_Range_55 : Outport  Port=882
  RadarSensor:1.OBJ_S_Range_56 : Outport  Port=883
  RadarSensor:1.OBJ_S_Range_57 : Outport  Port=884
  RadarSensor:1.OBJ_S_Range_58 : Outport  Port=885
  RadarSensor:1.OBJ_S_Range_59 : Outport  Port=886
  RadarSensor:1.OBJ_S_Range_60 : Outport  Port=887
  RadarSensor:1.OBJ_S_Range_61 : Outport  Port=888
  RadarSensor:1.OBJ_S_Range_62 : Outport  Port=889
  RadarSensor:1.OBJ_S_Range_63 : Outport  Port=890
  RadarSensor:1.OBJ_S_Range_64 : Outport  Port=891
  RadarSensor:1.OBJ_RCS : Outport  Port=892
  RadarSensor:1.OBJ_RCS_1 : Outport  Port=893
  RadarSensor:1.OBJ_RCS_2 : Outport  Port=894
  RadarSensor:1.OBJ_RCS_3 : Outport  Port=895
  RadarSensor:1.OBJ_RCS_4 : Outport  Port=896
  RadarSensor:1.OBJ_RCS_5 : Outport  Port=897
  RadarSensor:1.OBJ_RCS_6 : Outport  Port=898
  RadarSensor:1.OBJ_RCS_7 : Outport  Port=899
  RadarSensor:1.OBJ_RCS_8 : Outport  Port=900
  RadarSensor:1.OBJ_RCS_9 : Outport  Port=901
  RadarSensor:1.OBJ_RCS_10 : Outport  Port=902
  RadarSensor:1.OBJ_RCS_11 : Outport  Port=903
  RadarSensor:1.OBJ_RCS_12 : Outport  Port=904
  RadarSensor:1.OBJ_RCS_13 : Outport  Port=905
  RadarSensor:1.OBJ_RCS_14 : Outport  Port=906
  RadarSensor:1.OBJ_RCS_15 : Outport  Port=907
  RadarSensor:1.OBJ_RCS_16 : Outport  Port=908
  RadarSensor:1.OBJ_RCS_17 : Outport  Port=909
  RadarSensor:1.OBJ_RCS_18 : Outport  Port=910
  RadarSensor:1.OBJ_RCS_19 : Outport  Port=911
  RadarSensor:1.OBJ_RCS_20 : Outport  Port=912
  RadarSensor:1.OBJ_RCS_21 : Outport  Port=913
  RadarSensor:1.OBJ_RCS_22 : Outport  Port=914
  RadarSensor:1.OBJ_RCS_23 : Outport  Port=915
  RadarSensor:1.OBJ_RCS_24 : Outport  Port=916
  RadarSensor:1.OBJ_RCS_25 : Outport  Port=917
  RadarSensor:1.OBJ_RCS_26 : Outport  Port=918
  RadarSensor:1.OBJ_RCS_27 : Outport  Port=919
  RadarSensor:1.OBJ_RCS_28 : Outport  Port=920
  RadarSensor:1.OBJ_RCS_29 : Outport  Port=921
  RadarSensor:1.OBJ_RCS_30 : Outport  Port=922
  RadarSensor:1.OBJ_RCS_31 : Outport  Port=923
  RadarSensor:1.OBJ_RCS_32 : Outport  Port=924
  RadarSensor:1.OBJ_RCS_33 : Outport  Port=925
  RadarSensor:1.OBJ_RCS_34 : Outport  Port=926
  RadarSensor:1.OBJ_RCS_35 : Outport  Port=927
  RadarSensor:1.OBJ_RCS_36 : Outport  Port=928
  RadarSensor:1.OBJ_RCS_37 : Outport  Port=929
  RadarSensor:1.OBJ_RCS_38 : Outport  Port=930
  RadarSensor:1.OBJ_RCS_39 : Outport  Port=931
  RadarSensor:1.OBJ_RCS_40 : Outport  Port=932
  RadarSensor:1.OBJ_RCS_41 : Outport  Port=933
  RadarSensor:1.OBJ_RCS_42 : Outport  Port=934
  RadarSensor:1.OBJ_RCS_43 : Outport  Port=935
  RadarSensor:1.OBJ_RCS_44 : Outport  Port=936
  RadarSensor:1.OBJ_RCS_45 : Outport  Port=937
  RadarSensor:1.OBJ_RCS_46 : Outport  Port=938
  RadarSensor:1.OBJ_RCS_47 : Outport  Port=939
  RadarSensor:1.OBJ_RCS_48 : Outport  Port=940
  RadarSensor:1.OBJ_RCS_49 : Outport  Port=941
  RadarSensor:1.OBJ_RCS_50 : Outport  Port=942
  RadarSensor:1.OBJ_RCS_51 : Outport  Port=943
  RadarSensor:1.OBJ_RCS_52 : Outport  Port=944
  RadarSensor:1.OBJ_RCS_53 : Outport  Port=945
  RadarSensor:1.OBJ_RCS_54 : Outport  Port=946
  RadarSensor:1.OBJ_RCS_55 : Outport  Port=947
  RadarSensor:1.OBJ_RCS_56 : Outport  Port=948
  RadarSensor:1.OBJ_RCS_57 : Outport  Port=949
  RadarSensor:1.OBJ_RCS_58 : Outport  Port=950
  RadarSensor:1.OBJ_RCS_59 : Outport  Port=951
  RadarSensor:1.OBJ_RCS_60 : Outport  Port=952
  RadarSensor:1.OBJ_RCS_61 : Outport  Port=953
  RadarSensor:1.OBJ_RCS_62 : Outport  Port=954
  RadarSensor:1.OBJ_RCS_63 : Outport  Port=955
  RadarSensor:1.OBJ_RCS_64 : Outport  Port=956
  RadarSensor:2.time : Outport  Port=957
  RadarSensor:2.width : Outport  Port=958
  RadarSensor:2.OBJ_ID : Outport  Port=959
  RadarSensor:2.OBJ_ID_1 : Outport  Port=960
  RadarSensor:2.OBJ_ID_2 : Outport  Port=961
  RadarSensor:2.OBJ_ID_3 : Outport  Port=962
  RadarSensor:2.OBJ_ID_4 : Outport  Port=963
  RadarSensor:2.OBJ_ID_5 : Outport  Port=964
  RadarSensor:2.OBJ_ID_6 : Outport  Port=965
  RadarSensor:2.OBJ_ID_7 : Outport  Port=966
  RadarSensor:2.OBJ_ID_8 : Outport  Port=967
  RadarSensor:2.OBJ_ID_9 : Outport  Port=968
  RadarSensor:2.OBJ_ID_10 : Outport  Port=969
  RadarSensor:2.OBJ_ID_11 : Outport  Port=970
  RadarSensor:2.OBJ_ID_12 : Outport  Port=971
  RadarSensor:2.OBJ_ID_13 : Outport  Port=972
  RadarSensor:2.OBJ_ID_14 : Outport  Port=973
  RadarSensor:2.OBJ_ID_15 : Outport  Port=974
  RadarSensor:2.OBJ_ID_16 : Outport  Port=975
  RadarSensor:2.OBJ_ID_17 : Outport  Port=976
  RadarSensor:2.OBJ_ID_18 : Outport  Port=977
  RadarSensor:2.OBJ_ID_19 : Outport  Port=978
  RadarSensor:2.OBJ_ID_20 : Outport  Port=979
  RadarSensor:2.OBJ_ID_21 : Outport  Port=980
  RadarSensor:2.OBJ_ID_22 : Outport  Port=981
  RadarSensor:2.OBJ_ID_23 : Outport  Port=982
  RadarSensor:2.OBJ_ID_24 : Outport  Port=983
  RadarSensor:2.OBJ_ID_25 : Outport  Port=984
  RadarSensor:2.OBJ_ID_26 : Outport  Port=985
  RadarSensor:2.OBJ_ID_27 : Outport  Port=986
  RadarSensor:2.OBJ_ID_28 : Outport  Port=987
  RadarSensor:2.OBJ_ID_29 : Outport  Port=988
  RadarSensor:2.OBJ_ID_30 : Outport  Port=989
  RadarSensor:2.OBJ_ID_31 : Outport  Port=990
  RadarSensor:2.OBJ_ID_32 : Outport  Port=991
  RadarSensor:2.OBJ_ID_33 : Outport  Port=992
  RadarSensor:2.OBJ_ID_34 : Outport  Port=993
  RadarSensor:2.OBJ_ID_35 : Outport  Port=994
  RadarSensor:2.OBJ_ID_36 : Outport  Port=995
  RadarSensor:2.OBJ_ID_37 : Outport  Port=996
  RadarSensor:2.OBJ_ID_38 : Outport  Port=997
  RadarSensor:2.OBJ_ID_39 : Outport  Port=998
  RadarSensor:2.OBJ_ID_40 : Outport  Port=999
  RadarSensor:2.OBJ_ID_41 : Outport  Port=1000
  RadarSensor:2.OBJ_ID_42 : Outport  Port=1001
  RadarSensor:2.OBJ_ID_43 : Outport  Port=1002
  RadarSensor:2.OBJ_ID_44 : Outport  Port=1003
  RadarSensor:2.OBJ_ID_45 : Outport  Port=1004
  RadarSensor:2.OBJ_ID_46 : Outport  Port=1005
  RadarSensor:2.OBJ_ID_47 : Outport  Port=1006
  RadarSensor:2.OBJ_ID_48 : Outport  Port=1007
  RadarSensor:2.OBJ_ID_49 : Outport  Port=1008
  RadarSensor:2.OBJ_ID_50 : Outport  Port=1009
  RadarSensor:2.OBJ_ID_51 : Outport  Port=1010
  RadarSensor:2.OBJ_ID_52 : Outport  Port=1011
  RadarSensor:2.OBJ_ID_53 : Outport  Port=1012
  RadarSensor:2.OBJ_ID_54 : Outport  Port=1013
  RadarSensor:2.OBJ_ID_55 : Outport  Port=1014
  RadarSensor:2.OBJ_ID_56 : Outport  Port=1015
  RadarSensor:2.OBJ_ID_57 : Outport  Port=1016
  RadarSensor:2.OBJ_ID_58 : Outport  Port=1017
  RadarSensor:2.OBJ_ID_59 : Outport  Port=1018
  RadarSensor:2.OBJ_ID_60 : Outport  Port=1019
  RadarSensor:2.OBJ_ID_61 : Outport  Port=1020
  RadarSensor:2.OBJ_ID_62 : Outport  Port=1021
  RadarSensor:2.OBJ_ID_63 : Outport  Port=1022
  RadarSensor:2.OBJ_ID_64 : Outport  Port=1023
  RadarSensor:2.OBJ_Class : Outport  Port=1024
  RadarSensor:2.OBJ_Class_1 : Outport  Port=1025
  RadarSensor:2.OBJ_Class_2 : Outport  Port=1026
  RadarSensor:2.OBJ_Class_3 : Outport  Port=1027
  RadarSensor:2.OBJ_Class_4 : Outport  Port=1028
  RadarSensor:2.OBJ_Class_5 : Outport  Port=1029
  RadarSensor:2.OBJ_Class_6 : Outport  Port=1030
  RadarSensor:2.OBJ_Class_7 : Outport  Port=1031
  RadarSensor:2.OBJ_Class_8 : Outport  Port=1032
  RadarSensor:2.OBJ_Class_9 : Outport  Port=1033
  RadarSensor:2.OBJ_Class_10 : Outport  Port=1034
  RadarSensor:2.OBJ_Class_11 : Outport  Port=1035
  RadarSensor:2.OBJ_Class_12 : Outport  Port=1036
  RadarSensor:2.OBJ_Class_13 : Outport  Port=1037
  RadarSensor:2.OBJ_Class_14 : Outport  Port=1038
  RadarSensor:2.OBJ_Class_15 : Outport  Port=1039
  RadarSensor:2.OBJ_Class_16 : Outport  Port=1040
  RadarSensor:2.OBJ_Class_17 : Outport  Port=1041
  RadarSensor:2.OBJ_Class_18 : Outport  Port=1042
  RadarSensor:2.OBJ_Class_19 : Outport  Port=1043
  RadarSensor:2.OBJ_Class_20 : Outport  Port=1044
  RadarSensor:2.OBJ_Class_21 : Outport  Port=1045
  RadarSensor:2.OBJ_Class_22 : Outport  Port=1046
  RadarSensor:2.OBJ_Class_23 : Outport  Port=1047
  RadarSensor:2.OBJ_Class_24 : Outport  Port=1048
  RadarSensor:2.OBJ_Class_25 : Outport  Port=1049
  RadarSensor:2.OBJ_Class_26 : Outport  Port=1050
  RadarSensor:2.OBJ_Class_27 : Outport  Port=1051
  RadarSensor:2.OBJ_Class_28 : Outport  Port=1052
  RadarSensor:2.OBJ_Class_29 : Outport  Port=1053
  RadarSensor:2.OBJ_Class_30 : Outport  Port=1054
  RadarSensor:2.OBJ_Class_31 : Outport  Port=1055
  RadarSensor:2.OBJ_Class_32 : Outport  Port=1056
  RadarSensor:2.OBJ_Class_33 : Outport  Port=1057
  RadarSensor:2.OBJ_Class_34 : Outport  Port=1058
  RadarSensor:2.OBJ_Class_35 : Outport  Port=1059
  RadarSensor:2.OBJ_Class_36 : Outport  Port=1060
  RadarSensor:2.OBJ_Class_37 : Outport  Port=1061
  RadarSensor:2.OBJ_Class_38 : Outport  Port=1062
  RadarSensor:2.OBJ_Class_39 : Outport  Port=1063
  RadarSensor:2.OBJ_Class_40 : Outport  Port=1064
  RadarSensor:2.OBJ_Class_41 : Outport  Port=1065
  RadarSensor:2.OBJ_Class_42 : Outport  Port=1066
  RadarSensor:2.OBJ_Class_43 : Outport  Port=1067
  RadarSensor:2.OBJ_Class_44 : Outport  Port=1068
  RadarSensor:2.OBJ_Class_45 : Outport  Port=1069
  RadarSensor:2.OBJ_Class_46 : Outport  Port=1070
  RadarSensor:2.OBJ_Class_47 : Outport  Port=1071
  RadarSensor:2.OBJ_Class_48 : Outport  Port=1072
  RadarSensor:2.OBJ_Class_49 : Outport  Port=1073
  RadarSensor:2.OBJ_Class_50 : Outport  Port=1074
  RadarSensor:2.OBJ_Class_51 : Outport  Port=1075
  RadarSensor:2.OBJ_Class_52 : Outport  Port=1076
  RadarSensor:2.OBJ_Class_53 : Outport  Port=1077
  RadarSensor:2.OBJ_Class_54 : Outport  Port=1078
  RadarSensor:2.OBJ_Class_55 : Outport  Port=1079
  RadarSensor:2.OBJ_Class_56 : Outport  Port=1080
  RadarSensor:2.OBJ_Class_57 : Outport  Port=1081
  RadarSensor:2.OBJ_Class_58 : Outport  Port=1082
  RadarSensor:2.OBJ_Class_59 : Outport  Port=1083
  RadarSensor:2.OBJ_Class_60 : Outport  Port=1084
  RadarSensor:2.OBJ_Class_61 : Outport  Port=1085
  RadarSensor:2.OBJ_Class_62 : Outport  Port=1086
  RadarSensor:2.OBJ_Class_63 : Outport  Port=1087
  RadarSensor:2.OBJ_Class_64 : Outport  Port=1088
  RadarSensor:2.OBJ_S_Azimuth : Outport  Port=1089
  RadarSensor:2.OBJ_S_Azimuth_1 : Outport  Port=1090
  RadarSensor:2.OBJ_S_Azimuth_2 : Outport  Port=1091
  RadarSensor:2.OBJ_S_Azimuth_3 : Outport  Port=1092
  RadarSensor:2.OBJ_S_Azimuth_4 : Outport  Port=1093
  RadarSensor:2.OBJ_S_Azimuth_5 : Outport  Port=1094
  RadarSensor:2.OBJ_S_Azimuth_6 : Outport  Port=1095
  RadarSensor:2.OBJ_S_Azimuth_7 : Outport  Port=1096
  RadarSensor:2.OBJ_S_Azimuth_8 : Outport  Port=1097
  RadarSensor:2.OBJ_S_Azimuth_9 : Outport  Port=1098
  RadarSensor:2.OBJ_S_Azimuth_10 : Outport  Port=1099
  RadarSensor:2.OBJ_S_Azimuth_11 : Outport  Port=1100
  RadarSensor:2.OBJ_S_Azimuth_12 : Outport  Port=1101
  RadarSensor:2.OBJ_S_Azimuth_13 : Outport  Port=1102
  RadarSensor:2.OBJ_S_Azimuth_14 : Outport  Port=1103
  RadarSensor:2.OBJ_S_Azimuth_15 : Outport  Port=1104
  RadarSensor:2.OBJ_S_Azimuth_16 : Outport  Port=1105
  RadarSensor:2.OBJ_S_Azimuth_17 : Outport  Port=1106
  RadarSensor:2.OBJ_S_Azimuth_18 : Outport  Port=1107
  RadarSensor:2.OBJ_S_Azimuth_19 : Outport  Port=1108
  RadarSensor:2.OBJ_S_Azimuth_20 : Outport  Port=1109
  RadarSensor:2.OBJ_S_Azimuth_21 : Outport  Port=1110
  RadarSensor:2.OBJ_S_Azimuth_22 : Outport  Port=1111
  RadarSensor:2.OBJ_S_Azimuth_23 : Outport  Port=1112
  RadarSensor:2.OBJ_S_Azimuth_24 : Outport  Port=1113
  RadarSensor:2.OBJ_S_Azimuth_25 : Outport  Port=1114
  RadarSensor:2.OBJ_S_Azimuth_26 : Outport  Port=1115
  RadarSensor:2.OBJ_S_Azimuth_27 : Outport  Port=1116
  RadarSensor:2.OBJ_S_Azimuth_28 : Outport  Port=1117
  RadarSensor:2.OBJ_S_Azimuth_29 : Outport  Port=1118
  RadarSensor:2.OBJ_S_Azimuth_30 : Outport  Port=1119
  RadarSensor:2.OBJ_S_Azimuth_31 : Outport  Port=1120
  RadarSensor:2.OBJ_S_Azimuth_32 : Outport  Port=1121
  RadarSensor:2.OBJ_S_Azimuth_33 : Outport  Port=1122
  RadarSensor:2.OBJ_S_Azimuth_34 : Outport  Port=1123
  RadarSensor:2.OBJ_S_Azimuth_35 : Outport  Port=1124
  RadarSensor:2.OBJ_S_Azimuth_36 : Outport  Port=1125
  RadarSensor:2.OBJ_S_Azimuth_37 : Outport  Port=1126
  RadarSensor:2.OBJ_S_Azimuth_38 : Outport  Port=1127
  RadarSensor:2.OBJ_S_Azimuth_39 : Outport  Port=1128
  RadarSensor:2.OBJ_S_Azimuth_40 : Outport  Port=1129
  RadarSensor:2.OBJ_S_Azimuth_41 : Outport  Port=1130
  RadarSensor:2.OBJ_S_Azimuth_42 : Outport  Port=1131
  RadarSensor:2.OBJ_S_Azimuth_43 : Outport  Port=1132
  RadarSensor:2.OBJ_S_Azimuth_44 : Outport  Port=1133
  RadarSensor:2.OBJ_S_Azimuth_45 : Outport  Port=1134
  RadarSensor:2.OBJ_S_Azimuth_46 : Outport  Port=1135
  RadarSensor:2.OBJ_S_Azimuth_47 : Outport  Port=1136
  RadarSensor:2.OBJ_S_Azimuth_48 : Outport  Port=1137
  RadarSensor:2.OBJ_S_Azimuth_49 : Outport  Port=1138
  RadarSensor:2.OBJ_S_Azimuth_50 : Outport  Port=1139
  RadarSensor:2.OBJ_S_Azimuth_51 : Outport  Port=1140
  RadarSensor:2.OBJ_S_Azimuth_52 : Outport  Port=1141
  RadarSensor:2.OBJ_S_Azimuth_53 : Outport  Port=1142
  RadarSensor:2.OBJ_S_Azimuth_54 : Outport  Port=1143
  RadarSensor:2.OBJ_S_Azimuth_55 : Outport  Port=1144
  RadarSensor:2.OBJ_S_Azimuth_56 : Outport  Port=1145
  RadarSensor:2.OBJ_S_Azimuth_57 : Outport  Port=1146
  RadarSensor:2.OBJ_S_Azimuth_58 : Outport  Port=1147
  RadarSensor:2.OBJ_S_Azimuth_59 : Outport  Port=1148
  RadarSensor:2.OBJ_S_Azimuth_60 : Outport  Port=1149
  RadarSensor:2.OBJ_S_Azimuth_61 : Outport  Port=1150
  RadarSensor:2.OBJ_S_Azimuth_62 : Outport  Port=1151
  RadarSensor:2.OBJ_S_Azimuth_63 : Outport  Port=1152
  RadarSensor:2.OBJ_S_Azimuth_64 : Outport  Port=1153
  RadarSensor:2.OBJ_S_Elevation : Outport  Port=1154
  RadarSensor:2.OBJ_S_Elevation_1 : Outport  Port=1155
  RadarSensor:2.OBJ_S_Elevation_2 : Outport  Port=1156
  RadarSensor:2.OBJ_S_Elevation_3 : Outport  Port=1157
  RadarSensor:2.OBJ_S_Elevation_4 : Outport  Port=1158
  RadarSensor:2.OBJ_S_Elevation_5 : Outport  Port=1159
  RadarSensor:2.OBJ_S_Elevation_6 : Outport  Port=1160
  RadarSensor:2.OBJ_S_Elevation_7 : Outport  Port=1161
  RadarSensor:2.OBJ_S_Elevation_8 : Outport  Port=1162
  RadarSensor:2.OBJ_S_Elevation_9 : Outport  Port=1163
  RadarSensor:2.OBJ_S_Elevation_10 : Outport  Port=1164
  RadarSensor:2.OBJ_S_Elevation_11 : Outport  Port=1165
  RadarSensor:2.OBJ_S_Elevation_12 : Outport  Port=1166
  RadarSensor:2.OBJ_S_Elevation_13 : Outport  Port=1167
  RadarSensor:2.OBJ_S_Elevation_14 : Outport  Port=1168
  RadarSensor:2.OBJ_S_Elevation_15 : Outport  Port=1169
  RadarSensor:2.OBJ_S_Elevation_16 : Outport  Port=1170
  RadarSensor:2.OBJ_S_Elevation_17 : Outport  Port=1171
  RadarSensor:2.OBJ_S_Elevation_18 : Outport  Port=1172
  RadarSensor:2.OBJ_S_Elevation_19 : Outport  Port=1173
  RadarSensor:2.OBJ_S_Elevation_20 : Outport  Port=1174
  RadarSensor:2.OBJ_S_Elevation_21 : Outport  Port=1175
  RadarSensor:2.OBJ_S_Elevation_22 : Outport  Port=1176
  RadarSensor:2.OBJ_S_Elevation_23 : Outport  Port=1177
  RadarSensor:2.OBJ_S_Elevation_24 : Outport  Port=1178
  RadarSensor:2.OBJ_S_Elevation_25 : Outport  Port=1179
  RadarSensor:2.OBJ_S_Elevation_26 : Outport  Port=1180
  RadarSensor:2.OBJ_S_Elevation_27 : Outport  Port=1181
  RadarSensor:2.OBJ_S_Elevation_28 : Outport  Port=1182
  RadarSensor:2.OBJ_S_Elevation_29 : Outport  Port=1183
  RadarSensor:2.OBJ_S_Elevation_30 : Outport  Port=1184
  RadarSensor:2.OBJ_S_Elevation_31 : Outport  Port=1185
  RadarSensor:2.OBJ_S_Elevation_32 : Outport  Port=1186
  RadarSensor:2.OBJ_S_Elevation_33 : Outport  Port=1187
  RadarSensor:2.OBJ_S_Elevation_34 : Outport  Port=1188
  RadarSensor:2.OBJ_S_Elevation_35 : Outport  Port=1189
  RadarSensor:2.OBJ_S_Elevation_36 : Outport  Port=1190
  RadarSensor:2.OBJ_S_Elevation_37 : Outport  Port=1191
  RadarSensor:2.OBJ_S_Elevation_38 : Outport  Port=1192
  RadarSensor:2.OBJ_S_Elevation_39 : Outport  Port=1193
  RadarSensor:2.OBJ_S_Elevation_40 : Outport  Port=1194
  RadarSensor:2.OBJ_S_Elevation_41 : Outport  Port=1195
  RadarSensor:2.OBJ_S_Elevation_42 : Outport  Port=1196
  RadarSensor:2.OBJ_S_Elevation_43 : Outport  Port=1197
  RadarSensor:2.OBJ_S_Elevation_44 : Outport  Port=1198
  RadarSensor:2.OBJ_S_Elevation_45 : Outport  Port=1199
  RadarSensor:2.OBJ_S_Elevation_46 : Outport  Port=1200
  RadarSensor:2.OBJ_S_Elevation_47 : Outport  Port=1201
  RadarSensor:2.OBJ_S_Elevation_48 : Outport  Port=1202
  RadarSensor:2.OBJ_S_Elevation_49 : Outport  Port=1203
  RadarSensor:2.OBJ_S_Elevation_50 : Outport  Port=1204
  RadarSensor:2.OBJ_S_Elevation_51 : Outport  Port=1205
  RadarSensor:2.OBJ_S_Elevation_52 : Outport  Port=1206
  RadarSensor:2.OBJ_S_Elevation_53 : Outport  Port=1207
  RadarSensor:2.OBJ_S_Elevation_54 : Outport  Port=1208
  RadarSensor:2.OBJ_S_Elevation_55 : Outport  Port=1209
  RadarSensor:2.OBJ_S_Elevation_56 : Outport  Port=1210
  RadarSensor:2.OBJ_S_Elevation_57 : Outport  Port=1211
  RadarSensor:2.OBJ_S_Elevation_58 : Outport  Port=1212
  RadarSensor:2.OBJ_S_Elevation_59 : Outport  Port=1213
  RadarSensor:2.OBJ_S_Elevation_60 : Outport  Port=1214
  RadarSensor:2.OBJ_S_Elevation_61 : Outport  Port=1215
  RadarSensor:2.OBJ_S_Elevation_62 : Outport  Port=1216
  RadarSensor:2.OBJ_S_Elevation_63 : Outport  Port=1217
  RadarSensor:2.OBJ_S_Elevation_64 : Outport  Port=1218
  RadarSensor:2.OBJ_S_Velocity : Outport  Port=1219
  RadarSensor:2.OBJ_S_Velocity_1 : Outport  Port=1220
  RadarSensor:2.OBJ_S_Velocity_2 : Outport  Port=1221
  RadarSensor:2.OBJ_S_Velocity_3 : Outport  Port=1222
  RadarSensor:2.OBJ_S_Velocity_4 : Outport  Port=1223
  RadarSensor:2.OBJ_S_Velocity_5 : Outport  Port=1224
  RadarSensor:2.OBJ_S_Velocity_6 : Outport  Port=1225
  RadarSensor:2.OBJ_S_Velocity_7 : Outport  Port=1226
  RadarSensor:2.OBJ_S_Velocity_8 : Outport  Port=1227
  RadarSensor:2.OBJ_S_Velocity_9 : Outport  Port=1228
  RadarSensor:2.OBJ_S_Velocity_10 : Outport  Port=1229
  RadarSensor:2.OBJ_S_Velocity_11 : Outport  Port=1230
  RadarSensor:2.OBJ_S_Velocity_12 : Outport  Port=1231
  RadarSensor:2.OBJ_S_Velocity_13 : Outport  Port=1232
  RadarSensor:2.OBJ_S_Velocity_14 : Outport  Port=1233
  RadarSensor:2.OBJ_S_Velocity_15 : Outport  Port=1234
  RadarSensor:2.OBJ_S_Velocity_16 : Outport  Port=1235
  RadarSensor:2.OBJ_S_Velocity_17 : Outport  Port=1236
  RadarSensor:2.OBJ_S_Velocity_18 : Outport  Port=1237
  RadarSensor:2.OBJ_S_Velocity_19 : Outport  Port=1238
  RadarSensor:2.OBJ_S_Velocity_20 : Outport  Port=1239
  RadarSensor:2.OBJ_S_Velocity_21 : Outport  Port=1240
  RadarSensor:2.OBJ_S_Velocity_22 : Outport  Port=1241
  RadarSensor:2.OBJ_S_Velocity_23 : Outport  Port=1242
  RadarSensor:2.OBJ_S_Velocity_24 : Outport  Port=1243
  RadarSensor:2.OBJ_S_Velocity_25 : Outport  Port=1244
  RadarSensor:2.OBJ_S_Velocity_26 : Outport  Port=1245
  RadarSensor:2.OBJ_S_Velocity_27 : Outport  Port=1246
  RadarSensor:2.OBJ_S_Velocity_28 : Outport  Port=1247
  RadarSensor:2.OBJ_S_Velocity_29 : Outport  Port=1248
  RadarSensor:2.OBJ_S_Velocity_30 : Outport  Port=1249
  RadarSensor:2.OBJ_S_Velocity_31 : Outport  Port=1250
  RadarSensor:2.OBJ_S_Velocity_32 : Outport  Port=1251
  RadarSensor:2.OBJ_S_Velocity_33 : Outport  Port=1252
  RadarSensor:2.OBJ_S_Velocity_34 : Outport  Port=1253
  RadarSensor:2.OBJ_S_Velocity_35 : Outport  Port=1254
  RadarSensor:2.OBJ_S_Velocity_36 : Outport  Port=1255
  RadarSensor:2.OBJ_S_Velocity_37 : Outport  Port=1256
  RadarSensor:2.OBJ_S_Velocity_38 : Outport  Port=1257
  RadarSensor:2.OBJ_S_Velocity_39 : Outport  Port=1258
  RadarSensor:2.OBJ_S_Velocity_40 : Outport  Port=1259
  RadarSensor:2.OBJ_S_Velocity_41 : Outport  Port=1260
  RadarSensor:2.OBJ_S_Velocity_42 : Outport  Port=1261
  RadarSensor:2.OBJ_S_Velocity_43 : Outport  Port=1262
  RadarSensor:2.OBJ_S_Velocity_44 : Outport  Port=1263
  RadarSensor:2.OBJ_S_Velocity_45 : Outport  Port=1264
  RadarSensor:2.OBJ_S_Velocity_46 : Outport  Port=1265
  RadarSensor:2.OBJ_S_Velocity_47 : Outport  Port=1266
  RadarSensor:2.OBJ_S_Velocity_48 : Outport  Port=1267
  RadarSensor:2.OBJ_S_Velocity_49 : Outport  Port=1268
  RadarSensor:2.OBJ_S_Velocity_50 : Outport  Port=1269
  RadarSensor:2.OBJ_S_Velocity_51 : Outport  Port=1270
  RadarSensor:2.OBJ_S_Velocity_52 : Outport  Port=1271
  RadarSensor:2.OBJ_S_Velocity_53 : Outport  Port=1272
  RadarSensor:2.OBJ_S_Velocity_54 : Outport  Port=1273
  RadarSensor:2.OBJ_S_Velocity_55 : Outport  Port=1274
  RadarSensor:2.OBJ_S_Velocity_56 : Outport  Port=1275
  RadarSensor:2.OBJ_S_Velocity_57 : Outport  Port=1276
  RadarSensor:2.OBJ_S_Velocity_58 : Outport  Port=1277
  RadarSensor:2.OBJ_S_Velocity_59 : Outport  Port=1278
  RadarSensor:2.OBJ_S_Velocity_60 : Outport  Port=1279
  RadarSensor:2.OBJ_S_Velocity_61 : Outport  Port=1280
  RadarSensor:2.OBJ_S_Velocity_62 : Outport  Port=1281
  RadarSensor:2.OBJ_S_Velocity_63 : Outport  Port=1282
  RadarSensor:2.OBJ_S_Velocity_64 : Outport  Port=1283
  RadarSensor:2.OBJ_S_Range : Outport  Port=1284
  RadarSensor:2.OBJ_S_Range_1 : Outport  Port=1285
  RadarSensor:2.OBJ_S_Range_2 : Outport  Port=1286
  RadarSensor:2.OBJ_S_Range_3 : Outport  Port=1287
  RadarSensor:2.OBJ_S_Range_4 : Outport  Port=1288
  RadarSensor:2.OBJ_S_Range_5 : Outport  Port=1289
  RadarSensor:2.OBJ_S_Range_6 : Outport  Port=1290
  RadarSensor:2.OBJ_S_Range_7 : Outport  Port=1291
  RadarSensor:2.OBJ_S_Range_8 : Outport  Port=1292
  RadarSensor:2.OBJ_S_Range_9 : Outport  Port=1293
  RadarSensor:2.OBJ_S_Range_10 : Outport  Port=1294
  RadarSensor:2.OBJ_S_Range_11 : Outport  Port=1295
  RadarSensor:2.OBJ_S_Range_12 : Outport  Port=1296
  RadarSensor:2.OBJ_S_Range_13 : Outport  Port=1297
  RadarSensor:2.OBJ_S_Range_14 : Outport  Port=1298
  RadarSensor:2.OBJ_S_Range_15 : Outport  Port=1299
  RadarSensor:2.OBJ_S_Range_16 : Outport  Port=1300
  RadarSensor:2.OBJ_S_Range_17 : Outport  Port=1301
  RadarSensor:2.OBJ_S_Range_18 : Outport  Port=1302
  RadarSensor:2.OBJ_S_Range_19 : Outport  Port=1303
  RadarSensor:2.OBJ_S_Range_20 : Outport  Port=1304
  RadarSensor:2.OBJ_S_Range_21 : Outport  Port=1305
  RadarSensor:2.OBJ_S_Range_22 : Outport  Port=1306
  RadarSensor:2.OBJ_S_Range_23 : Outport  Port=1307
  RadarSensor:2.OBJ_S_Range_24 : Outport  Port=1308
  RadarSensor:2.OBJ_S_Range_25 : Outport  Port=1309
  RadarSensor:2.OBJ_S_Range_26 : Outport  Port=1310
  RadarSensor:2.OBJ_S_Range_27 : Outport  Port=1311
  RadarSensor:2.OBJ_S_Range_28 : Outport  Port=1312
  RadarSensor:2.OBJ_S_Range_29 : Outport  Port=1313
  RadarSensor:2.OBJ_S_Range_30 : Outport  Port=1314
  RadarSensor:2.OBJ_S_Range_31 : Outport  Port=1315
  RadarSensor:2.OBJ_S_Range_32 : Outport  Port=1316
  RadarSensor:2.OBJ_S_Range_33 : Outport  Port=1317
  RadarSensor:2.OBJ_S_Range_34 : Outport  Port=1318
  RadarSensor:2.OBJ_S_Range_35 : Outport  Port=1319
  RadarSensor:2.OBJ_S_Range_36 : Outport  Port=1320
  RadarSensor:2.OBJ_S_Range_37 : Outport  Port=1321
  RadarSensor:2.OBJ_S_Range_38 : Outport  Port=1322
  RadarSensor:2.OBJ_S_Range_39 : Outport  Port=1323
  RadarSensor:2.OBJ_S_Range_40 : Outport  Port=1324
  RadarSensor:2.OBJ_S_Range_41 : Outport  Port=1325
  RadarSensor:2.OBJ_S_Range_42 : Outport  Port=1326
  RadarSensor:2.OBJ_S_Range_43 : Outport  Port=1327
  RadarSensor:2.OBJ_S_Range_44 : Outport  Port=1328
  RadarSensor:2.OBJ_S_Range_45 : Outport  Port=1329
  RadarSensor:2.OBJ_S_Range_46 : Outport  Port=1330
  RadarSensor:2.OBJ_S_Range_47 : Outport  Port=1331
  RadarSensor:2.OBJ_S_Range_48 : Outport  Port=1332
  RadarSensor:2.OBJ_S_Range_49 : Outport  Port=1333
  RadarSensor:2.OBJ_S_Range_50 : Outport  Port=1334
